simulink model "model"  (R2014a)
(part 4 of 5)

  С_10_С_85_(ПС_«Восточная»___ПС_«Солнечная»___ПС_«Зональная»___ПС_«Солнечная»)_CN_131640871_110000_CN_161501791_110000/RConn3 -- T_161501791_110000_Подстанция_«Коммунальная»/LConn3 -- bus34/LConn1
  T_223481385__Тяговая_ПС/LConn1 -- _CN_223481385_110000_CN_208172439_110000/LConn1
  T_223481385__Тяговая_ПС/LConn2 -- _CN_223481385_110000_CN_208172439_110000/LConn2
  _CN_223481385_110000_CN_208172439_110000/LConn3 -- T_223481385__Тяговая_ПС/LConn3 -- bus35/LConn1
  _CN_223481385_110000_CN_208172439_110000/RConn1 -- T_208172439_110000_Яшкино/LConn1 -- _CN_202917769_110000_CN_208172439_110000/LConn1
  _CN_223481385_110000_CN_208172439_110000/RConn2 -- T_208172439_110000_Яшкино/LConn2 -- _CN_202917769_110000_CN_208172439_110000/LConn2
  _CN_223481385_110000_CN_208172439_110000/RConn3 -- T_208172439_110000_Яшкино/LConn3 -- _CN_202917769_110000_CN_208172439_110000/LConn3 -- bus36/LConn1
  "T_237781034__ПС_110_10_кВ_\"Стрела\""/LConn1 -- _CN_237781034_110000_CN_421135596_110000/LConn1
  "T_237781034__ПС_110_10_кВ_\"Стрела\""/LConn2 -- _CN_237781034_110000_CN_421135596_110000/LConn2
  _CN_237781034_110000_CN_421135596_110000/LConn3 -- "T_237781034__ПС_110_10_кВ_\"Стрела\""/LConn3 -- bus37/LConn1
  "T_421135596_110000;35000;10000_ПС_\"Новоуральская\"_110_35_10"/LConn1 -- _CN_237781034_110000_CN_421135596_110000/RConn1
  "T_421135596_110000;35000;10000_ПС_\"Новоуральская\"_110_35_10"/LConn2 -- _CN_237781034_110000_CN_421135596_110000/RConn2
  _CN_237781034_110000_CN_421135596_110000/RConn3 -- "T_421135596_110000;35000;10000_ПС_\"Новоуральская\"_110_35_10"/LConn3 -- bus38/LConn1
  _CN_228962860_110000_CN_418072303_110000/LConn1 -- T_228962860__/LConn1 -- _CN_228962860_110000_CN_180788791_110000/LConn1
  _CN_228962860_110000_CN_418072303_110000/LConn2 -- T_228962860__/LConn2 -- _CN_228962860_110000_CN_180788791_110000/LConn2
  _CN_228962860_110000_CN_418072303_110000/LConn3 -- T_228962860__/LConn3 -- _CN_228962860_110000_CN_180788791_110000/LConn3 -- bus39/LConn1
  T_418072303__/LConn1 -- _CN_228962860_110000_CN_418072303_110000/RConn1
  T_418072303__/LConn2 -- _CN_228962860_110000_CN_418072303_110000/RConn2
  _CN_228962860_110000_CN_418072303_110000/RConn3 -- T_418072303__/LConn3 -- bus40/LConn1
  _CN_228962860_110000_CN_180788791_110000/RConn1 -- T_180788791__/LConn1 -- _CN_168239171_110000_CN_180788791_110000/LConn1
  _CN_228962860_110000_CN_180788791_110000/RConn2 -- T_180788791__/LConn2 -- _CN_168239171_110000_CN_180788791_110000/LConn2
  _CN_228962860_110000_CN_180788791_110000/RConn3 -- T_180788791__/LConn3 -- _CN_168239171_110000_CN_180788791_110000/LConn3 -- bus41/LConn1
  "T_178541618_110000;6000_ПС_№119_\"Мичуринская\""/LConn1 -- С_201___С_202_CN_178541618_110000_CN_130661477_110000/LConn1
  "T_178541618_110000;6000_ПС_№119_\"Мичуринская\""/LConn2 -- С_201___С_202_CN_178541618_110000_CN_130661477_110000/LConn2
  С_201___С_202_CN_178541618_110000_CN_130661477_110000/LConn3 -- "T_178541618_110000;6000_ПС_№119_\"Мичуринская\""/LConn3 -- bus42/LConn1
  С_201___С_202_CN_178541618_110000_CN_130661477_110000/RConn1 -- G_130661477_Красноярская_ТЭЦ_1/RConn1 -- С_1___С_204_CN_435735618_110000_CN_130661477_110000/RConn1 -- _CN_259523001_110000_CN_130661477_110000/LConn1 -- _CN_259526393_110000_CN_130661477_110000/LConn1
  С_201___С_202_CN_178541618_110000_CN_130661477_110000/RConn2 -- G_130661477_Красноярская_ТЭЦ_1/RConn2 -- С_1___С_204_CN_435735618_110000_CN_130661477_110000/RConn2 -- _CN_259523001_110000_CN_130661477_110000/LConn2 -- _CN_259526393_110000_CN_130661477_110000/LConn2
  С_201___С_202_CN_178541618_110000_CN_130661477_110000/RConn3 -- G_130661477_Красноярская_ТЭЦ_1/RConn3 -- С_1___С_204_CN_435735618_110000_CN_130661477_110000/RConn3 -- _CN_259523001_110000_CN_130661477_110000/LConn3 -- _CN_259526393_110000_CN_130661477_110000/LConn3 -- bus43/LConn1
  T_201587851__/LConn1 -- _CN_201587851_110000_CN_98731668_110000/LConn1
  T_201587851__/LConn2 -- _CN_201587851_110000_CN_98731668_110000/LConn2
  _CN_201587851_110000_CN_98731668_110000/LConn3 -- T_201587851__/LConn3 -- bus44/LConn1
  T_98731668_220000_Подстанция_«Районная»/LConn1 -- _CN_201587851_110000_CN_98731668_110000/RConn1
  T_98731668_220000_Подстанция_«Районная»/LConn2 -- _CN_201587851_110000_CN_98731668_110000/RConn2
  _CN_201587851_110000_CN_98731668_110000/RConn3 -- T_98731668_220000_Подстанция_«Районная»/LConn3 -- bus45/LConn1
  _CN_110796857_110000_CN_184811446_110000/LConn1 -- "T_110796857__ПС_500_220_110_кВ_\"Иркутская\""/RConn1 -- _CN_110796857_110000_CN_184798669_110000/LConn1 -- L_110796857/LConn1
  _CN_110796857_110000_CN_184811446_110000/LConn2 -- "T_110796857__ПС_500_220_110_кВ_\"Иркутская\""/RConn2 -- _CN_110796857_110000_CN_184798669_110000/LConn2 -- L_110796857/LConn2
  _CN_110796857_110000_CN_184811446_110000/LConn3 -- "T_110796857__ПС_500_220_110_кВ_\"Иркутская\""/RConn3 -- _CN_110796857_110000_CN_184798669_110000/LConn3 -- L_110796857/LConn3 -- bus46/LConn1
  T_184811446_110000_ПС_110_35_6_кВ_Прибрежная/LConn1 -- _CN_110796857_110000_CN_184811446_110000/RConn1
  T_184811446_110000_ПС_110_35_6_кВ_Прибрежная/LConn2 -- _CN_110796857_110000_CN_184811446_110000/RConn2
  _CN_110796857_110000_CN_184811446_110000/RConn3 -- T_184811446_110000_ПС_110_35_6_кВ_Прибрежная/LConn3 -- bus47/LConn1
  _CN_110796857_110000_CN_184798669_110000/RConn1 -- T_184798669__ПС_110_35_6_кВ_ГПП_2/LConn1 -- _CN_184798669_110000_CN_297714701_110000/LConn1
  _CN_110796857_110000_CN_184798669_110000/RConn2 -- T_184798669__ПС_110_35_6_кВ_ГПП_2/LConn2 -- _CN_184798669_110000_CN_297714701_110000/LConn2
  _CN_110796857_110000_CN_184798669_110000/RConn3 -- T_184798669__ПС_110_35_6_кВ_ГПП_2/LConn3 -- _CN_184798669_110000_CN_297714701_110000/LConn3 -- bus48/LConn1
  _CN_283922783_110000_CN_202649908_110000/LConn1 -- "T_283922783_110000;10000_ПС_№122_\"Северная\""/LConn1 -- _CN_283922783_110000_CN_95996044_110000/LConn1 -- _CN_283922783_110000_CN_225106390_110000/LConn1 -- _CN_283922783_110000_CN_95614050_110000/LConn1
  _CN_283922783_110000_CN_202649908_110000/LConn2 -- "T_283922783_110000;10000_ПС_№122_\"Северная\""/LConn2 -- _CN_283922783_110000_CN_95996044_110000/LConn2 -- _CN_283922783_110000_CN_225106390_110000/LConn2 -- _CN_283922783_110000_CN_95614050_110000/LConn2
  _CN_283922783_110000_CN_202649908_110000/LConn3 -- "T_283922783_110000;10000_ПС_№122_\"Северная\""/LConn3 -- _CN_283922783_110000_CN_95996044_110000/LConn3 -- _CN_283922783_110000_CN_225106390_110000/LConn3 -- _CN_283922783_110000_CN_95614050_110000/LConn3 -- bus49/LConn1
  _CN_283922783_110000_CN_202649908_110000/RConn1 -- "T_202649908_220000;110000;10000_ПС_\"Октябрьская\""/RConn1 -- С_17___С_18_CN_255772238_110000_CN_202649908_110000/LConn1 -- С_13___С_14_CN_267632930_110000_CN_202649908_110000/LConn1 -- L_202649908/LConn1
  _CN_283922783_110000_CN_202649908_110000/RConn2 -- "T_202649908_220000;110000;10000_ПС_\"Октябрьская\""/RConn2 -- С_17___С_18_CN_255772238_110000_CN_202649908_110000/LConn2 -- С_13___С_14_CN_267632930_110000_CN_202649908_110000/LConn2 -- L_202649908/LConn2
  _CN_283922783_110000_CN_202649908_110000/RConn3 -- "T_202649908_220000;110000;10000_ПС_\"Октябрьская\""/RConn3 -- С_17___С_18_CN_255772238_110000_CN_202649908_110000/LConn3 -- С_13___С_14_CN_267632930_110000_CN_202649908_110000/LConn3 -- L_202649908/LConn3 -- bus50/LConn1
  _CN_283922783_110000_CN_95996044_110000/RConn1 -- "T_95996044_220000;110000;10000_ПС_\"Левобережная\""/RConn1 -- _CN_95996044_110000_CN_289000622_110000/LConn1 -- _CN_95996044_110000_CN_203496562_110000/RConn1 -- L_95996044/LConn1 -- _CN_277861487_110000_CN_95996044_110000/LConn1
  _CN_283922783_110000_CN_95996044_110000/RConn2 -- "T_95996044_220000;110000;10000_ПС_\"Левобережная\""/RConn2 -- _CN_95996044_110000_CN_289000622_110000/LConn2 -- _CN_95996044_110000_CN_203496562_110000/RConn2 -- L_95996044/LConn2 -- _CN_277861487_110000_CN_95996044_110000/LConn2
  _CN_283922783_110000_CN_95996044_110000/RConn3 -- "T_95996044_220000;110000;10000_ПС_\"Левобережная\""/RConn3 -- _CN_95996044_110000_CN_289000622_110000/LConn3 -- _CN_95996044_110000_CN_203496562_110000/RConn3 -- L_95996044/LConn3 -- bus51/LConn1 -- _CN_277861487_110000_CN_95996044_110000/LConn3
  "T_225106390_110000;10000_ПС_№140_\"Аэропорт\""/LConn1 -- _CN_283922783_110000_CN_225106390_110000/RConn1
  "T_225106390_110000;10000_ПС_№140_\"Аэропорт\""/LConn2 -- _CN_283922783_110000_CN_225106390_110000/RConn2
  _CN_283922783_110000_CN_225106390_110000/RConn3 -- "T_225106390_110000;10000_ПС_№140_\"Аэропорт\""/LConn3 -- bus52/LConn1
  T_95614050_110000;10000_/LConn1 -- _CN_283922783_110000_CN_95614050_110000/RConn1
  T_95614050_110000;10000_/LConn2 -- _CN_283922783_110000_CN_95614050_110000/RConn2
  _CN_283922783_110000_CN_95614050_110000/RConn3 -- T_95614050_110000;10000_/LConn3 -- bus53/LConn1
  "T_255519517_110000;6000_ПС_\"Химволокно\""/LConn1 -- С_221___С_222_CN_435735618_110000_CN_255519517_110000/RConn1
  "T_255519517_110000;6000_ПС_\"Химволокно\""/LConn2 -- С_221___С_222_CN_435735618_110000_CN_255519517_110000/RConn2
  С_221___С_222_CN_435735618_110000_CN_255519517_110000/RConn3 -- "T_255519517_110000;6000_ПС_\"Химволокно\""/LConn3 -- bus54/LConn1
  "T_255519515_110000;6000_ПС_\"Цветные_металлы\""/LConn1 -- С_221___С_222_CN_435735618_110000_CN_255519515_110000/RConn1
  "T_255519515_110000;6000_ПС_\"Цветные_металлы\""/LConn2 -- С_221___С_222_CN_435735618_110000_CN_255519515_110000/RConn2
  С_221___С_222_CN_435735618_110000_CN_255519515_110000/RConn3 -- "T_255519515_110000;6000_ПС_\"Цветные_металлы\""/LConn3 -- bus55/LConn1
  "T_258257783_110000;10000_ПС_ГПП_1_\"КрасМаш\""/LConn1 -- С_1___С_204_CN_435735618_110000_CN_258257783_110000/RConn1
  "T_258257783_110000;10000_ПС_ГПП_1_\"КрасМаш\""/LConn2 -- С_1___С_204_CN_435735618_110000_CN_258257783_110000/RConn2
  С_1___С_204_CN_435735618_110000_CN_258257783_110000/RConn3 -- "T_258257783_110000;10000_ПС_ГПП_1_\"КрасМаш\""/LConn3 -- bus56/LConn1
  "T_328318277_110000;10000_ПС_ГПП_2_\"КрасМаш\""/LConn1 -- С_1___С_204_CN_435735618_110000_CN_328318277_110000/RConn1
  "T_328318277_110000;10000_ПС_ГПП_2_\"КрасМаш\""/LConn2 -- С_1___С_204_CN_435735618_110000_CN_328318277_110000/RConn2
  С_1___С_204_CN_435735618_110000_CN_328318277_110000/RConn3 -- "T_328318277_110000;10000_ПС_ГПП_2_\"КрасМаш\""/LConn3 -- bus57/LConn1
  T_255181608_110000_/LConn1 -- _CN_435735618_110000_CN_255181608_110000/RConn1
  T_255181608_110000_/LConn2 -- _CN_435735618_110000_CN_255181608_110000/RConn2
  _CN_435735618_110000_CN_255181608_110000/RConn3 -- T_255181608_110000_/LConn3 -- bus58/LConn1
  _CN_168239171_110000_CN_180788791_110000/RConn1 -- T_168239171_220000_Подстанция_«Ужур»/RConn1 -- L_168239171/LConn1
  _CN_168239171_110000_CN_180788791_110000/RConn2 -- T_168239171_220000_Подстанция_«Ужур»/RConn2 -- L_168239171/LConn2
  _CN_168239171_110000_CN_180788791_110000/RConn3 -- T_168239171_220000_Подстанция_«Ужур»/RConn3 -- L_168239171/LConn3 -- bus59/LConn1
  "T_201620593_110000_Тяговая_ПС_\"Кабаклы\""/LConn1 -- _CN_107439685_110000_CN_201620593_110000/RConn1
  "T_201620593_110000_Тяговая_ПС_\"Кабаклы\""/LConn2 -- _CN_107439685_110000_CN_201620593_110000/RConn2
  _CN_107439685_110000_CN_201620593_110000/RConn3 -- "T_201620593_110000_Тяговая_ПС_\"Кабаклы\""/LConn3 -- bus60/LConn1
  T_197934973_110000_Подстанция_«Валерино»/LConn1 -- _CN_107439685_110000_CN_197934973_110000/RConn1
  T_197934973_110000_Подстанция_«Валерино»/LConn2 -- _CN_107439685_110000_CN_197934973_110000/RConn2
  _CN_107439685_110000_CN_197934973_110000/RConn3 -- T_197934973_110000_Подстанция_«Валерино»/LConn3 -- bus61/LConn1
  T_113306036__/LConn1 -- _CN_107439685_110000_CN_113306036_110000/RConn1
  T_113306036__/LConn2 -- _CN_107439685_110000_CN_113306036_110000/RConn2
  _CN_107439685_110000_CN_113306036_110000/RConn3 -- T_113306036__/LConn3 -- bus62/LConn1
  T_197933918_110000_/LConn1 -- _CN_107439685_110000_CN_197933918_110000/RConn1
  T_197933918_110000_/LConn2 -- _CN_107439685_110000_CN_197933918_110000/RConn2
  _CN_107439685_110000_CN_197933918_110000/RConn3 -- T_197933918_110000_/LConn3 -- bus63/LConn1
  T_201620594_110000_Подстанция_«Киевская»/LConn1 -- _CN_107439685_110000_CN_201620594_110000/RConn1
  T_201620594_110000_Подстанция_«Киевская»/LConn2 -- _CN_107439685_110000_CN_201620594_110000/RConn2
  _CN_107439685_110000_CN_201620594_110000/RConn3 -- T_201620594_110000_Подстанция_«Киевская»/LConn3 -- bus64/LConn1
  С_15_С_16_(ПС_«Левобережная»___ПС_«Мельниково_110»)_CN_167347786_110000_CN_150289682_110000/LConn1 -- T_167347786_110000_Подстанция_«Мельниково»/LConn1 -- С_18_(ПС_«Мельниково»___ПС_«Кожевниково»)_CN_167347786_110000_CN_169673998_110000/LConn1
  С_15_С_16_(ПС_«Левобережная»___ПС_«Мельниково_110»)_CN_167347786_110000_CN_150289682_110000/LConn2 -- T_167347786_110000_Подстанция_«Мельниково»/LConn2 -- С_18_(ПС_«Мельниково»___ПС_«Кожевниково»)_CN_167347786_110000_CN_169673998_110000/LConn2
  С_15_С_16_(ПС_«Левобережная»___ПС_«Мельниково_110»)_CN_167347786_110000_CN_150289682_110000/LConn3 -- T_167347786_110000_Подстанция_«Мельниково»/LConn3 -- С_18_(ПС_«Мельниково»___ПС_«Кожевниково»)_CN_167347786_110000_CN_169673998_110000/LConn3 -- bus65/LConn1
  С_15_С_16_(ПС_«Левобережная»___ПС_«Мельниково_110»)_CN_167347786_110000_CN_150289682_110000/RConn1 -- T_150289682_110000_Подстанция_«Левобережная»/LConn1 -- С_82_С_83_(ПС_«Зональная»___ПС_«Левобережная»)_CN_123874057_110000_CN_150289682_110000/RConn1 -- С_13_С_14_(ПС_«Левобережная»___ПС_«Кандинка_110»)_CN_150289682_110000_CN_169996149_110000/LConn1
  С_15_С_16_(ПС_«Левобережная»___ПС_«Мельниково_110»)_CN_167347786_110000_CN_150289682_110000/RConn2 -- T_150289682_110000_Подстанция_«Левобережная»/LConn2 -- С_82_С_83_(ПС_«Зональная»___ПС_«Левобережная»)_CN_123874057_110000_CN_150289682_110000/RConn2 -- С_13_С_14_(ПС_«Левобережная»___ПС_«Кандинка_110»)_CN_150289682_110000_CN_169996149_110000/LConn2
  С_15_С_16_(ПС_«Левобережная»___ПС_«Мельниково_110»)_CN_167347786_110000_CN_150289682_110000/RConn3 -- T_150289682_110000_Подстанция_«Левобережная»/LConn3 -- С_82_С_83_(ПС_«Зональная»___ПС_«Левобережная»)_CN_123874057_110000_CN_150289682_110000/RConn3 -- С_13_С_14_(ПС_«Левобережная»___ПС_«Кандинка_110»)_CN_150289682_110000_CN_169996149_110000/LConn3 -- bus66/LConn1
  С_18_(ПС_«Мельниково»___ПС_«Кожевниково»)_CN_167347786_110000_CN_169673998_110000/RConn1 -- T_169673998_110000_Подстанция_«Кожевниково»/LConn1 -- С_19_(ПС_«Кожевниково»___ПС_«Уртам»)_CN_169673998_110000_CN_165976042_110000/RConn1
  С_18_(ПС_«Мельниково»___ПС_«Кожевниково»)_CN_167347786_110000_CN_169673998_110000/RConn2 -- T_169673998_110000_Подстанция_«Кожевниково»/LConn2 -- С_19_(ПС_«Кожевниково»___ПС_«Уртам»)_CN_169673998_110000_CN_165976042_110000/RConn2
  С_18_(ПС_«Мельниково»___ПС_«Кожевниково»)_CN_167347786_110000_CN_169673998_110000/RConn3 -- T_169673998_110000_Подстанция_«Кожевниково»/LConn3 -- С_19_(ПС_«Кожевниково»___ПС_«Уртам»)_CN_169673998_110000_CN_165976042_110000/RConn3 -- bus67/LConn1
  С_55_(ПС_«Сайга»___ПС_«Ягодное»)_CN_220695627_110000_CN_202927834_110000/LConn1 -- T_220695627_110000_Подстанция_«Сайга»/LConn1 -- С_55_(ПС_«Сайга»___ПС_«Ягодное»)_CN_220695627_110000_CN_220695628_110000/LConn1
  С_55_(ПС_«Сайга»___ПС_«Ягодное»)_CN_220695627_110000_CN_202927834_110000/LConn2 -- T_220695627_110000_Подстанция_«Сайга»/LConn2 -- С_55_(ПС_«Сайга»___ПС_«Ягодное»)_CN_220695627_110000_CN_220695628_110000/LConn2
  С_55_(ПС_«Сайга»___ПС_«Ягодное»)_CN_220695627_110000_CN_202927834_110000/LConn3 -- T_220695627_110000_Подстанция_«Сайга»/LConn3 -- С_55_(ПС_«Сайга»___ПС_«Ягодное»)_CN_220695627_110000_CN_220695628_110000/LConn3 -- bus68/LConn1
  С_55_(ПС_«Сайга»___ПС_«Ягодное»)_CN_220695627_110000_CN_202927834_110000/RConn1 -- T_202927834_110000_Подстанция_«Белый_Яр»/LConn1 -- С_58_С_59_(ПС_«Белый_Яр»___ПС_«Клюквинка»)_CN_202927834_110000_CN_374528071_110000/LConn1 -- С_57_(ПС_«Белый_Яр»___ПС_«Колпашево»)_CN_170936087_110000_CN_202927834_110000/LConn1
  С_55_(ПС_«Сайга»___ПС_«Ягодное»)_CN_220695627_110000_CN_202927834_110000/RConn2 -- T_202927834_110000_Подстанция_«Белый_Яр»/LConn2 -- С_58_С_59_(ПС_«Белый_Яр»___ПС_«Клюквинка»)_CN_202927834_110000_CN_374528071_110000/LConn2 -- С_57_(ПС_«Белый_Яр»___ПС_«Колпашево»)_CN_170936087_110000_CN_202927834_110000/LConn2
  С_55_(ПС_«Сайга»___ПС_«Ягодное»)_CN_220695627_110000_CN_202927834_110000/RConn3 -- T_202927834_110000_Подстанция_«Белый_Яр»/LConn3 -- С_58_С_59_(ПС_«Белый_Яр»___ПС_«Клюквинка»)_CN_202927834_110000_CN_374528071_110000/LConn3 -- bus69/LConn1 -- С_57_(ПС_«Белый_Яр»___ПС_«Колпашево»)_CN_170936087_110000_CN_202927834_110000/LConn3
  T_220695628_110000_Подстанция_«Ягодное»/LConn1 -- С_55_(ПС_«Сайга»___ПС_«Ягодное»)_CN_220695627_110000_CN_220695628_110000/RConn1
  T_220695628_110000_Подстанция_«Ягодное»/LConn2 -- С_55_(ПС_«Сайга»___ПС_«Ягодное»)_CN_220695627_110000_CN_220695628_110000/RConn2
  С_55_(ПС_«Сайга»___ПС_«Ягодное»)_CN_220695627_110000_CN_220695628_110000/RConn3 -- T_220695628_110000_Подстанция_«Ягодное»/LConn3 -- bus70/LConn1
  _CN_277861487_110000_CN_225106385_110000/LConn1 -- "T_277861487_110000;10000_ПС_№126_\"Радиотехническая\""/LConn1 -- _CN_277861487_110000_CN_277861486_110000/LConn1 -- _CN_277861487_110000_CN_95996044_110000/RConn1
  _CN_277861487_110000_CN_225106385_110000/LConn2 -- "T_277861487_110000;10000_ПС_№126_\"Радиотехническая\""/LConn2 -- _CN_277861487_110000_CN_277861486_110000/LConn2 -- _CN_277861487_110000_CN_95996044_110000/RConn2
  _CN_277861487_110000_CN_225106385_110000/LConn3 -- "T_277861487_110000;10000_ПС_№126_\"Радиотехническая\""/LConn3 -- _CN_277861487_110000_CN_277861486_110000/LConn3 -- _CN_277861487_110000_CN_95996044_110000/RConn3 -- bus71/LConn1
  "T_225106385_110000;35000;10000_ПС_№121_\"Мясокомбинат\""/LConn1 -- _CN_277861487_110000_CN_225106385_110000/RConn1
  "T_225106385_110000;35000;10000_ПС_№121_\"Мясокомбинат\""/LConn2 -- _CN_277861487_110000_CN_225106385_110000/RConn2
  _CN_277861487_110000_CN_225106385_110000/RConn3 -- "T_225106385_110000;35000;10000_ПС_№121_\"Мясокомбинат\""/LConn3 -- bus72/LConn1
  "T_277861486_110000;10000_ПС_№183_\"Ботаническая\""/LConn1 -- _CN_277861487_110000_CN_277861486_110000/RConn1
  "T_277861486_110000;10000_ПС_№183_\"Ботаническая\""/LConn2 -- _CN_277861487_110000_CN_277861486_110000/RConn2
  _CN_277861487_110000_CN_277861486_110000/RConn3 -- "T_277861486_110000;10000_ПС_№183_\"Ботаническая\""/LConn3 -- bus73/LConn1
  С_17___С_18_CN_255772238_110000_CN_259338276_110000/LConn1 -- T_255772238_110000_ПС_БНС_ТЭЦ_2/LConn1 -- С_17___С_18_CN_255772238_110000_CN_202168526_110000/LConn1 -- С_17___С_18_CN_255772238_110000_CN_202649908_110000/RConn1 -- С_17___С_18_CN_255772238_110000_CN_434906029_110000/LConn1 -- С_17___С_18_CN_255772238_110000_CN_258448640_110000/LConn1
  С_17___С_18_CN_255772238_110000_CN_259338276_110000/LConn2 -- T_255772238_110000_ПС_БНС_ТЭЦ_2/LConn2 -- С_17___С_18_CN_255772238_110000_CN_202168526_110000/LConn2 -- С_17___С_18_CN_255772238_110000_CN_202649908_110000/RConn2 -- С_17___С_18_CN_255772238_110000_CN_434906029_110000/LConn2 -- С_17___С_18_CN_255772238_110000_CN_258448640_110000/LConn2
  С_17___С_18_CN_255772238_110000_CN_259338276_110000/LConn3 -- T_255772238_110000_ПС_БНС_ТЭЦ_2/LConn3 -- С_17___С_18_CN_255772238_110000_CN_202168526_110000/LConn3 -- С_17___С_18_CN_255772238_110000_CN_202649908_110000/RConn3 -- С_17___С_18_CN_255772238_110000_CN_434906029_110000/LConn3 -- С_17___С_18_CN_255772238_110000_CN_258448640_110000/LConn3 -- bus74/LConn1
  "T_259338276_110000;6000_ПС_\"Железнодорожная\""/LConn1 -- С_17___С_18_CN_255772238_110000_CN_259338276_110000/RConn1
  "T_259338276_110000;6000_ПС_\"Железнодорожная\""/LConn2 -- С_17___С_18_CN_255772238_110000_CN_259338276_110000/RConn2
  С_17___С_18_CN_255772238_110000_CN_259338276_110000/RConn3 -- "T_259338276_110000;6000_ПС_\"Железнодорожная\""/LConn3 -- bus75/LConn1
  "T_202168526_110000;10000_ПС_№2_\"Советская\""/LConn1 -- С_17___С_18_CN_255772238_110000_CN_202168526_110000/RConn1
  "T_202168526_110000;10000_ПС_№2_\"Советская\""/LConn2 -- С_17___С_18_CN_255772238_110000_CN_202168526_110000/RConn2
  С_17___С_18_CN_255772238_110000_CN_202168526_110000/RConn3 -- "T_202168526_110000;10000_ПС_№2_\"Советская\""/LConn3 -- bus76/LConn1
  "T_434906029_110000_ПС_\"Комбайновый_завод\""/LConn1 -- С_17___С_18_CN_255772238_110000_CN_434906029_110000/RConn1
  "T_434906029_110000_ПС_\"Комбайновый_завод\""/LConn2 -- С_17___С_18_CN_255772238_110000_CN_434906029_110000/RConn2
  С_17___С_18_CN_255772238_110000_CN_434906029_110000/RConn3 -- "T_434906029_110000_ПС_\"Комбайновый_завод\""/LConn3 -- bus77/LConn1
  "T_258448640_110000;6000_ПС_№4_\"Городская\""/LConn1 -- С_17___С_18_CN_255772238_110000_CN_258448640_110000/RConn1
  "T_258448640_110000;6000_ПС_№4_\"Городская\""/LConn2 -- С_17___С_18_CN_255772238_110000_CN_258448640_110000/RConn2
  С_17___С_18_CN_255772238_110000_CN_258448640_110000/RConn3 -- "T_258448640_110000;6000_ПС_№4_\"Городская\""/LConn3 -- bus78/LConn1
  _CN_202917769_110000_CN_170223875_110000/LConn1 -- T_202917769_110000_Подстанция_«Сураново»/LConn1 -- _CN_202917769_110000_CN_162639659_110000/LConn1 -- _CN_202917769_110000_CN_123874057_110000/RConn1 -- _CN_202917769_110000_CN_208172439_110000/RConn1
  _CN_202917769_110000_CN_170223875_110000/LConn2 -- T_202917769_110000_Подстанция_«Сураново»/LConn2 -- _CN_202917769_110000_CN_162639659_110000/LConn2 -- _CN_202917769_110000_CN_123874057_110000/RConn2 -- _CN_202917769_110000_CN_208172439_110000/RConn2
  _CN_202917769_110000_CN_170223875_110000/LConn3 -- T_202917769_110000_Подстанция_«Сураново»/LConn3 -- _CN_202917769_110000_CN_162639659_110000/LConn3 -- _CN_202917769_110000_CN_123874057_110000/RConn3 -- _CN_202917769_110000_CN_208172439_110000/RConn3 -- bus79/LConn1
  T_170223875_110000_Подстанция_«Межениновка»/LConn1 -- _CN_202917769_110000_CN_170223875_110000/RConn1
  T_170223875_110000_Подстанция_«Межениновка»/LConn2 -- _CN_202917769_110000_CN_170223875_110000/RConn2
  _CN_202917769_110000_CN_170223875_110000/RConn3 -- T_170223875_110000_Подстанция_«Межениновка»/LConn3 -- bus80/LConn1
  T_162639659_110000_Подстанция_«71_км»/LConn1 -- _CN_202917769_110000_CN_162639659_110000/RConn1
  T_162639659_110000_Подстанция_«71_км»/LConn2 -- _CN_202917769_110000_CN_162639659_110000/RConn2
  _CN_202917769_110000_CN_162639659_110000/RConn3 -- T_162639659_110000_Подстанция_«71_км»/LConn3 -- bus81/LConn1
  _CN_208031316_110000_CN_221735143_110000/LConn1 -- T_208031316__/LConn1 -- _CN_208031316_110000_CN_210955238_110000/LConn1
  _CN_208031316_110000_CN_221735143_110000/LConn2 -- T_208031316__/LConn2 -- _CN_208031316_110000_CN_210955238_110000/LConn2
  _CN_208031316_110000_CN_221735143_110000/LConn3 -- T_208031316__/LConn3 -- _CN_208031316_110000_CN_210955238_110000/LConn3 -- bus82/LConn1
  T_221735143__/LConn1 -- _CN_208031316_110000_CN_221735143_110000/RConn1
  T_221735143__/LConn2 -- _CN_208031316_110000_CN_221735143_110000/RConn2
  _CN_208031316_110000_CN_221735143_110000/RConn3 -- T_221735143__/LConn3 -- bus83/LConn1
  _CN_208031316_110000_CN_210955238_110000/RConn1 -- T_210955238__/LConn1 -- _CN_126390946_110000_CN_210955238_110000/LConn1
  _CN_208031316_110000_CN_210955238_110000/RConn2 -- T_210955238__/LConn2 -- _CN_126390946_110000_CN_210955238_110000/LConn2
  _CN_208031316_110000_CN_210955238_110000/RConn3 -- T_210955238__/LConn3 -- _CN_126390946_110000_CN_210955238_110000/LConn3 -- bus84/LConn1
  _CN_259523001_110000_CN_130661477_110000/RConn1 -- "T_259523001_110000;6000_ПС_№25_\"РТИ\""/LConn1 -- _CN_259523001_110000_CN_255181607_110000/LConn1 -- _CN_259523001_110000_CN_106887628_110000/LConn1 -- _CN_259523001_110000_CN_254770727_110000/LConn1
  _CN_259523001_110000_CN_130661477_110000/RConn2 -- "T_259523001_110000;6000_ПС_№25_\"РТИ\""/LConn2 -- _CN_259523001_110000_CN_255181607_110000/LConn2 -- _CN_259523001_110000_CN_106887628_110000/LConn2 -- _CN_259523001_110000_CN_254770727_110000/LConn2
  _CN_259523001_110000_CN_130661477_110000/RConn3 -- "T_259523001_110000;6000_ПС_№25_\"РТИ\""/LConn3 -- _CN_259523001_110000_CN_255181607_110000/LConn3 -- _CN_259523001_110000_CN_106887628_110000/LConn3 -- _CN_259523001_110000_CN_254770727_110000/LConn3 -- bus85/LConn1
  T_255181607_110000_/LConn1 -- _CN_259523001_110000_CN_255181607_110000/RConn1
  T_255181607_110000_/LConn2 -- _CN_259523001_110000_CN_255181607_110000/RConn2
  _CN_259523001_110000_CN_255181607_110000/RConn3 -- T_255181607_110000_/LConn3 -- bus86/LConn1
  _CN_259523001_110000_CN_106887628_110000/RConn1 -- G_106887628_Красноярская_ТЭЦ_2/RConn1 -- С_13___С_14_CN_267632930_110000_CN_106887628_110000/LConn1
  _CN_259523001_110000_CN_106887628_110000/RConn2 -- G_106887628_Красноярская_ТЭЦ_2/RConn2 -- С_13___С_14_CN_267632930_110000_CN_106887628_110000/LConn2
  _CN_259523001_110000_CN_106887628_110000/RConn3 -- G_106887628_Красноярская_ТЭЦ_2/RConn3 -- С_13___С_14_CN_267632930_110000_CN_106887628_110000/LConn3 -- bus87/LConn1
  "T_254770727_110000;6000_ПС_№8_\"Цемзавод\""/LConn1 -- _CN_259523001_110000_CN_254770727_110000/RConn1
  "T_254770727_110000;6000_ПС_№8_\"Цемзавод\""/LConn2 -- _CN_259523001_110000_CN_254770727_110000/RConn2
  _CN_259523001_110000_CN_254770727_110000/RConn3 -- "T_254770727_110000;6000_ПС_№8_\"Цемзавод\""/LConn3 -- bus88/LConn1
  "T_259526393_110000_ПС_№24_\"ЦБК\""/LConn1 -- _CN_259526393_110000_CN_130661477_110000/RConn1
  "T_259526393_110000_ПС_№24_\"ЦБК\""/LConn2 -- _CN_259526393_110000_CN_130661477_110000/RConn2
  _CN_259526393_110000_CN_130661477_110000/RConn3 -- "T_259526393_110000_ПС_№24_\"ЦБК\""/LConn3 -- bus89/LConn1
  T_272521315__/LConn1 -- _CN_272521315_110000_CN_267191160_110000/LConn1
  T_272521315__/LConn2 -- _CN_272521315_110000_CN_267191160_110000/LConn2
  _CN_272521315_110000_CN_267191160_110000/LConn3 -- T_272521315__/LConn3 -- bus90/LConn1
  _CN_272521315_110000_CN_267191160_110000/RConn1 -- T_267191160_220000;110000;10000_/RConn1 -- L_267191160/LConn1
  _CN_272521315_110000_CN_267191160_110000/RConn2 -- T_267191160_220000;110000;10000_/RConn2 -- L_267191160/LConn2
  _CN_272521315_110000_CN_267191160_110000/RConn3 -- T_267191160_220000;110000;10000_/RConn3 -- L_267191160/LConn3 -- bus91/LConn1
  T_170766446__/LConn1 -- _CN_170766446_110000_CN_170766539_110000/LConn1
  T_170766446__/LConn2 -- _CN_170766446_110000_CN_170766539_110000/LConn2
  _CN_170766446_110000_CN_170766539_110000/LConn3 -- T_170766446__/LConn3 -- bus92/LConn1
  T_170766539__/LConn1 -- _CN_170766446_110000_CN_170766539_110000/RConn1
  T_170766539__/LConn2 -- _CN_170766446_110000_CN_170766539_110000/RConn2
  _CN_170766446_110000_CN_170766539_110000/RConn3 -- T_170766539__/LConn3 -- bus93/LConn1
  T_141629072__/LConn1 -- _CN_141629044_110000_CN_141629072_110000/RConn1
  T_141629072__/LConn2 -- _CN_141629044_110000_CN_141629072_110000/RConn2
  _CN_141629044_110000_CN_141629072_110000/RConn3 -- T_141629072__/LConn3 -- bus94/LConn1
  T_256577270__/LConn1 -- _CN_141629044_110000_CN_256577270_110000/RConn1
  T_256577270__/LConn2 -- _CN_141629044_110000_CN_256577270_110000/RConn2
  _CN_141629044_110000_CN_256577270_110000/RConn3 -- T_256577270__/LConn3 -- bus95/LConn1
  T_227657047__/LConn1 -- _CN_141629044_110000_CN_227657047_110000/RConn1
  T_227657047__/LConn2 -- _CN_141629044_110000_CN_227657047_110000/RConn2
  _CN_141629044_110000_CN_227657047_110000/RConn3 -- T_227657047__/LConn3 -- bus96/LConn1
  С_75_С_76_(ПС_«Малиновка»___ПС_«Турунтаево»)_CN_97113720_110000_CN_181309204_110000/LConn1 -- T_97113720_110000_Подстанция_«Малиновка»/LConn1 -- С_7Б_(ПС_«Бройлерная»___ПС_«Малиновка»)_CN_97113720_110000_CN_125746756_110000/LConn1 -- С_7М_(ПС_«Малиновка»___ПС_«Итатка»);?_(ПС_«Малиновка»___ПС_«Асино_220»)_CN_97113720_110000_CN_97113734_110000/LConn1
  С_75_С_76_(ПС_«Малиновка»___ПС_«Турунтаево»)_CN_97113720_110000_CN_181309204_110000/LConn2 -- T_97113720_110000_Подстанция_«Малиновка»/LConn2 -- С_7Б_(ПС_«Бройлерная»___ПС_«Малиновка»)_CN_97113720_110000_CN_125746756_110000/LConn2 -- С_7М_(ПС_«Малиновка»___ПС_«Итатка»);?_(ПС_«Малиновка»___ПС_«Асино_220»)_CN_97113720_110000_CN_97113734_110000/LConn2
  С_75_С_76_(ПС_«Малиновка»___ПС_«Турунтаево»)_CN_97113720_110000_CN_181309204_110000/LConn3 -- T_97113720_110000_Подстанция_«Малиновка»/LConn3 -- С_7Б_(ПС_«Бройлерная»___ПС_«Малиновка»)_CN_97113720_110000_CN_125746756_110000/LConn3 -- С_7М_(ПС_«Малиновка»___ПС_«Итатка»);?_(ПС_«Малиновка»___ПС_«Асино_220»)_CN_97113720_110000_CN_97113734_110000/LConn3 -- bus97/LConn1
  T_181309204_110000_Подстанция_«Турунтаево»/LConn1 -- С_75_С_76_(ПС_«Малиновка»___ПС_«Турунтаево»)_CN_97113720_110000_CN_181309204_110000/RConn1
  T_181309204_110000_Подстанция_«Турунтаево»/LConn2 -- С_75_С_76_(ПС_«Малиновка»___ПС_«Турунтаево»)_CN_97113720_110000_CN_181309204_110000/RConn2
  С_75_С_76_(ПС_«Малиновка»___ПС_«Турунтаево»)_CN_97113720_110000_CN_181309204_110000/RConn3 -- T_181309204_110000_Подстанция_«Турунтаево»/LConn3 -- bus98/LConn1
  С_7Б_(ПС_«Бройлерная»___ПС_«Малиновка»)_CN_97113720_110000_CN_125746756_110000/RConn1 -- T_125746756_110000_Подстанция_«Бройлерная»/LConn1 -- C_107_С_108_(ПС_«Восточная»___ПС_«Бройлерная»)_CN_77195444_110000_CN_125746756_110000/RConn1
  С_7Б_(ПС_«Бройлерная»___ПС_«Малиновка»)_CN_97113720_110000_CN_125746756_110000/RConn2 -- T_125746756_110000_Подстанция_«Бройлерная»/LConn2 -- C_107_С_108_(ПС_«Восточная»___ПС_«Бройлерная»)_CN_77195444_110000_CN_125746756_110000/RConn2
  С_7Б_(ПС_«Бройлерная»___ПС_«Малиновка»)_CN_97113720_110000_CN_125746756_110000/RConn3 -- T_125746756_110000_Подстанция_«Бройлерная»/LConn3 -- C_107_С_108_(ПС_«Восточная»___ПС_«Бройлерная»)_CN_77195444_110000_CN_125746756_110000/RConn3 -- bus99/LConn1
  С_7М_(ПС_«Малиновка»___ПС_«Итатка»);?_(ПС_«Малиновка»___ПС_«Асино_220»)_CN_97113720_110000_CN_97113734_110000/RConn1 -- T_97113734_110000_Подстанция_«Итатка»/LConn1 -- С_7а_(ПС_«Итатка»___ПС_«Асино_110»)_CN_97113734_110000_CN_169734094_110000/LConn1
  С_7М_(ПС_«Малиновка»___ПС_«Итатка»);?_(ПС_«Малиновка»___ПС_«Асино_220»)_CN_97113720_110000_CN_97113734_110000/RConn2 -- T_97113734_110000_Подстанция_«Итатка»/LConn2 -- С_7а_(ПС_«Итатка»___ПС_«Асино_110»)_CN_97113734_110000_CN_169734094_110000/LConn2
  С_7М_(ПС_«Малиновка»___ПС_«Итатка»);?_(ПС_«Малиновка»___ПС_«Асино_220»)_CN_97113720_110000_CN_97113734_110000/RConn3 -- T_97113734_110000_Подстанция_«Итатка»/LConn3 -- С_7а_(ПС_«Итатка»___ПС_«Асино_110»)_CN_97113734_110000_CN_169734094_110000/LConn3 -- bus100/LConn1
  С_102_(С_101?)_(ПС_«Парабель»___ПС_«Парабель_КС»)_CN_167241850_110000_CN_171057519_110000/LConn1 -- T_167241850_220000_Подстанция_«Парабель»/RConn1 -- С_103_С_104_(ПС_«Парабель»___ПС_«Лугинецкая»)_CN_167241850_110000_CN_197782305_110000/LConn1 -- L_167241850/LConn1
  С_102_(С_101?)_(ПС_«Парабель»___ПС_«Парабель_КС»)_CN_167241850_110000_CN_171057519_110000/LConn2 -- T_167241850_220000_Подстанция_«Парабель»/RConn2 -- С_103_С_104_(ПС_«Парабель»___ПС_«Лугинецкая»)_CN_167241850_110000_CN_197782305_110000/LConn2 -- L_167241850/LConn2
  С_102_(С_101?)_(ПС_«Парабель»___ПС_«Парабель_КС»)_CN_167241850_110000_CN_171057519_110000/LConn3 -- T_167241850_220000_Подстанция_«Парабель»/RConn3 -- С_103_С_104_(ПС_«Парабель»___ПС_«Лугинецкая»)_CN_167241850_110000_CN_197782305_110000/LConn3 -- L_167241850/LConn3 -- bus101/LConn1
  T_171057519_110000_Подстанция_«Парабель_КС»/LConn1 -- С_102_(С_101?)_(ПС_«Парабель»___ПС_«Парабель_КС»)_CN_167241850_110000_CN_171057519_110000/RConn1
  T_171057519_110000_Подстанция_«Парабель_КС»/LConn2 -- С_102_(С_101?)_(ПС_«Парабель»___ПС_«Парабель_КС»)_CN_167241850_110000_CN_171057519_110000/RConn2
  С_102_(С_101?)_(ПС_«Парабель»___ПС_«Парабель_КС»)_CN_167241850_110000_CN_171057519_110000/RConn3 -- T_171057519_110000_Подстанция_«Парабель_КС»/LConn3 -- bus102/LConn1
  С_103_С_104_(ПС_«Парабель»___ПС_«Лугинецкая»)_CN_167241850_110000_CN_197782305_110000/RConn1 -- T_197782305_110000_Подстанция_«Лугинецкая»/LConn1 -- С_109_(С_110?)_(ПС_«Лугинецкая»___ПС_«Игольская»)_CN_197782305_110000_CN_195060971_110000/LConn1 -- С_105_106_(ПС_«Лугинецкая»___ПС_«Калиновая»)_CN_194903352_110000_CN_197782305_110000/LConn1
  С_103_С_104_(ПС_«Парабель»___ПС_«Лугинецкая»)_CN_167241850_110000_CN_197782305_110000/RConn2 -- T_197782305_110000_Подстанция_«Лугинецкая»/LConn2 -- С_109_(С_110?)_(ПС_«Лугинецкая»___ПС_«Игольская»)_CN_197782305_110000_CN_195060971_110000/LConn2 -- С_105_106_(ПС_«Лугинецкая»___ПС_«Калиновая»)_CN_194903352_110000_CN_197782305_110000/LConn2
  С_103_С_104_(ПС_«Парабель»___ПС_«Лугинецкая»)_CN_167241850_110000_CN_197782305_110000/RConn3 -- T_197782305_110000_Подстанция_«Лугинецкая»/LConn3 -- С_109_(С_110?)_(ПС_«Лугинецкая»___ПС_«Игольская»)_CN_197782305_110000_CN_195060971_110000/LConn3 -- bus103/LConn1 -- С_105_106_(ПС_«Лугинецкая»___ПС_«Калиновая»)_CN_194903352_110000_CN_197782305_110000/LConn3
  С_7а_(ПС_«Итатка»___ПС_«Асино_110»)_CN_97113734_110000_CN_169734094_110000/RConn1 -- T_169734094_110000_Подстанция_«Асино_110»/LConn1 -- С_61_С_62_(ПС_«Асино_110»___ПС_«Зырянка»)_CN_169734094_110000_CN_245392698_110000/LConn1 -- С_61_С_62_(ПС_«Асино_110»___ПС_«Зырянка»)_CN_169734094_110000_CN_243298567_110000/LConn1
  С_7а_(ПС_«Итатка»___ПС_«Асино_110»)_CN_97113734_110000_CN_169734094_110000/RConn2 -- T_169734094_110000_Подстанция_«Асино_110»/LConn2 -- С_61_С_62_(ПС_«Асино_110»___ПС_«Зырянка»)_CN_169734094_110000_CN_245392698_110000/LConn2 -- С_61_С_62_(ПС_«Асино_110»___ПС_«Зырянка»)_CN_169734094_110000_CN_243298567_110000/LConn2
  С_7а_(ПС_«Итатка»___ПС_«Асино_110»)_CN_97113734_110000_CN_169734094_110000/RConn3 -- T_169734094_110000_Подстанция_«Асино_110»/LConn3 -- С_61_С_62_(ПС_«Асино_110»___ПС_«Зырянка»)_CN_169734094_110000_CN_245392698_110000/LConn3 -- С_61_С_62_(ПС_«Асино_110»___ПС_«Зырянка»)_CN_169734094_110000_CN_243298567_110000/LConn3 -- bus104/LConn1
  T_145227914__Подстанция_«Учительская»/LConn1 -- _CN_145227914_110000_CN_51844718_110000/LConn1
  T_145227914__Подстанция_«Учительская»/LConn2 -- _CN_145227914_110000_CN_51844718_110000/LConn2
  _CN_145227914_110000_CN_51844718_110000/LConn3 -- T_145227914__Подстанция_«Учительская»/LConn3 -- bus105/LConn1
  G_51844718_ТЭЦ_№4/RConn1 -- _CN_145227914_110000_CN_51844718_110000/RConn1
  G_51844718_ТЭЦ_№4/RConn2 -- _CN_145227914_110000_CN_51844718_110000/RConn2
  _CN_145227914_110000_CN_51844718_110000/RConn3 -- G_51844718_ТЭЦ_№4/RConn3 -- bus106/LConn1
  С_40_(ПС_«Чажемто»___ПС_«Колпашево»)_CN_170936087_110000_CN_169356997_110000/LConn1 -- T_170936087_110000_Подстанция_«Колпашево»/LConn1 -- С_57_(ПС_«Белый_Яр»___ПС_«Колпашево»)_CN_170936087_110000_CN_202927834_110000/RConn1
  С_40_(ПС_«Чажемто»___ПС_«Колпашево»)_CN_170936087_110000_CN_169356997_110000/LConn2 -- T_170936087_110000_Подстанция_«Колпашево»/LConn2 -- С_57_(ПС_«Белый_Яр»___ПС_«Колпашево»)_CN_170936087_110000_CN_202927834_110000/RConn2
  С_40_(ПС_«Чажемто»___ПС_«Колпашево»)_CN_170936087_110000_CN_169356997_110000/LConn3 -- T_170936087_110000_Подстанция_«Колпашево»/LConn3 -- С_57_(ПС_«Белый_Яр»___ПС_«Колпашево»)_CN_170936087_110000_CN_202927834_110000/RConn3 -- bus107/LConn1
  С_40_(ПС_«Чажемто»___ПС_«Колпашево»)_CN_170936087_110000_CN_169356997_110000/RConn1 -- T_169356997_220000_Подстанция_«Чажемто_220»/RConn1 -- С_111_(С_112?)_(ПС_«Чажемто_220»___ПС_«Первомайская»_консерв)_CN_169356997_110000_CN_316964474_110000/LConn1 -- С_28_С_38_(ПС_«Чажемто»___ПС_«Коломинские_Гривы»)_CN_169356997_110000_CN_191567780_110000/LConn1 -- С_29_С_39_(ПС_«Чажемто_220»___ПС_«Чажемто_110»)_CN_169356997_110000_CN_169700760_110000/LConn1 -- L_169356997/LConn1
  С_40_(ПС_«Чажемто»___ПС_«Колпашево»)_CN_170936087_110000_CN_169356997_110000/RConn2 -- T_169356997_220000_Подстанция_«Чажемто_220»/RConn2 -- С_111_(С_112?)_(ПС_«Чажемто_220»___ПС_«Первомайская»_консерв)_CN_169356997_110000_CN_316964474_110000/LConn2 -- С_28_С_38_(ПС_«Чажемто»___ПС_«Коломинские_Гривы»)_CN_169356997_110000_CN_191567780_110000/LConn2 -- С_29_С_39_(ПС_«Чажемто_220»___ПС_«Чажемто_110»)_CN_169356997_110000_CN_169700760_110000/LConn2 -- L_169356997/LConn2
  С_40_(ПС_«Чажемто»___ПС_«Колпашево»)_CN_170936087_110000_CN_169356997_110000/RConn3 -- T_169356997_220000_Подстанция_«Чажемто_220»/RConn3 -- С_111_(С_112?)_(ПС_«Чажемто_220»___ПС_«Первомайская»_консерв)_CN_169356997_110000_CN_316964474_110000/LConn3 -- С_28_С_38_(ПС_«Чажемто»___ПС_«Коломинские_Гривы»)_CN_169356997_110000_CN_191567780_110000/LConn3 -- С_29_С_39_(ПС_«Чажемто_220»___ПС_«Чажемто_110»)_CN_169356997_110000_CN_169700760_110000/LConn3 -- L_169356997/LConn3 -- bus108/LConn1
  "T_289000622_110000;10000_ПC_№16_\"Пролетарская\""/LConn1 -- _CN_95996044_110000_CN_289000622_110000/RConn1
  "T_289000622_110000;10000_ПC_№16_\"Пролетарская\""/LConn2 -- _CN_95996044_110000_CN_289000622_110000/RConn2
  _CN_95996044_110000_CN_289000622_110000/RConn3 -- "T_289000622_110000;10000_ПC_№16_\"Пролетарская\""/LConn3 -- bus109/LConn1
  T_173502610_110000_Подстанция_«Усть_Бакчар»/LConn1 -- С_46_С_47_(ПС_«Высокий_Яр»___ПС_«Усть_Бакчар»___ПС_«Подгорное»___ПС_«Усть_Бакчар»)_CN_173502610_110000_CN_170480403_110000/LConn1
  T_173502610_110000_Подстанция_«Усть_Бакчар»/LConn2 -- С_46_С_47_(ПС_«Высокий_Яр»___ПС_«Усть_Бакчар»___ПС_«Подгорное»___ПС_«Усть_Бакчар»)_CN_173502610_110000_CN_170480403_110000/LConn2
  С_46_С_47_(ПС_«Высокий_Яр»___ПС_«Усть_Бакчар»___ПС_«Подгорное»___ПС_«Усть_Бакчар»)_CN_173502610_110000_CN_170480403_110000/LConn3 -- T_173502610_110000_Подстанция_«Усть_Бакчар»/LConn3 -- bus110/LConn1
  T_170480403_110000_Подстанция_«Высокий_Яр»/LConn1 -- С_46_С_47_(ПС_«Высокий_Яр»___ПС_«Усть_Бакчар»___ПС_«Подгорное»___ПС_«Усть_Бакчар»)_CN_173502610_110000_CN_170480403_110000/RConn1
  T_170480403_110000_Подстанция_«Высокий_Яр»/LConn2 -- С_46_С_47_(ПС_«Высокий_Яр»___ПС_«Усть_Бакчар»___ПС_«Подгорное»___ПС_«Усть_Бакчар»)_CN_173502610_110000_CN_170480403_110000/RConn2
  С_46_С_47_(ПС_«Высокий_Яр»___ПС_«Усть_Бакчар»___ПС_«Подгорное»___ПС_«Усть_Бакчар»)_CN_173502610_110000_CN_170480403_110000/RConn3 -- T_170480403_110000_Подстанция_«Высокий_Яр»/LConn3 -- bus111/LConn1
  С_25_С_26_(ПС_«Кривошеино»___ПС_«Молчаново»___ПС_«Молчаново»___ПС_«Коломинские_Гривы»)_CN_169815706_110000_CN_191567780_110000/LConn1 -- T_169815706_110000_Подстанция_«Молчаново»/LConn1 -- С_25_С_26_(ПС_«Кривошеино»___ПС_«Молчаново»___ПС_«Молчаново»___ПС_«Коломинские_Гривы»)_CN_169815706_110000_CN_189871845_110000/LConn1 -- С_25_С_26_(ПС_«Кривошеино»___ПС_«Молчаново»___ПС_«Молчаново»___ПС_«Коломинские_Гривы»)_CN_169815706_110000_CN_190434443_110000/RConn1 -- С_25_С_26_(ПС_«Кривошеино»___ПС_«Молчаново»___ПС_«Молчаново»___ПС_«Коломинские_Гривы»)_CN_169815706_110000_CN_172669169_110000/LConn1 -- С_25_С_26_(ПС_«Кривошеино»___ПС_«Молчаново»___ПС_«Молчаново»___ПС_«Коломинские_Гривы»)_CN_169815706_110000_CN_172669881_110000/LConn1
  С_25_С_26_(ПС_«Кривошеино»___ПС_«Молчаново»___ПС_«Молчаново»___ПС_«Коломинские_Гривы»)_CN_169815706_110000_CN_191567780_110000/LConn2 -- T_169815706_110000_Подстанция_«Молчаново»/LConn2 -- С_25_С_26_(ПС_«Кривошеино»___ПС_«Молчаново»___ПС_«Молчаново»___ПС_«Коломинские_Гривы»)_CN_169815706_110000_CN_189871845_110000/LConn2 -- С_25_С_26_(ПС_«Кривошеино»___ПС_«Молчаново»___ПС_«Молчаново»___ПС_«Коломинские_Гривы»)_CN_169815706_110000_CN_190434443_110000/RConn2 -- С_25_С_26_(ПС_«Кривошеино»___ПС_«Молчаново»___ПС_«Молчаново»___ПС_«Коломинские_Гривы»)_CN_169815706_110000_CN_172669169_110000/LConn2 -- С_25_С_26_(ПС_«Кривошеино»___ПС_«Молчаново»___ПС_«Молчаново»___ПС_«Коломинские_Гривы»)_CN_169815706_110000_CN_172669881_110000/LConn2
  С_25_С_26_(ПС_«Кривошеино»___ПС_«Молчаново»___ПС_«Молчаново»___ПС_«Коломинские_Гривы»)_CN_169815706_110000_CN_191567780_110000/LConn3 -- T_169815706_110000_Подстанция_«Молчаново»/LConn3 -- С_25_С_26_(ПС_«Кривошеино»___ПС_«Молчаново»___ПС_«Молчаново»___ПС_«Коломинские_Гривы»)_CN_169815706_110000_CN_189871845_110000/LConn3 -- С_25_С_26_(ПС_«Кривошеино»___ПС_«Молчаново»___ПС_«Молчаново»___ПС_«Коломинские_Гривы»)_CN_169815706_110000_CN_190434443_110000/RConn3 -- С_25_С_26_(ПС_«Кривошеино»___ПС_«Молчаново»___ПС_«Молчаново»___ПС_«Коломинские_Гривы»)_CN_169815706_110000_CN_172669169_110000/LConn3 -- С_25_С_26_(ПС_«Кривошеино»___ПС_«Молчаново»___ПС_«Молчаново»___ПС_«Коломинские_Гривы»)_CN_169815706_110000_CN_172669881_110000/LConn3 -- bus112/LConn1
  С_25_С_26_(ПС_«Кривошеино»___ПС_«Молчаново»___ПС_«Молчаново»___ПС_«Коломинские_Гривы»)_CN_169815706_110000_CN_191567780_110000/RConn1 -- T_191567780_110000_Подстанция_«Коломинские_Гривы»/LConn1 -- С_28_С_38_(ПС_«Чажемто»___ПС_«Коломинские_Гривы»)_CN_169356997_110000_CN_191567780_110000/RConn1
  С_25_С_26_(ПС_«Кривошеино»___ПС_«Молчаново»___ПС_«Молчаново»___ПС_«Коломинские_Гривы»)_CN_169815706_110000_CN_191567780_110000/RConn2 -- T_191567780_110000_Подстанция_«Коломинские_Гривы»/LConn2 -- С_28_С_38_(ПС_«Чажемто»___ПС_«Коломинские_Гривы»)_CN_169356997_110000_CN_191567780_110000/RConn2
  С_25_С_26_(ПС_«Кривошеино»___ПС_«Молчаново»___ПС_«Молчаново»___ПС_«Коломинские_Гривы»)_CN_169815706_110000_CN_191567780_110000/RConn3 -- T_191567780_110000_Подстанция_«Коломинские_Гривы»/LConn3 -- С_28_С_38_(ПС_«Чажемто»___ПС_«Коломинские_Гривы»)_CN_169356997_110000_CN_191567780_110000/RConn3 -- bus113/LConn1
  С_25_С_26_(ПС_«Кривошеино»___ПС_«Молчаново»___ПС_«Молчаново»___ПС_«Коломинские_Гривы»)_CN_169815706_110000_CN_189871845_110000/RConn1 -- T_189871845_220000_Подстанция_«Володино_220»/RConn1 -- С_22_С_32_(ПС_«Мельниково_220»___ПС_«Володино_220»)_CN_189871845_110000_CN_169671124_110000/LConn1 -- L_189871845/LConn1
  С_25_С_26_(ПС_«Кривошеино»___ПС_«Молчаново»___ПС_«Молчаново»___ПС_«Коломинские_Гривы»)_CN_169815706_110000_CN_189871845_110000/RConn2 -- T_189871845_220000_Подстанция_«Володино_220»/RConn2 -- С_22_С_32_(ПС_«Мельниково_220»___ПС_«Володино_220»)_CN_189871845_110000_CN_169671124_110000/LConn2 -- L_189871845/LConn2
  С_25_С_26_(ПС_«Кривошеино»___ПС_«Молчаново»___ПС_«Молчаново»___ПС_«Коломинские_Гривы»)_CN_169815706_110000_CN_189871845_110000/RConn3 -- T_189871845_220000_Подстанция_«Володино_220»/RConn3 -- С_22_С_32_(ПС_«Мельниково_220»___ПС_«Володино_220»)_CN_189871845_110000_CN_169671124_110000/LConn3 -- L_189871845/LConn3 -- bus114/LConn1
  T_172669169_110000_Подстанция_«Молчановская_НПС»/LConn1 -- С_25_С_26_(ПС_«Кривошеино»___ПС_«Молчаново»___ПС_«Молчаново»___ПС_«Коломинские_Гривы»)_CN_169815706_110000_CN_172669169_110000/RConn1
  T_172669169_110000_Подстанция_«Молчановская_НПС»/LConn2 -- С_25_С_26_(ПС_«Кривошеино»___ПС_«Молчаново»___ПС_«Молчаново»___ПС_«Коломинские_Гривы»)_CN_169815706_110000_CN_172669169_110000/RConn2
  С_25_С_26_(ПС_«Кривошеино»___ПС_«Молчаново»___ПС_«Молчаново»___ПС_«Коломинские_Гривы»)_CN_169815706_110000_CN_172669169_110000/RConn3 -- T_172669169_110000_Подстанция_«Молчановская_НПС»/LConn3 -- bus115/LConn1
  T_172669881_110000_Подстанция_«Тунгусово»/LConn1 -- С_25_С_26_(ПС_«Кривошеино»___ПС_«Молчаново»___ПС_«Молчаново»___ПС_«Коломинские_Гривы»)_CN_169815706_110000_CN_172669881_110000/RConn1
  T_172669881_110000_Подстанция_«Тунгусово»/LConn2 -- С_25_С_26_(ПС_«Кривошеино»___ПС_«Молчаново»___ПС_«Молчаново»___ПС_«Коломинские_Гривы»)_CN_169815706_110000_CN_172669881_110000/RConn2
  С_25_С_26_(ПС_«Кривошеино»___ПС_«Молчаново»___ПС_«Молчаново»___ПС_«Коломинские_Гривы»)_CN_169815706_110000_CN_172669881_110000/RConn3 -- T_172669881_110000_Подстанция_«Тунгусово»/LConn3 -- bus116/LConn1
  T_198009967__/LConn1 -- _CN_198009967_110000_CN_198008863_110000/LConn1
  T_198009967__/LConn2 -- _CN_198009967_110000_CN_198008863_110000/LConn2
  _CN_198009967_110000_CN_198008863_110000/LConn3 -- T_198009967__/LConn3 -- bus117/LConn1
  T_198008863__/LConn1 -- _CN_198009967_110000_CN_198008863_110000/RConn1
  T_198008863__/LConn2 -- _CN_198009967_110000_CN_198008863_110000/RConn2
  _CN_198009967_110000_CN_198008863_110000/RConn3 -- T_198008863__/LConn3 -- bus118/LConn1
  "T_126390946__ПС_\"Сыропятское\""/LConn1 -- _CN_126390946_110000_CN_210955238_110000/RConn1
  "T_126390946__ПС_\"Сыропятское\""/LConn2 -- _CN_126390946_110000_CN_210955238_110000/RConn2
  _CN_126390946_110000_CN_210955238_110000/RConn3 -- "T_126390946__ПС_\"Сыропятское\""/LConn3 -- bus119/LConn1
  "T_230915624__Тяговая_подстанция_\"Чугунаш\""/LConn1 -- "ВЛ_110_Чугунаш___ПС_\"Кондомская\"_CN_230915624_110000_CN_225625506_110000"/LConn1
  "T_230915624__Тяговая_подстанция_\"Чугунаш\""/LConn2 -- "ВЛ_110_Чугунаш___ПС_\"Кондомская\"_CN_230915624_110000_CN_225625506_110000"/LConn2
  "ВЛ_110_Чугунаш___ПС_\"Кондомская\"_CN_230915624_110000_CN_225625506_110000"/LConn3 -- "T_230915624__Тяговая_подстанция_\"Чугунаш\""/LConn3 -- bus120/LConn1
  "T_225625506_110000;35000;6000_ПС_110_35_6_кВ_\"Кондомская\""/LConn1 -- "ВЛ_110_Чугунаш___ПС_\"Кондомская\"_CN_230915624_110000_CN_225625506_110000"/RConn1
  "T_225625506_110000;35000;6000_ПС_110_35_6_кВ_\"Кондомская\""/LConn2 -- "ВЛ_110_Чугунаш___ПС_\"Кондомская\"_CN_230915624_110000_CN_225625506_110000"/RConn2
  "ВЛ_110_Чугунаш___ПС_\"Кондомская\"_CN_230915624_110000_CN_225625506_110000"/RConn3 -- "T_225625506_110000;35000;6000_ПС_110_35_6_кВ_\"Кондомская\""/LConn3 -- bus121/LConn1
  _CN_312889001_110000_CN_60047767_110000/LConn1 -- T_312889001_110000;6000_ПС_БНС_ТЭЦ_3/LConn1 -- С_246_CN_312889001_110000_CN_313033143_110000/LConn1 -- С_246_CN_312889001_110000_CN_60450100_110000/LConn1
  _CN_312889001_110000_CN_60047767_110000/LConn2 -- T_312889001_110000;6000_ПС_БНС_ТЭЦ_3/LConn2 -- С_246_CN_312889001_110000_CN_313033143_110000/LConn2 -- С_246_CN_312889001_110000_CN_60450100_110000/LConn2
  _CN_312889001_110000_CN_60047767_110000/LConn3 -- T_312889001_110000;6000_ПС_БНС_ТЭЦ_3/LConn3 -- С_246_CN_312889001_110000_CN_313033143_110000/LConn3 -- С_246_CN_312889001_110000_CN_60450100_110000/LConn3 -- bus122/LConn1
  _CN_312889001_110000_CN_60047767_110000/RConn1 -- G_60047767_Красноярская_ТЭЦ_3/RConn1 -- С_243___С_244_CN_60450100_110000_CN_60047767_110000/LConn1 -- _CN_48050742_220000_CN_60047767_110000/LConn1 -- _CN_305389785_220000_CN_60047767_110000/LConn1
  _CN_312889001_110000_CN_60047767_110000/RConn2 -- G_60047767_Красноярская_ТЭЦ_3/RConn2 -- С_243___С_244_CN_60450100_110000_CN_60047767_110000/LConn2 -- _CN_48050742_220000_CN_60047767_110000/LConn2 -- _CN_305389785_220000_CN_60047767_110000/LConn2
  _CN_312889001_110000_CN_60047767_110000/RConn3 -- G_60047767_Красноярская_ТЭЦ_3/RConn3 -- С_243___С_244_CN_60450100_110000_CN_60047767_110000/LConn3 -- _CN_48050742_220000_CN_60047767_110000/LConn3 -- _CN_305389785_220000_CN_60047767_110000/LConn3 -- bus123/LConn1
  "T_313033143_110000;10000_ПС_№147_\"Речпорт\""/LConn1 -- С_246_CN_312889001_110000_CN_313033143_110000/RConn1
  "T_313033143_110000;10000_ПС_№147_\"Речпорт\""/LConn2 -- С_246_CN_312889001_110000_CN_313033143_110000/RConn2
  С_246_CN_312889001_110000_CN_313033143_110000/RConn3 -- "T_313033143_110000;10000_ПС_№147_\"Речпорт\""/LConn3 -- bus124/LConn1
  С_246_CN_312889001_110000_CN_60450100_110000/RConn1 -- "T_60450100_220000;110000_ПС_\"КИСК\""/LConn1 -- _CN_60450100_110000_CN_295819200_110000/LConn1 -- С_243___С_244_CN_60450100_110000_CN_60047767_110000/RConn1
  С_246_CN_312889001_110000_CN_60450100_110000/RConn2 -- "T_60450100_220000;110000_ПС_\"КИСК\""/LConn2 -- _CN_60450100_110000_CN_295819200_110000/LConn2 -- С_243___С_244_CN_60450100_110000_CN_60047767_110000/RConn2
  С_246_CN_312889001_110000_CN_60450100_110000/RConn3 -- "T_60450100_220000;110000_ПС_\"КИСК\""/LConn3 -- _CN_60450100_110000_CN_295819200_110000/LConn3 -- С_243___С_244_CN_60450100_110000_CN_60047767_110000/RConn3 -- bus125/LConn1
  "T_285451553_110000;10000_ПС_№134_\"Солонцы\""/LConn1 -- _CN_203496562_110000_CN_285451553_110000/RConn1
  "T_285451553_110000;10000_ПС_№134_\"Солонцы\""/LConn2 -- _CN_203496562_110000_CN_285451553_110000/RConn2
  _CN_203496562_110000_CN_285451553_110000/RConn3 -- "T_285451553_110000;10000_ПС_№134_\"Солонцы\""/LConn3 -- bus126/LConn1
  "T_202168530_110000;10000_ПС_\"Слобода_весны\""/LConn1 -- _CN_203496562_110000_CN_202168530_110000/RConn1
  "T_202168530_110000;10000_ПС_\"Слобода_весны\""/LConn2 -- _CN_203496562_110000_CN_202168530_110000/RConn2
  _CN_203496562_110000_CN_202168530_110000/RConn3 -- "T_202168530_110000;10000_ПС_\"Слобода_весны\""/LConn3 -- bus127/LConn1
  "T_202168527_110000;10000_ПС_№71_\"Весна\""/LConn1 -- С_213_CN_203496562_110000_CN_202168527_110000/RConn1
  "T_202168527_110000;10000_ПС_№71_\"Весна\""/LConn2 -- С_213_CN_203496562_110000_CN_202168527_110000/RConn2
  С_213_CN_203496562_110000_CN_202168527_110000/RConn3 -- "T_202168527_110000;10000_ПС_№71_\"Весна\""/LConn3 -- bus128/LConn1
  Т_1_Т_4_(ПС_«Восточная»___СХК___ПС_«Восточная»___ПС_«Пиковая»)_CN_77195444_110000_CN_162583841_110000/RConn1 -- T_162583841_220000_Подстанция_«ГПП_220»/RConn1 -- L_162583841/LConn1
  Т_1_Т_4_(ПС_«Восточная»___СХК___ПС_«Восточная»___ПС_«Пиковая»)_CN_77195444_110000_CN_162583841_110000/RConn2 -- T_162583841_220000_Подстанция_«ГПП_220»/RConn2 -- L_162583841/LConn2
  Т_1_Т_4_(ПС_«Восточная»___СХК___ПС_«Восточная»___ПС_«Пиковая»)_CN_77195444_110000_CN_162583841_110000/RConn3 -- T_162583841_220000_Подстанция_«ГПП_220»/RConn3 -- L_162583841/LConn3 -- bus129/LConn1
  T_162577702__ПС_СХК/LConn1 -- Т_1_Т_4_(ПС_«Восточная»___СХК___ПС_«Восточная»___ПС_«Пиковая»)_CN_77195444_110000_CN_162577702_110000/RConn1
  T_162577702__ПС_СХК/LConn2 -- Т_1_Т_4_(ПС_«Восточная»___СХК___ПС_«Восточная»___ПС_«Пиковая»)_CN_77195444_110000_CN_162577702_110000/RConn2
  Т_1_Т_4_(ПС_«Восточная»___СХК___ПС_«Восточная»___ПС_«Пиковая»)_CN_77195444_110000_CN_162577702_110000/RConn3 -- T_162577702__ПС_СХК/LConn3 -- bus130/LConn1
  T_149712234_110000_Подстанция_«Пиковая»/LConn1 -- Т_1_Т_4_(ПС_«Восточная»___СХК___ПС_«Восточная»___ПС_«Пиковая»)_CN_77195444_110000_CN_149712234_110000/RConn1
  T_149712234_110000_Подстанция_«Пиковая»/LConn2 -- Т_1_Т_4_(ПС_«Восточная»___СХК___ПС_«Восточная»___ПС_«Пиковая»)_CN_77195444_110000_CN_149712234_110000/RConn2
  Т_1_Т_4_(ПС_«Восточная»___СХК___ПС_«Восточная»___ПС_«Пиковая»)_CN_77195444_110000_CN_149712234_110000/RConn3 -- T_149712234_110000_Подстанция_«Пиковая»/LConn3 -- bus131/LConn1
  "С_1__С_2_(ГРЭС_2___ПС_\"Восточная\")_CN_77195444_110000_CN_124009952_110000"/RConn1 -- G_124009952_ГРЭС_2/RConn1 -- "С_3_С_4_(ПС_\"Зональная\"___ГРЭС_2)_CN_123874057_110000_CN_124009952_110000"/RConn1
  "С_1__С_2_(ГРЭС_2___ПС_\"Восточная\")_CN_77195444_110000_CN_124009952_110000"/RConn2 -- G_124009952_ГРЭС_2/RConn2 -- "С_3_С_4_(ПС_\"Зональная\"___ГРЭС_2)_CN_123874057_110000_CN_124009952_110000"/RConn2
  "С_1__С_2_(ГРЭС_2___ПС_\"Восточная\")_CN_77195444_110000_CN_124009952_110000"/RConn3 -- G_124009952_ГРЭС_2/RConn3 -- "С_3_С_4_(ПС_\"Зональная\"___ГРЭС_2)_CN_123874057_110000_CN_124009952_110000"/RConn3 -- bus132/LConn1
  _CN_105831607_110000_CN_107196366_110000/LConn1 -- T_105831607__Камала_1/RConn1 -- L_105831607/LConn1
  _CN_105831607_110000_CN_107196366_110000/LConn2 -- T_105831607__Камала_1/RConn2 -- L_105831607/LConn2
  _CN_105831607_110000_CN_107196366_110000/LConn3 -- T_105831607__Камала_1/RConn3 -- L_105831607/LConn3 -- bus133/LConn1
  "T_107196366__ГПП_1_\"Первая_Городская\""/LConn1 -- _CN_105831607_110000_CN_107196366_110000/RConn1
  "T_107196366__ГПП_1_\"Первая_Городская\""/LConn2 -- _CN_105831607_110000_CN_107196366_110000/RConn2
  _CN_105831607_110000_CN_107196366_110000/RConn3 -- "T_107196366__ГПП_1_\"Первая_Городская\""/LConn3 -- bus134/LConn1
  T_274464446__/LConn1 -- _CN_274464446_110000_CN_289973452_110000/LConn1
  T_274464446__/LConn2 -- _CN_274464446_110000_CN_289973452_110000/LConn2
  _CN_274464446_110000_CN_289973452_110000/LConn3 -- T_274464446__/LConn3 -- bus135/LConn1
  T_289973452__/LConn1 -- _CN_274464446_110000_CN_289973452_110000/RConn1
  T_289973452__/LConn2 -- _CN_274464446_110000_CN_289973452_110000/RConn2
  _CN_274464446_110000_CN_289973452_110000/RConn3 -- T_289973452__/LConn3 -- bus136/LConn1
  T_190450368_110000_Подстанция_«Григорьевская»/LConn1 -- _CN_190450368_110000_CN_89555905_110000/LConn1
  T_190450368_110000_Подстанция_«Григорьевская»/LConn2 -- _CN_190450368_110000_CN_89555905_110000/LConn2
  _CN_190450368_110000_CN_89555905_110000/LConn3 -- T_190450368_110000_Подстанция_«Григорьевская»/LConn3 -- bus137/LConn1
  T_89555905_110000_Подстанция_«Стрежевская»/LConn1 -- _CN_190450368_110000_CN_89555905_110000/RConn1
  T_89555905_110000_Подстанция_«Стрежевская»/LConn2 -- _CN_190450368_110000_CN_89555905_110000/RConn2
  _CN_190450368_110000_CN_89555905_110000/RConn3 -- T_89555905_110000_Подстанция_«Стрежевская»/LConn3 -- bus138/LConn1
  T_316964474__/LConn1 -- С_111_(С_112?)_(ПС_«Чажемто_220»___ПС_«Первомайская»_консерв)_CN_169356997_110000_CN_316964474_110000/RConn1
  T_316964474__/LConn2 -- С_111_(С_112?)_(ПС_«Чажемто_220»___ПС_«Первомайская»_консерв)_CN_169356997_110000_CN_316964474_110000/RConn2
  С_111_(С_112?)_(ПС_«Чажемто_220»___ПС_«Первомайская»_консерв)_CN_169356997_110000_CN_316964474_110000/RConn3 -- T_316964474__/LConn3 -- bus139/LConn1
  T_169700760_110000_Подстанция_«Чажемто_110»/LConn1 -- С_29_С_39_(ПС_«Чажемто_220»___ПС_«Чажемто_110»)_CN_169356997_110000_CN_169700760_110000/RConn1
  T_169700760_110000_Подстанция_«Чажемто_110»/LConn2 -- С_29_С_39_(ПС_«Чажемто_220»___ПС_«Чажемто_110»)_CN_169356997_110000_CN_169700760_110000/RConn2
  С_29_С_39_(ПС_«Чажемто_220»___ПС_«Чажемто_110»)_CN_169356997_110000_CN_169700760_110000/RConn3 -- T_169700760_110000_Подстанция_«Чажемто_110»/LConn3 -- bus140/LConn1
  T_134436050_110000_Подстанция_«Малореченская»/LConn1 -- С_95М_С_96М_(ПС_«Александровская»___ПС_«Малореченская»)_CN_134436050_110000_CN_130469640_110000/LConn1
  T_134436050_110000_Подстанция_«Малореченская»/LConn2 -- С_95М_С_96М_(ПС_«Александровская»___ПС_«Малореченская»)_CN_134436050_110000_CN_130469640_110000/LConn2
  С_95М_С_96М_(ПС_«Александровская»___ПС_«Малореченская»)_CN_134436050_110000_CN_130469640_110000/LConn3 -- T_134436050_110000_Подстанция_«Малореченская»/LConn3 -- bus141/LConn1
  T_130469640_110000_ПС_«Александровская»_110_10/LConn1 -- С_95М_С_96М_(ПС_«Александровская»___ПС_«Малореченская»)_CN_134436050_110000_CN_130469640_110000/RConn1
  T_130469640_110000_ПС_«Александровская»_110_10/LConn2 -- С_95М_С_96М_(ПС_«Александровская»___ПС_«Малореченская»)_CN_134436050_110000_CN_130469640_110000/RConn2
  С_95М_С_96М_(ПС_«Александровская»___ПС_«Малореченская»)_CN_134436050_110000_CN_130469640_110000/RConn3 -- T_130469640_110000_ПС_«Александровская»_110_10/LConn3 -- bus142/LConn1
  С_61_С_62_(ПС_«Асино_110»___ПС_«Зырянка»)_CN_169734094_110000_CN_245392698_110000/RConn1 -- T_245392698_110000_Подстанция_«Чердаты»/LConn1 -- С_63_С_64_(ПС_«Чердаты»___ПС_«Тегульдет»)_CN_219125213_110000_CN_245392698_110000/LConn1
  С_61_С_62_(ПС_«Асино_110»___ПС_«Зырянка»)_CN_169734094_110000_CN_245392698_110000/RConn2 -- T_245392698_110000_Подстанция_«Чердаты»/LConn2 -- С_63_С_64_(ПС_«Чердаты»___ПС_«Тегульдет»)_CN_219125213_110000_CN_245392698_110000/LConn2
  С_61_С_62_(ПС_«Асино_110»___ПС_«Зырянка»)_CN_169734094_110000_CN_245392698_110000/RConn3 -- T_245392698_110000_Подстанция_«Чердаты»/LConn3 -- С_63_С_64_(ПС_«Чердаты»___ПС_«Тегульдет»)_CN_219125213_110000_CN_245392698_110000/LConn3 -- bus143/LConn1
  T_243298567_110000_Подстанция_«Зырянка»/LConn1 -- С_61_С_62_(ПС_«Асино_110»___ПС_«Зырянка»)_CN_169734094_110000_CN_243298567_110000/RConn1
  T_243298567_110000_Подстанция_«Зырянка»/LConn2 -- С_61_С_62_(ПС_«Асино_110»___ПС_«Зырянка»)_CN_169734094_110000_CN_243298567_110000/RConn2
  С_61_С_62_(ПС_«Асино_110»___ПС_«Зырянка»)_CN_169734094_110000_CN_243298567_110000/RConn3 -- T_243298567_110000_Подстанция_«Зырянка»/LConn3 -- bus144/LConn1
  АС_70_(ПС_«Веселовская»___ПС_«Зубковская»)_CN_100146904_110000_CN_201600388_110000/LConn1 -- T_100146904_110000_Подстанция_«Зубковская»/LConn1 -- АС_70_(ПС_«Веселовская»___ПС_«Зубковская»)_CN_100146904_110000_CN_100118265_110000/LConn1 -- АС_70_(ПС_«Веселовская»___ПС_«Зубковская»)_CN_100146904_110000_CN_201600393_110000/LConn1
  АС_70_(ПС_«Веселовская»___ПС_«Зубковская»)_CN_100146904_110000_CN_201600388_110000/LConn2 -- T_100146904_110000_Подстанция_«Зубковская»/LConn2 -- АС_70_(ПС_«Веселовская»___ПС_«Зубковская»)_CN_100146904_110000_CN_100118265_110000/LConn2 -- АС_70_(ПС_«Веселовская»___ПС_«Зубковская»)_CN_100146904_110000_CN_201600393_110000/LConn2
  АС_70_(ПС_«Веселовская»___ПС_«Зубковская»)_CN_100146904_110000_CN_201600388_110000/LConn3 -- T_100146904_110000_Подстанция_«Зубковская»/LConn3 -- АС_70_(ПС_«Веселовская»___ПС_«Зубковская»)_CN_100146904_110000_CN_100118265_110000/LConn3 -- АС_70_(ПС_«Веселовская»___ПС_«Зубковская»)_CN_100146904_110000_CN_201600393_110000/LConn3 -- bus145/LConn1
  T_201600388_110000_Подстанция_«Веселовская»/LConn1 -- АС_70_(ПС_«Веселовская»___ПС_«Зубковская»)_CN_100146904_110000_CN_201600388_110000/RConn1
  T_201600388_110000_Подстанция_«Веселовская»/LConn2 -- АС_70_(ПС_«Веселовская»___ПС_«Зубковская»)_CN_100146904_110000_CN_201600388_110000/RConn2
  АС_70_(ПС_«Веселовская»___ПС_«Зубковская»)_CN_100146904_110000_CN_201600388_110000/RConn3 -- T_201600388_110000_Подстанция_«Веселовская»/LConn3 -- bus146/LConn1
  T_100118265_110000_Подстанция_«Нива»/LConn1 -- АС_70_(ПС_«Веселовская»___ПС_«Зубковская»)_CN_100146904_110000_CN_100118265_110000/RConn1
  T_100118265_110000_Подстанция_«Нива»/LConn2 -- АС_70_(ПС_«Веселовская»___ПС_«Зубковская»)_CN_100146904_110000_CN_100118265_110000/RConn2
  АС_70_(ПС_«Веселовская»___ПС_«Зубковская»)_CN_100146904_110000_CN_100118265_110000/RConn3 -- T_100118265_110000_Подстанция_«Нива»/LConn3 -- bus147/LConn1
  АС_70_(ПС_«Веселовская»___ПС_«Зубковская»)_CN_100146904_110000_CN_201600393_110000/RConn1 -- T_201600393_110000_Подстанция_«Лянино»/LConn1 -- ПС_«Лянино»___ПС_«Верх_Угрюм»_CN_201600393_110000_CN_201600394_110000/LConn1
  АС_70_(ПС_«Веселовская»___ПС_«Зубковская»)_CN_100146904_110000_CN_201600393_110000/RConn2 -- T_201600393_110000_Подстанция_«Лянино»/LConn2 -- ПС_«Лянино»___ПС_«Верх_Угрюм»_CN_201600393_110000_CN_201600394_110000/LConn2
  АС_70_(ПС_«Веселовская»___ПС_«Зубковская»)_CN_100146904_110000_CN_201600393_110000/RConn3 -- T_201600393_110000_Подстанция_«Лянино»/LConn3 -- ПС_«Лянино»___ПС_«Верх_Угрюм»_CN_201600393_110000_CN_201600394_110000/LConn3 -- bus148/LConn1
  T_374528071__/LConn1 -- С_58_С_59_(ПС_«Белый_Яр»___ПС_«Клюквинка»)_CN_202927834_110000_CN_374528071_110000/RConn1
  T_374528071__/LConn2 -- С_58_С_59_(ПС_«Белый_Яр»___ПС_«Клюквинка»)_CN_202927834_110000_CN_374528071_110000/RConn2
  С_58_С_59_(ПС_«Белый_Яр»___ПС_«Клюквинка»)_CN_202927834_110000_CN_374528071_110000/RConn3 -- T_374528071__/LConn3 -- bus149/LConn1
  С_22_С_32_(ПС_«Мельниково_220»___ПС_«Володино_220»)_CN_189871845_110000_CN_169671124_110000/RConn1 -- T_169671124_220000_Подстанция_«Мельниково_220»/RConn1 -- L_169671124/LConn1
  С_22_С_32_(ПС_«Мельниково_220»___ПС_«Володино_220»)_CN_189871845_110000_CN_169671124_110000/RConn2 -- T_169671124_220000_Подстанция_«Мельниково_220»/RConn2 -- L_169671124/LConn2
  С_22_С_32_(ПС_«Мельниково_220»___ПС_«Володино_220»)_CN_189871845_110000_CN_169671124_110000/RConn3 -- T_169671124_220000_Подстанция_«Мельниково_220»/RConn3 -- L_169671124/LConn3 -- bus150/LConn1
  _CN_131753195_110000_CN_176748969_110000/LConn1 -- T_131753195_500000;220000;fixme_Подстанция_«Абаканская»/RConn4 -- _CN_131753195_110000_CN_223867037_110000/LConn1 -- L_131753195/LConn1
  _CN_131753195_110000_CN_176748969_110000/LConn2 -- T_131753195_500000;220000;fixme_Подстанция_«Абаканская»/RConn5 -- _CN_131753195_110000_CN_223867037_110000/LConn2 -- L_131753195/LConn2
  _CN_131753195_110000_CN_176748969_110000/LConn3 -- T_131753195_500000;220000;fixme_Подстанция_«Абаканская»/RConn6 -- _CN_131753195_110000_CN_223867037_110000/LConn3 -- L_131753195/LConn3 -- bus151/LConn1
  T_176748969__/LConn1 -- _CN_131753195_110000_CN_176748969_110000/RConn1
  T_176748969__/LConn2 -- _CN_131753195_110000_CN_176748969_110000/RConn2
  _CN_131753195_110000_CN_176748969_110000/RConn3 -- T_176748969__/LConn3 -- bus152/LConn1
  T_223867037__/LConn1 -- _CN_131753195_110000_CN_223867037_110000/RConn1
  T_223867037__/LConn2 -- _CN_131753195_110000_CN_223867037_110000/RConn2
  _CN_131753195_110000_CN_223867037_110000/RConn3 -- T_223867037__/LConn3 -- bus153/LConn1
  T_191079379_110000_Подстанция_110_35_10_кВ_«ОЭЗ»/LConn1 -- "?_(ПС_«Зональная»___ПС_«ОЭЗ»)_CN_191079379_110000_CN_123874057_110000"/RConn1
  T_191079379_110000_Подстанция_110_35_10_кВ_«ОЭЗ»/LConn2 -- "?_(ПС_«Зональная»___ПС_«ОЭЗ»)_CN_191079379_110000_CN_123874057_110000"/RConn2
  "?_(ПС_«Зональная»___ПС_«ОЭЗ»)_CN_191079379_110000_CN_123874057_110000"/RConn3 -- T_191079379_110000_Подстанция_110_35_10_кВ_«ОЭЗ»/LConn3 -- bus154/LConn1
  T_192046328__/LConn1 -- _CN_192046328_110000_CN_76228618_110000/LConn1
  T_192046328__/LConn2 -- _CN_192046328_110000_CN_76228618_110000/LConn2
  _CN_192046328_110000_CN_76228618_110000/LConn3 -- T_192046328__/LConn3 -- bus155/LConn1
  _CN_192046328_110000_CN_76228618_110000/RConn1 -- G_76228618_ТЭЦ_3/RConn1 -- Т_210_(ПС_«Томская»___ТЭЦ_3)_CN_166018985_220000_CN_76228618_110000/LConn1 -- Т_211_Т_212_(ТЭЦ_3___ПС_«ГПП_220»)_CN_162583841_220000_CN_76228618_110000/LConn1
  _CN_192046328_110000_CN_76228618_110000/RConn2 -- G_76228618_ТЭЦ_3/RConn2 -- Т_210_(ПС_«Томская»___ТЭЦ_3)_CN_166018985_220000_CN_76228618_110000/LConn2 -- Т_211_Т_212_(ТЭЦ_3___ПС_«ГПП_220»)_CN_162583841_220000_CN_76228618_110000/LConn2
  _CN_192046328_110000_CN_76228618_110000/RConn3 -- G_76228618_ТЭЦ_3/RConn3 -- Т_210_(ПС_«Томская»___ТЭЦ_3)_CN_166018985_220000_CN_76228618_110000/LConn3 -- bus156/LConn1 -- Т_211_Т_212_(ТЭЦ_3___ПС_«ГПП_220»)_CN_162583841_220000_CN_76228618_110000/LConn3
  T_169996149_110000_Подстанция_«Кандинка_110»/LConn1 -- С_13_С_14_(ПС_«Левобережная»___ПС_«Кандинка_110»)_CN_150289682_110000_CN_169996149_110000/RConn1
  T_169996149_110000_Подстанция_«Кандинка_110»/LConn2 -- С_13_С_14_(ПС_«Левобережная»___ПС_«Кандинка_110»)_CN_150289682_110000_CN_169996149_110000/RConn2
  С_13_С_14_(ПС_«Левобережная»___ПС_«Кандинка_110»)_CN_150289682_110000_CN_169996149_110000/RConn3 -- T_169996149_110000_Подстанция_«Кандинка_110»/LConn3 -- bus157/LConn1
  С_13___С_14_CN_267632930_110000_CN_106887628_110000/RConn1 -- "T_267632930_110000_ПС_№7_\"Медпрепараты\""/LConn1 -- С_13___С_14_CN_267632930_110000_CN_275667154_110000/LConn1 -- С_13___С_14_CN_267632930_110000_CN_279030763_110000/LConn1 -- С_13___С_14_CN_267632930_110000_CN_202649908_110000/RConn1
  С_13___С_14_CN_267632930_110000_CN_106887628_110000/RConn2 -- "T_267632930_110000_ПС_№7_\"Медпрепараты\""/LConn2 -- С_13___С_14_CN_267632930_110000_CN_275667154_110000/LConn2 -- С_13___С_14_CN_267632930_110000_CN_279030763_110000/LConn2 -- С_13___С_14_CN_267632930_110000_CN_202649908_110000/RConn2
  С_13___С_14_CN_267632930_110000_CN_106887628_110000/RConn3 -- "T_267632930_110000_ПС_№7_\"Медпрепараты\""/LConn3 -- С_13___С_14_CN_267632930_110000_CN_275667154_110000/LConn3 -- С_13___С_14_CN_267632930_110000_CN_279030763_110000/LConn3 -- С_13___С_14_CN_267632930_110000_CN_202649908_110000/RConn3 -- bus158/LConn1
  "T_275667154_110000;35000;6000_ПС_№92_\"Юго_Западная\""/LConn1 -- С_13___С_14_CN_267632930_110000_CN_275667154_110000/RConn1
  "T_275667154_110000;35000;6000_ПС_№92_\"Юго_Западная\""/LConn2 -- С_13___С_14_CN_267632930_110000_CN_275667154_110000/RConn2
  С_13___С_14_CN_267632930_110000_CN_275667154_110000/RConn3 -- "T_275667154_110000;35000;6000_ПС_№92_\"Юго_Западная\""/LConn3 -- bus159/LConn1
  "T_279030763_110000;6000_ПС_№65_\"Бобровый_лог\""/LConn1 -- С_13___С_14_CN_267632930_110000_CN_279030763_110000/RConn1
  "T_279030763_110000;6000_ПС_№65_\"Бобровый_лог\""/LConn2 -- С_13___С_14_CN_267632930_110000_CN_279030763_110000/RConn2
  С_13___С_14_CN_267632930_110000_CN_279030763_110000/RConn3 -- "T_279030763_110000;6000_ПС_№65_\"Бобровый_лог\""/LConn3 -- bus160/LConn1
  T_130482986_110000_Подстанция_«Раздольное»/LConn1 -- С_93_(С_94?)_(ПС_«Чапаевка»___ПС_«Раздольное»)_CN_130482986_110000_CN_191588676_110000/RConn1
  T_130482986_110000_Подстанция_«Раздольное»/LConn2 -- С_93_(С_94?)_(ПС_«Чапаевка»___ПС_«Раздольное»)_CN_130482986_110000_CN_191588676_110000/RConn2
  С_93_(С_94?)_(ПС_«Чапаевка»___ПС_«Раздольное»)_CN_130482986_110000_CN_191588676_110000/RConn3 -- T_130482986_110000_Подстанция_«Раздольное»/LConn3 -- bus161/LConn1
  T_219125213_110000_Подстанция_«Тегульдет»/LConn1 -- С_63_С_64_(ПС_«Чердаты»___ПС_«Тегульдет»)_CN_219125213_110000_CN_245392698_110000/RConn1
  T_219125213_110000_Подстанция_«Тегульдет»/LConn2 -- С_63_С_64_(ПС_«Чердаты»___ПС_«Тегульдет»)_CN_219125213_110000_CN_245392698_110000/RConn2
  С_63_С_64_(ПС_«Чердаты»___ПС_«Тегульдет»)_CN_219125213_110000_CN_245392698_110000/RConn3 -- T_219125213_110000_Подстанция_«Тегульдет»/LConn3 -- bus162/LConn1
  "T_295819200_110000;10000_ПС_№49_\"Юбилейная\""/LConn1 -- _CN_60450100_110000_CN_295819200_110000/RConn1
  "T_295819200_110000;10000_ПС_№49_\"Юбилейная\""/LConn2 -- _CN_60450100_110000_CN_295819200_110000/RConn2
  _CN_60450100_110000_CN_295819200_110000/RConn3 -- "T_295819200_110000;10000_ПС_№49_\"Юбилейная\""/LConn3 -- bus163/LConn1
  T_194903352_110000_Подстанция_«Калиновая»/LConn1 -- С_105_106_(ПС_«Лугинецкая»___ПС_«Калиновая»)_CN_194903352_110000_CN_197782305_110000/RConn1
  T_194903352_110000_Подстанция_«Калиновая»/LConn2 -- С_105_106_(ПС_«Лугинецкая»___ПС_«Калиновая»)_CN_194903352_110000_CN_197782305_110000/RConn2
  С_105_106_(ПС_«Лугинецкая»___ПС_«Калиновая»)_CN_194903352_110000_CN_197782305_110000/RConn3 -- T_194903352_110000_Подстанция_«Калиновая»/LConn3 -- bus164/LConn1
  С_109_(С_110?)_(ПС_«Лугинецкая»___ПС_«Игольская»)_CN_197782305_110000_CN_195060971_110000/RConn1 -- T_195060971_110000_Подстанция_«Игольская»/LConn1 -- С_140_С_141_(ПС_«Двуреченская»___ПС_«Игольская»)_CN_194874204_110000_CN_195060971_110000/LConn1
  С_109_(С_110?)_(ПС_«Лугинецкая»___ПС_«Игольская»)_CN_197782305_110000_CN_195060971_110000/RConn2 -- T_195060971_110000_Подстанция_«Игольская»/LConn2 -- С_140_С_141_(ПС_«Двуреченская»___ПС_«Игольская»)_CN_194874204_110000_CN_195060971_110000/LConn2
  С_109_(С_110?)_(ПС_«Лугинецкая»___ПС_«Игольская»)_CN_197782305_110000_CN_195060971_110000/RConn3 -- T_195060971_110000_Подстанция_«Игольская»/LConn3 -- С_140_С_141_(ПС_«Двуреченская»___ПС_«Игольская»)_CN_194874204_110000_CN_195060971_110000/LConn3 -- bus165/LConn1
  T_332123970__/LConn1 -- _CN_332123970_110000_CN_332122569_110000/LConn1
  T_332123970__/LConn2 -- _CN_332123970_110000_CN_332122569_110000/LConn2
  _CN_332123970_110000_CN_332122569_110000/LConn3 -- T_332123970__/LConn3 -- bus166/LConn1
  T_332122569__/LConn1 -- _CN_332123970_110000_CN_332122569_110000/RConn1
  T_332122569__/LConn2 -- _CN_332123970_110000_CN_332122569_110000/RConn2
  _CN_332123970_110000_CN_332122569_110000/RConn3 -- T_332122569__/LConn3 -- bus167/LConn1
  T_194874204_110000_Подстанция_«Крапивинская»/LConn1 -- С_140_С_141_(ПС_«Двуреченская»___ПС_«Игольская»)_CN_194874204_110000_CN_195060971_110000/RConn1
  T_194874204_110000_Подстанция_«Крапивинская»/LConn2 -- С_140_С_141_(ПС_«Двуреченская»___ПС_«Игольская»)_CN_194874204_110000_CN_195060971_110000/RConn2
  С_140_С_141_(ПС_«Двуреченская»___ПС_«Игольская»)_CN_194874204_110000_CN_195060971_110000/RConn3 -- T_194874204_110000_Подстанция_«Крапивинская»/LConn3 -- bus168/LConn1
  T_100718452__Ефремовская/LConn1 -- _CN_100718452_110000_CN_94337786_110000/LConn1
  T_100718452__Ефремовская/LConn2 -- _CN_100718452_110000_CN_94337786_110000/LConn2
  _CN_100718452_110000_CN_94337786_110000/LConn3 -- T_100718452__Ефремовская/LConn3 -- bus169/LConn1
  T_94337786__Оловозаводская/LConn1 -- _CN_100718452_110000_CN_94337786_110000/RConn1
  T_94337786__Оловозаводская/LConn2 -- _CN_100718452_110000_CN_94337786_110000/RConn2
  _CN_100718452_110000_CN_94337786_110000/RConn3 -- T_94337786__Оловозаводская/LConn3 -- bus170/LConn1
  T_201600394_110000_Подстанция_«Верх_Угрюм»/LConn1 -- ПС_«Лянино»___ПС_«Верх_Угрюм»_CN_201600393_110000_CN_201600394_110000/RConn1
  T_201600394_110000_Подстанция_«Верх_Угрюм»/LConn2 -- ПС_«Лянино»___ПС_«Верх_Угрюм»_CN_201600393_110000_CN_201600394_110000/RConn2
  ПС_«Лянино»___ПС_«Верх_Угрюм»_CN_201600393_110000_CN_201600394_110000/RConn3 -- T_201600394_110000_Подстанция_«Верх_Угрюм»/LConn3 -- bus171/LConn1
  _CN_203056539_110000_CN_298817867_110000/LConn1 -- T_203056539__Тяговая_ПС_Суховская/LConn1 -- _CN_203056539_110000_CN_297714701_110000/LConn1
  _CN_203056539_110000_CN_298817867_110000/LConn2 -- T_203056539__Тяговая_ПС_Суховская/LConn2 -- _CN_203056539_110000_CN_297714701_110000/LConn2
  _CN_203056539_110000_CN_298817867_110000/LConn3 -- T_203056539__Тяговая_ПС_Суховская/LConn3 -- _CN_203056539_110000_CN_297714701_110000/LConn3 -- bus172/LConn1
  T_298817867__/LConn1 -- _CN_203056539_110000_CN_298817867_110000/RConn1
  T_298817867__/LConn2 -- _CN_203056539_110000_CN_298817867_110000/RConn2
  _CN_203056539_110000_CN_298817867_110000/RConn3 -- T_298817867__/LConn3 -- bus173/LConn1
  _CN_203056539_110000_CN_297714701_110000/RConn1 -- G_297714701_/RConn1 -- _CN_184798669_110000_CN_297714701_110000/RConn1
  _CN_203056539_110000_CN_297714701_110000/RConn2 -- G_297714701_/RConn2 -- _CN_184798669_110000_CN_297714701_110000/RConn2
  _CN_203056539_110000_CN_297714701_110000/RConn3 -- G_297714701_/RConn3 -- _CN_184798669_110000_CN_297714701_110000/RConn3 -- bus174/LConn1
  T_367574444__/LConn1 -- _CN_367574444_110000_CN_283373486_110000/LConn1
  T_367574444__/LConn2 -- _CN_367574444_110000_CN_283373486_110000/LConn2
  _CN_367574444_110000_CN_283373486_110000/LConn3 -- T_367574444__/LConn3 -- bus175/LConn1
  T_283373486__/LConn1 -- _CN_367574444_110000_CN_283373486_110000/RConn1
  T_283373486__/LConn2 -- _CN_367574444_110000_CN_283373486_110000/RConn2
  _CN_367574444_110000_CN_283373486_110000/RConn3 -- T_283373486__/LConn3 -- bus176/LConn1
  Д_12_CN_59261969_220000_CN_110542603_220000/LConn1 -- "T_59261969_220000;110000;10000_ПС_\"Дивногорск\""/LConn1 -- Д_18_CN_59261969_220000_CN_198719682_220000/LConn1
  Д_12_CN_59261969_220000_CN_110542603_220000/LConn2 -- "T_59261969_220000;110000;10000_ПС_\"Дивногорск\""/LConn2 -- Д_18_CN_59261969_220000_CN_198719682_220000/LConn2
  Д_12_CN_59261969_220000_CN_110542603_220000/LConn3 -- "T_59261969_220000;110000;10000_ПС_\"Дивногорск\""/LConn3 -- Д_18_CN_59261969_220000_CN_198719682_220000/LConn3 -- bus177/LConn1
  Д_12_CN_59261969_220000_CN_110542603_220000/RConn1 -- "T_110542603_220000_ПС_№152_\"Новокрасноярская\""/LConn1 -- _CN_305389785_220000_CN_110542603_220000/LConn1 -- _CN_60040448_220000_CN_110542603_220000/LConn1
  Д_12_CN_59261969_220000_CN_110542603_220000/RConn2 -- "T_110542603_220000_ПС_№152_\"Новокрасноярская\""/LConn2 -- _CN_305389785_220000_CN_110542603_220000/LConn2 -- _CN_60040448_220000_CN_110542603_220000/LConn2
  Д_12_CN_59261969_220000_CN_110542603_220000/RConn3 -- "T_110542603_220000_ПС_№152_\"Новокрасноярская\""/LConn3 -- _CN_305389785_220000_CN_110542603_220000/LConn3 -- _CN_60040448_220000_CN_110542603_220000/LConn3 -- bus178/LConn1
  "T_198719682_220000;110000;10000;6000_ПС_\"Правобережная\""/LConn1 -- Д_18_CN_59261969_220000_CN_198719682_220000/RConn1
  "T_198719682_220000;110000;10000;6000_ПС_\"Правобережная\""/LConn2 -- Д_18_CN_59261969_220000_CN_198719682_220000/RConn2
  Д_18_CN_59261969_220000_CN_198719682_220000/RConn3 -- "T_198719682_220000;110000;10000;6000_ПС_\"Правобережная\""/LConn3 -- bus179/LConn1
  T_116607512__/LConn1 -- _CN_116607512_220000_CN_113555542_220000/LConn1
  T_116607512__/LConn2 -- _CN_116607512_220000_CN_113555542_220000/LConn2
  _CN_116607512_220000_CN_113555542_220000/LConn3 -- T_116607512__/LConn3 -- bus180/LConn1
  _CN_116607512_220000_CN_113555542_220000/RConn1 -- G_113555542_ТЭЦ_7/RConn1 -- _CN_110601357_220000_CN_113555542_220000/LConn1
  _CN_116607512_220000_CN_113555542_220000/RConn2 -- G_113555542_ТЭЦ_7/RConn2 -- _CN_110601357_220000_CN_113555542_220000/LConn2
  _CN_116607512_220000_CN_113555542_220000/RConn3 -- G_113555542_ТЭЦ_7/RConn3 -- _CN_110601357_220000_CN_113555542_220000/LConn3 -- bus181/LConn1
  _CN_51129883_220000_CN_51809085_220000/LConn1 -- T_51129883__Восточная/LConn1 -- _CN_51129883_220000_CN_51857448_110000/RConn1
  _CN_51129883_220000_CN_51809085_220000/LConn2 -- T_51129883__Восточная/LConn2 -- _CN_51129883_220000_CN_51857448_110000/RConn2
  _CN_51129883_220000_CN_51809085_220000/LConn3 -- T_51129883__Восточная/LConn3 -- _CN_51129883_220000_CN_51857448_110000/RConn3 -- bus182/LConn1
  G_51809085_Новосибирская_ГЭС/RConn1 -- _CN_51129883_220000_CN_51809085_220000/RConn1
  G_51809085_Новосибирская_ГЭС/RConn2 -- _CN_51129883_220000_CN_51809085_220000/RConn2
  _CN_51129883_220000_CN_51809085_220000/RConn3 -- G_51809085_Новосибирская_ГЭС/RConn3 -- bus183/LConn1
  T_394149419_220000_Подстанция_«Орловка»/LConn1 -- Отпайка_на_ПС_«Орловка»_от_ТВ_221_ТВ_231_CN_394149419_220000_CN_166018985_220000/LConn1
  T_394149419_220000_Подстанция_«Орловка»/LConn2 -- Отпайка_на_ПС_«Орловка»_от_ТВ_221_ТВ_231_CN_394149419_220000_CN_166018985_220000/LConn2
  Отпайка_на_ПС_«Орловка»_от_ТВ_221_ТВ_231_CN_394149419_220000_CN_166018985_220000/LConn3 -- T_394149419_220000_Подстанция_«Орловка»/LConn3 -- bus184/LConn1
  Отпайка_на_ПС_«Орловка»_от_ТВ_221_ТВ_231_CN_394149419_220000_CN_166018985_220000/RConn1 -- T_166018985_500000_Подстанция_«Томская»/LConn1 -- Т_203_Т_204_(ПС_«Томская»___ПС_«Восточная»)_CN_77195444_220000_CN_166018985_220000/LConn1 -- Т_213_(ПС_«Томская»___ПС_«ГПП_220»)_CN_162583841_220000_CN_166018985_220000/LConn1 -- Т_210_(ПС_«Томская»___ТЭЦ_3)_CN_166018985_220000_CN_76228618_110000/RConn1
  Отпайка_на_ПС_«Орловка»_от_ТВ_221_ТВ_231_CN_394149419_220000_CN_166018985_220000/RConn2 -- T_166018985_500000_Подстанция_«Томская»/LConn2 -- Т_203_Т_204_(ПС_«Томская»___ПС_«Восточная»)_CN_77195444_220000_CN_166018985_220000/LConn2 -- Т_213_(ПС_«Томская»___ПС_«ГПП_220»)_CN_162583841_220000_CN_166018985_220000/LConn2 -- Т_210_(ПС_«Томская»___ТЭЦ_3)_CN_166018985_220000_CN_76228618_110000/RConn2
  Отпайка_на_ПС_«Орловка»_от_ТВ_221_ТВ_231_CN_394149419_220000_CN_166018985_220000/RConn3 -- T_166018985_500000_Подстанция_«Томская»/LConn3 -- Т_203_Т_204_(ПС_«Томская»___ПС_«Восточная»)_CN_77195444_220000_CN_166018985_220000/LConn3 -- Т_213_(ПС_«Томская»___ПС_«ГПП_220»)_CN_162583841_220000_CN_166018985_220000/LConn3 -- Т_210_(ПС_«Томская»___ТЭЦ_3)_CN_166018985_220000_CN_76228618_110000/RConn3 -- bus185/LConn1
  _CN_48050741_220000_CN_48050742_220000/LConn1 -- "T_48050741_500000;220000;35000;10000_ПС_\"Красноярская\""/RConn1 -- L_48050741/LConn1
  _CN_48050741_220000_CN_48050742_220000/LConn2 -- "T_48050741_500000;220000;35000;10000_ПС_\"Красноярская\""/RConn2 -- L_48050741/LConn2
  _CN_48050741_220000_CN_48050742_220000/LConn3 -- "T_48050741_500000;220000;35000;10000_ПС_\"Красноярская\""/RConn3 -- L_48050741/LConn3 -- bus186/LConn1
  _CN_48050741_220000_CN_48050742_220000/RConn1 -- T_48050742_220000_ПС_ЦРП_220_кВ/LConn1 -- _CN_48050742_220000_CN_60047767_110000/RConn1 -- Д_5_CN_48050742_220000_CN_95996044_220000/LConn1 -- _CN_48050742_220000_CN_305389785_220000/LConn1 -- _CN_48050742_220000_CN_60040415_220000/LConn1 -- _CN_48050742_220000_CN_220574879_220000/LConn1 -- _CN_48050742_220000_CN_60040500_220000/LConn1
  _CN_48050741_220000_CN_48050742_220000/RConn2 -- T_48050742_220000_ПС_ЦРП_220_кВ/LConn2 -- _CN_48050742_220000_CN_60047767_110000/RConn2 -- Д_5_CN_48050742_220000_CN_95996044_220000/LConn2 -- _CN_48050742_220000_CN_305389785_220000/LConn2 -- _CN_48050742_220000_CN_60040415_220000/LConn2 -- _CN_48050742_220000_CN_220574879_220000/LConn2 -- _CN_48050742_220000_CN_60040500_220000/LConn2
  _CN_48050741_220000_CN_48050742_220000/RConn3 -- T_48050742_220000_ПС_ЦРП_220_кВ/LConn3 -- _CN_48050742_220000_CN_60047767_110000/RConn3 -- bus187/LConn1 -- Д_5_CN_48050742_220000_CN_95996044_220000/LConn3 -- _CN_48050742_220000_CN_305389785_220000/LConn3 -- _CN_48050742_220000_CN_60040415_220000/LConn3 -- _CN_48050742_220000_CN_220574879_220000/LConn3 -- _CN_48050742_220000_CN_60040500_220000/LConn3
  _CN_48050742_220000_CN_220574879_220000/RConn1 -- T_220574879_220000_ОРУ___ГПП_3/LConn1 -- _CN_60040328_220000_CN_220574879_220000/LConn1 -- _CN_220574879_220000_CN_60040606_220000/LConn1
  _CN_48050742_220000_CN_220574879_220000/RConn2 -- T_220574879_220000_ОРУ___ГПП_3/LConn2 -- _CN_60040328_220000_CN_220574879_220000/LConn2 -- _CN_220574879_220000_CN_60040606_220000/LConn2
  _CN_48050742_220000_CN_220574879_220000/RConn3 -- T_220574879_220000_ОРУ___ГПП_3/LConn3 -- _CN_60040328_220000_CN_220574879_220000/LConn3 -- _CN_220574879_220000_CN_60040606_220000/LConn3 -- bus188/LConn1
  _CN_48050742_220000_CN_60040500_220000/RConn1 -- T_60040500_220000_ОРУ___ГПП_5/LConn1 -- _CN_60040500_220000_CN_60040659_220000/LConn1
  _CN_48050742_220000_CN_60040500_220000/RConn2 -- T_60040500_220000_ОРУ___ГПП_5/LConn2 -- _CN_60040500_220000_CN_60040659_220000/LConn2
  _CN_48050742_220000_CN_60040500_220000/RConn3 -- T_60040500_220000_ОРУ___ГПП_5/LConn3 -- _CN_60040500_220000_CN_60040659_220000/LConn3 -- bus189/LConn1
  _CN_48050742_220000_CN_60040415_220000/RConn1 -- T_60040415_220000_ОРУ___ГПП_1/LConn1 -- _CN_60040415_220000_CN_60040606_220000/LConn1
  _CN_48050742_220000_CN_60040415_220000/RConn2 -- T_60040415_220000_ОРУ___ГПП_1/LConn2 -- _CN_60040415_220000_CN_60040606_220000/LConn2
  _CN_48050742_220000_CN_60040415_220000/RConn3 -- T_60040415_220000_ОРУ___ГПП_1/LConn3 -- _CN_60040415_220000_CN_60040606_220000/LConn3 -- bus190/LConn1
  Д_5_CN_48050742_220000_CN_95996044_220000/RConn1 -- "T_95996044_220000;110000;10000_ПС_\"Левобережная\""/LConn1 -- _CN_95996044_220000_CN_202649908_220000/LConn1
  Д_5_CN_48050742_220000_CN_95996044_220000/RConn2 -- "T_95996044_220000;110000;10000_ПС_\"Левобережная\""/LConn2 -- _CN_95996044_220000_CN_202649908_220000/LConn2
  Д_5_CN_48050742_220000_CN_95996044_220000/RConn3 -- "T_95996044_220000;110000;10000_ПС_\"Левобережная\""/LConn3 -- _CN_95996044_220000_CN_202649908_220000/LConn3 -- bus191/LConn1
  _CN_48050742_220000_CN_305389785_220000/RConn1 -- "T_305389785_500000;220000_ПС_\"Енисей\""/RConn1 -- _CN_305389785_220000_CN_110542603_220000/RConn1 -- L_305389785/LConn1 -- _CN_305389785_220000_CN_60047767_110000/RConn1
  _CN_48050742_220000_CN_305389785_220000/RConn2 -- "T_305389785_500000;220000_ПС_\"Енисей\""/RConn2 -- _CN_305389785_220000_CN_110542603_220000/RConn2 -- L_305389785/LConn2 -- _CN_305389785_220000_CN_60047767_110000/RConn2
  _CN_48050742_220000_CN_305389785_220000/RConn3 -- "T_305389785_500000;220000_ПС_\"Енисей\""/RConn3 -- _CN_305389785_220000_CN_110542603_220000/RConn3 -- L_305389785/LConn3 -- bus192/LConn1 -- _CN_305389785_220000_CN_60047767_110000/RConn3
  "T_105828925_220000;110000;10000_ПС_\"Узловая\""/LConn1 -- Д_19___Д_20_CN_105828925_220000_CN_435735615_220000/LConn1
  "T_105828925_220000;110000;10000_ПС_\"Узловая\""/LConn2 -- Д_19___Д_20_CN_105828925_220000_CN_435735615_220000/LConn2
  Д_19___Д_20_CN_105828925_220000_CN_435735615_220000/LConn3 -- "T_105828925_220000;110000;10000_ПС_\"Узловая\""/LConn3 -- bus193/LConn1
  T_435735615_220000_ОРУ_220_кВ/LConn1 -- Д_19___Д_20_CN_105828925_220000_CN_435735615_220000/RConn1
  T_435735615_220000_ОРУ_220_кВ/LConn2 -- Д_19___Д_20_CN_105828925_220000_CN_435735615_220000/RConn2
  Д_19___Д_20_CN_105828925_220000_CN_435735615_220000/RConn3 -- T_435735615_220000_ОРУ_220_кВ/LConn3 -- bus194/LConn1
  _CN_168239171_220000_CN_221635306_220000/LConn1 -- T_168239171_220000_Подстанция_«Ужур»/LConn1 -- _CN_168239171_220000_CN_228972838_220000/LConn1
  _CN_168239171_220000_CN_221635306_220000/LConn2 -- T_168239171_220000_Подстанция_«Ужур»/LConn2 -- _CN_168239171_220000_CN_228972838_220000/LConn2
  _CN_168239171_220000_CN_221635306_220000/LConn3 -- T_168239171_220000_Подстанция_«Ужур»/LConn3 -- _CN_168239171_220000_CN_228972838_220000/LConn3 -- bus195/LConn1
  T_221635306__Подстанция_«Сорская»/LConn1 -- _CN_168239171_220000_CN_221635306_220000/RConn1
  T_221635306__Подстанция_«Сорская»/LConn2 -- _CN_168239171_220000_CN_221635306_220000/RConn2
  _CN_168239171_220000_CN_221635306_220000/RConn3 -- T_221635306__Подстанция_«Сорская»/LConn3 -- bus196/LConn1
  _CN_168239171_220000_CN_228972838_220000/RConn1 -- T_228972838__/LConn1 -- _CN_228972838_220000_CN_228960140_220000/LConn1
  _CN_168239171_220000_CN_228972838_220000/RConn2 -- T_228972838__/LConn2 -- _CN_228972838_220000_CN_228960140_220000/LConn2
  _CN_168239171_220000_CN_228972838_220000/RConn3 -- T_228972838__/LConn3 -- _CN_228972838_220000_CN_228960140_220000/LConn3 -- bus197/LConn1
  _CN_141629044_220000_CN_110601357_220000/LConn1 -- T_141629044_500000;220000;110000;10000_Тулун/RConn1 -- _CN_141629044_220000_CN_113629981_220000/LConn1
  _CN_141629044_220000_CN_110601357_220000/LConn2 -- T_141629044_500000;220000;110000;10000_Тулун/RConn2 -- _CN_141629044_220000_CN_113629981_220000/LConn2
  _CN_141629044_220000_CN_110601357_220000/LConn3 -- T_141629044_500000;220000;110000;10000_Тулун/RConn3 -- _CN_141629044_220000_CN_113629981_220000/LConn3 -- bus198/LConn1
  _CN_141629044_220000_CN_110601357_220000/RConn1 -- T_110601357_500000;220000_/RConn1 -- _CN_110601357_220000_CN_113629981_220000/LConn1 -- _CN_110601357_220000_CN_116489400_220000/LConn1 -- _CN_110601357_220000_CN_113555542_220000/RConn1 -- L_110601357/LConn1
  _CN_141629044_220000_CN_110601357_220000/RConn2 -- T_110601357_500000;220000_/RConn2 -- _CN_110601357_220000_CN_113629981_220000/LConn2 -- _CN_110601357_220000_CN_116489400_220000/LConn2 -- _CN_110601357_220000_CN_113555542_220000/RConn2 -- L_110601357/LConn2
  _CN_141629044_220000_CN_110601357_220000/RConn3 -- T_110601357_500000;220000_/RConn3 -- _CN_110601357_220000_CN_113629981_220000/LConn3 -- _CN_110601357_220000_CN_116489400_220000/LConn3 -- _CN_110601357_220000_CN_113555542_220000/RConn3 -- L_110601357/LConn3 -- bus199/LConn1
  _CN_141629044_220000_CN_113629981_220000/RConn1 -- T_113629981_220000;110000;35000;fixme_/LConn1 -- _CN_110601357_220000_CN_113629981_220000/RConn1
  _CN_141629044_220000_CN_113629981_220000/RConn2 -- T_113629981_220000;110000;35000;fixme_/LConn2 -- _CN_110601357_220000_CN_113629981_220000/RConn2
  _CN_141629044_220000_CN_113629981_220000/RConn3 -- T_113629981_220000;110000;35000;fixme_/LConn3 -- _CN_110601357_220000_CN_113629981_220000/RConn3 -- bus200/LConn1
  ЧП_223___ЧП_233_(ПС_«Чажемто»___ПС_«Парабель»)_CN_167241850_220000_CN_169356997_220000/LConn1 -- T_167241850_220000_Подстанция_«Парабель»/LConn1 -- ПВ_224___ПВ_234_(ПС_«Парабель»___ПС_«Вертикос»)_CN_167241850_220000_CN_228023756_220000/LConn1
  ЧП_223___ЧП_233_(ПС_«Чажемто»___ПС_«Парабель»)_CN_167241850_220000_CN_169356997_220000/LConn2 -- T_167241850_220000_Подстанция_«Парабель»/LConn2 -- ПВ_224___ПВ_234_(ПС_«Парабель»___ПС_«Вертикос»)_CN_167241850_220000_CN_228023756_220000/LConn2
  ЧП_223___ЧП_233_(ПС_«Чажемто»___ПС_«Парабель»)_CN_167241850_220000_CN_169356997_220000/LConn3 -- T_167241850_220000_Подстанция_«Парабель»/LConn3 -- ПВ_224___ПВ_234_(ПС_«Парабель»___ПС_«Вертикос»)_CN_167241850_220000_CN_228023756_220000/LConn3 -- bus201/LConn1
  ЧП_223___ЧП_233_(ПС_«Чажемто»___ПС_«Парабель»)_CN_167241850_220000_CN_169356997_220000/RConn1 -- T_169356997_220000_Подстанция_«Чажемто_220»/LConn1 -- ВЧ_222___ВЧ_232_(ПС_«Володино»___ПС_«Чажемто»)_CN_169356997_220000_CN_189871845_220000/LConn1
  ЧП_223___ЧП_233_(ПС_«Чажемто»___ПС_«Парабель»)_CN_167241850_220000_CN_169356997_220000/RConn2 -- T_169356997_220000_Подстанция_«Чажемто_220»/LConn2 -- ВЧ_222___ВЧ_232_(ПС_«Володино»___ПС_«Чажемто»)_CN_169356997_220000_CN_189871845_220000/LConn2
  ЧП_223___ЧП_233_(ПС_«Чажемто»___ПС_«Парабель»)_CN_167241850_220000_CN_169356997_220000/RConn3 -- T_169356997_220000_Подстанция_«Чажемто_220»/LConn3 -- ВЧ_222___ВЧ_232_(ПС_«Володино»___ПС_«Чажемто»)_CN_169356997_220000_CN_189871845_220000/LConn3 -- bus202/LConn1
  T_228023756_220000_Подстанция_«Вертикос»/LConn1 -- ПВ_224___ПВ_234_(ПС_«Парабель»___ПС_«Вертикос»)_CN_167241850_220000_CN_228023756_220000/RConn1
  T_228023756_220000_Подстанция_«Вертикос»/LConn2 -- ПВ_224___ПВ_234_(ПС_«Парабель»___ПС_«Вертикос»)_CN_167241850_220000_CN_228023756_220000/RConn2
  ПВ_224___ПВ_234_(ПС_«Парабель»___ПС_«Вертикос»)_CN_167241850_220000_CN_228023756_220000/RConn3 -- T_228023756_220000_Подстанция_«Вертикос»/LConn3 -- bus203/LConn1
  T_245816959__/LConn1 -- _CN_245816959_220000_CN_82361665_220000/LConn1
  T_245816959__/LConn2 -- _CN_245816959_220000_CN_82361665_220000/LConn2
  _CN_245816959_220000_CN_82361665_220000/LConn3 -- T_245816959__/LConn3 -- bus204/LConn1
  _CN_245816959_220000_CN_82361665_220000/RConn1 -- T_82361665_500000_Означенное/RConn1 -- L_82361665/LConn1
  _CN_245816959_220000_CN_82361665_220000/RConn2 -- T_82361665_500000_Означенное/RConn2 -- L_82361665/LConn2
  _CN_245816959_220000_CN_82361665_220000/RConn3 -- T_82361665_500000_Означенное/RConn3 -- L_82361665/LConn3 -- bus205/LConn1
  T_60040328_220000_ОРУ___ГПП_4/LConn1 -- _CN_60040328_220000_CN_220574879_220000/RConn1
  T_60040328_220000_ОРУ___ГПП_4/LConn2 -- _CN_60040328_220000_CN_220574879_220000/RConn2
  _CN_60040328_220000_CN_220574879_220000/RConn3 -- T_60040328_220000_ОРУ___ГПП_4/LConn3 -- bus206/LConn1
  "T_202649908_220000;110000;10000_ПС_\"Октябрьская\""/LConn1 -- _CN_95996044_220000_CN_202649908_220000/RConn1
  "T_202649908_220000;110000;10000_ПС_\"Октябрьская\""/LConn2 -- _CN_95996044_220000_CN_202649908_220000/RConn2
  _CN_95996044_220000_CN_202649908_220000/RConn3 -- "T_202649908_220000;110000;10000_ПС_\"Октябрьская\""/LConn3 -- bus207/LConn1
  T_116489400__/LConn1 -- _CN_110601357_220000_CN_116489400_220000/RConn1
  T_116489400__/LConn2 -- _CN_110601357_220000_CN_116489400_220000/RConn2
  _CN_110601357_220000_CN_116489400_220000/RConn3 -- T_116489400__/LConn3 -- bus208/LConn1
  _CN_220574879_220000_CN_60040606_220000/RConn1 -- T_60040606_220000_ОРУ___ГПП_2/LConn1 -- _CN_60040415_220000_CN_60040606_220000/RConn1
  _CN_220574879_220000_CN_60040606_220000/RConn2 -- T_60040606_220000_ОРУ___ГПП_2/LConn2 -- _CN_60040415_220000_CN_60040606_220000/RConn2
  _CN_220574879_220000_CN_60040606_220000/RConn3 -- T_60040606_220000_ОРУ___ГПП_2/LConn3 -- _CN_60040415_220000_CN_60040606_220000/RConn3 -- bus209/LConn1
  АТ_216_Т_208_(ПС_«Новоанжерская»___ПС_«Восточная»___ПС_«Зональная»___ПС_«Восточная»)_CN_77195444_220000_CN_123874057_220000/LConn1 -- T_77195444_220000_Подстанция_«Восточная»/LConn1 -- Т_203_Т_204_(ПС_«Томская»___ПС_«Восточная»)_CN_77195444_220000_CN_341189940_220000/LConn1 -- Т_203_Т_204_(ПС_«Томская»___ПС_«Восточная»)_CN_77195444_220000_CN_166018985_220000/RConn1 -- Т_201_Т_202_(ПС_«Восточная»___ТЭЦ_СХК___ПС_«Восточная»___ЭС_2_СХК)_CN_77195444_220000_CN_166616387_220000/LConn1
  АТ_216_Т_208_(ПС_«Новоанжерская»___ПС_«Восточная»___ПС_«Зональная»___ПС_«Восточная»)_CN_77195444_220000_CN_123874057_220000/LConn2 -- T_77195444_220000_Подстанция_«Восточная»/LConn2 -- Т_203_Т_204_(ПС_«Томская»___ПС_«Восточная»)_CN_77195444_220000_CN_341189940_220000/LConn2 -- Т_203_Т_204_(ПС_«Томская»___ПС_«Восточная»)_CN_77195444_220000_CN_166018985_220000/RConn2 -- Т_201_Т_202_(ПС_«Восточная»___ТЭЦ_СХК___ПС_«Восточная»___ЭС_2_СХК)_CN_77195444_220000_CN_166616387_220000/LConn2
  АТ_216_Т_208_(ПС_«Новоанжерская»___ПС_«Восточная»___ПС_«Зональная»___ПС_«Восточная»)_CN_77195444_220000_CN_123874057_220000/LConn3 -- T_77195444_220000_Подстанция_«Восточная»/LConn3 -- Т_203_Т_204_(ПС_«Томская»___ПС_«Восточная»)_CN_77195444_220000_CN_341189940_220000/LConn3 -- Т_203_Т_204_(ПС_«Томская»___ПС_«Восточная»)_CN_77195444_220000_CN_166018985_220000/RConn3 -- Т_201_Т_202_(ПС_«Восточная»___ТЭЦ_СХК___ПС_«Восточная»___ЭС_2_СХК)_CN_77195444_220000_CN_166616387_220000/LConn3 -- bus210/LConn1
  T_123874057_220000_Подстанция_«Зональная»/LConn1 -- АТ_216_Т_208_(ПС_«Новоанжерская»___ПС_«Восточная»___ПС_«Зональная»___ПС_«Восточная»)_CN_77195444_220000_CN_123874057_220000/RConn1
  T_123874057_220000_Подстанция_«Зональная»/LConn2 -- АТ_216_Т_208_(ПС_«Новоанжерская»___ПС_«Восточная»___ПС_«Зональная»___ПС_«Восточная»)_CN_77195444_220000_CN_123874057_220000/RConn2
  АТ_216_Т_208_(ПС_«Новоанжерская»___ПС_«Восточная»___ПС_«Зональная»___ПС_«Восточная»)_CN_77195444_220000_CN_123874057_220000/RConn3 -- T_123874057_220000_Подстанция_«Зональная»/LConn3 -- bus211/LConn1
  T_341189940__/LConn1 -- Т_203_Т_204_(ПС_«Томская»___ПС_«Восточная»)_CN_77195444_220000_CN_341189940_220000/RConn1
  T_341189940__/LConn2 -- Т_203_Т_204_(ПС_«Томская»___ПС_«Восточная»)_CN_77195444_220000_CN_341189940_220000/RConn2
  Т_203_Т_204_(ПС_«Томская»___ПС_«Восточная»)_CN_77195444_220000_CN_341189940_220000/RConn3 -- T_341189940__/LConn3 -- bus212/LConn1
  T_166616387__ЭС_2_СХК/LConn1 -- Т_201_Т_202_(ПС_«Восточная»___ТЭЦ_СХК___ПС_«Восточная»___ЭС_2_СХК)_CN_77195444_220000_CN_166616387_220000/RConn1
  T_166616387__ЭС_2_СХК/LConn2 -- Т_201_Т_202_(ПС_«Восточная»___ТЭЦ_СХК___ПС_«Восточная»___ЭС_2_СХК)_CN_77195444_220000_CN_166616387_220000/RConn2
  Т_201_Т_202_(ПС_«Восточная»___ТЭЦ_СХК___ПС_«Восточная»___ЭС_2_СХК)_CN_77195444_220000_CN_166616387_220000/RConn3 -- T_166616387__ЭС_2_СХК/LConn3 -- bus213/LConn1
  ВЧ_222___ВЧ_232_(ПС_«Володино»___ПС_«Чажемто»)_CN_169356997_220000_CN_189871845_220000/RConn1 -- T_189871845_220000_Подстанция_«Володино_220»/LConn1 -- Т_219___Т_220_(ПС_«Володино_220»___ПС_«Мельниково_220»)_CN_189871845_220000_CN_169671124_220000/LConn1
  ВЧ_222___ВЧ_232_(ПС_«Володино»___ПС_«Чажемто»)_CN_169356997_220000_CN_189871845_220000/RConn2 -- T_189871845_220000_Подстанция_«Володино_220»/LConn2 -- Т_219___Т_220_(ПС_«Володино_220»___ПС_«Мельниково_220»)_CN_189871845_220000_CN_169671124_220000/LConn2
  ВЧ_222___ВЧ_232_(ПС_«Володино»___ПС_«Чажемто»)_CN_169356997_220000_CN_189871845_220000/RConn3 -- T_189871845_220000_Подстанция_«Володино_220»/LConn3 -- Т_219___Т_220_(ПС_«Володино_220»___ПС_«Мельниково_220»)_CN_189871845_220000_CN_169671124_220000/LConn3 -- bus214/LConn1
  T_169671124_220000_Подстанция_«Мельниково_220»/LConn1 -- Т_219___Т_220_(ПС_«Володино_220»___ПС_«Мельниково_220»)_CN_189871845_220000_CN_169671124_220000/RConn1
  T_169671124_220000_Подстанция_«Мельниково_220»/LConn2 -- Т_219___Т_220_(ПС_«Володино_220»___ПС_«Мельниково_220»)_CN_189871845_220000_CN_169671124_220000/RConn2
  Т_219___Т_220_(ПС_«Володино_220»___ПС_«Мельниково_220»)_CN_189871845_220000_CN_169671124_220000/RConn3 -- T_169671124_220000_Подстанция_«Мельниково_220»/LConn3 -- bus215/LConn1
  T_131753194_220000;110000;10000_Абакан_Районная/LConn1 -- _CN_131753194_220000_CN_131753195_220000/LConn1
  T_131753194_220000;110000;10000_Абакан_Районная/LConn2 -- _CN_131753194_220000_CN_131753195_220000/LConn2
  _CN_131753194_220000_CN_131753195_220000/LConn3 -- T_131753194_220000;110000;10000_Абакан_Районная/LConn3 -- bus216/LConn1
  _CN_131753194_220000_CN_131753195_220000/RConn1 -- T_131753195_500000;220000;fixme_Подстанция_«Абаканская»/RConn1 -- _CN_131753195_220000_CN_115163974_220000/LConn1
  _CN_131753194_220000_CN_131753195_220000/RConn2 -- T_131753195_500000;220000;fixme_Подстанция_«Абаканская»/RConn2 -- _CN_131753195_220000_CN_115163974_220000/LConn2
  _CN_131753194_220000_CN_131753195_220000/RConn3 -- T_131753195_500000;220000;fixme_Подстанция_«Абаканская»/RConn3 -- _CN_131753195_220000_CN_115163974_220000/LConn3 -- bus217/LConn1
  T_115163974_220000_Подстанция_«Минусинск_Опорная»/LConn1 -- _CN_131753195_220000_CN_115163974_220000/RConn1
  T_115163974_220000_Подстанция_«Минусинск_Опорная»/LConn2 -- _CN_131753195_220000_CN_115163974_220000/RConn2
  _CN_131753195_220000_CN_115163974_220000/RConn3 -- T_115163974_220000_Подстанция_«Минусинск_Опорная»/LConn3 -- bus218/LConn1
  _CN_60040448_220000_CN_110542603_220000/RConn1 -- "T_60040448_220000_РПС_\"КРАМЗ\""/LConn1 -- _CN_60040448_220000_CN_308372785_220000/LConn1 -- _CN_60040448_220000_CN_308372786_220000/LConn1 -- _CN_60040448_220000_CN_60040627_220000/LConn1
  _CN_60040448_220000_CN_110542603_220000/RConn2 -- "T_60040448_220000_РПС_\"КРАМЗ\""/LConn2 -- _CN_60040448_220000_CN_308372785_220000/LConn2 -- _CN_60040448_220000_CN_308372786_220000/LConn2 -- _CN_60040448_220000_CN_60040627_220000/LConn2
  _CN_60040448_220000_CN_110542603_220000/RConn3 -- "T_60040448_220000_РПС_\"КРАМЗ\""/LConn3 -- _CN_60040448_220000_CN_308372785_220000/LConn3 -- _CN_60040448_220000_CN_308372786_220000/LConn3 -- _CN_60040448_220000_CN_60040627_220000/LConn3 -- bus219/LConn1
  T_308372785_220000_/LConn1 -- _CN_60040448_220000_CN_308372785_220000/RConn1
  T_308372785_220000_/LConn2 -- _CN_60040448_220000_CN_308372785_220000/RConn2
  _CN_60040448_220000_CN_308372785_220000/RConn3 -- T_308372785_220000_/LConn3 -- bus220/LConn1
  T_308372786_220000_/LConn1 -- _CN_60040448_220000_CN_308372786_220000/RConn1
  T_308372786_220000_/LConn2 -- _CN_60040448_220000_CN_308372786_220000/RConn2
  _CN_60040448_220000_CN_308372786_220000/RConn3 -- T_308372786_220000_/LConn3 -- bus221/LConn1
  T_60040627_220000_/LConn1 -- _CN_60040448_220000_CN_60040627_220000/RConn1
  T_60040627_220000_/LConn2 -- _CN_60040448_220000_CN_60040627_220000/RConn2
  _CN_60040448_220000_CN_60040627_220000/RConn3 -- T_60040627_220000_/LConn3 -- bus222/LConn1
  "T_81603854__ПС_220_кВ_\"Урожай\""/LConn1 -- _CN_81603854_220000_CN_88364440_220000/LConn1
  "T_81603854__ПС_220_кВ_\"Урожай\""/LConn2 -- _CN_81603854_220000_CN_88364440_220000/LConn2
  _CN_81603854_220000_CN_88364440_220000/LConn3 -- "T_81603854__ПС_220_кВ_\"Урожай\""/LConn3 -- bus223/LConn1
  T_88364440_220000_Подстанция_«Карасук_3_(тяговая)»/LConn1 -- _CN_81603854_220000_CN_88364440_220000/RConn1
  T_88364440_220000_Подстанция_«Карасук_3_(тяговая)»/LConn2 -- _CN_81603854_220000_CN_88364440_220000/RConn2
  _CN_81603854_220000_CN_88364440_220000/RConn3 -- T_88364440_220000_Подстанция_«Карасук_3_(тяговая)»/LConn3 -- bus224/LConn1
  _CN_240874260_220000_CN_267191160_220000/LConn1 -- T_240874260__/LConn1 -- _CN_240874260_220000_CN_290406343_220000/LConn1 -- _CN_240874260_220000_CN_271058766_220000/LConn1
  _CN_240874260_220000_CN_267191160_220000/LConn2 -- T_240874260__/LConn2 -- _CN_240874260_220000_CN_290406343_220000/LConn2 -- _CN_240874260_220000_CN_271058766_220000/LConn2
  _CN_240874260_220000_CN_267191160_220000/LConn3 -- T_240874260__/LConn3 -- _CN_240874260_220000_CN_290406343_220000/LConn3 -- _CN_240874260_220000_CN_271058766_220000/LConn3 -- bus225/LConn1
  T_267191160_220000;110000;10000_/LConn1 -- _CN_240874260_220000_CN_267191160_220000/RConn1
  T_267191160_220000;110000;10000_/LConn2 -- _CN_240874260_220000_CN_267191160_220000/RConn2
  _CN_240874260_220000_CN_267191160_220000/RConn3 -- T_267191160_220000;110000;10000_/LConn3 -- bus226/LConn1
  T_290406343__/LConn1 -- _CN_240874260_220000_CN_290406343_220000/RConn1
  T_290406343__/LConn2 -- _CN_240874260_220000_CN_290406343_220000/RConn2
  _CN_240874260_220000_CN_290406343_220000/RConn3 -- T_290406343__/LConn3 -- bus227/LConn1
  T_271058766__/LConn1 -- _CN_240874260_220000_CN_271058766_220000/RConn1
  T_271058766__/LConn2 -- _CN_240874260_220000_CN_271058766_220000/RConn2
  _CN_240874260_220000_CN_271058766_220000/RConn3 -- T_271058766__/LConn3 -- bus228/LConn1
  Т_213_(ПС_«Томская»___ПС_«ГПП_220»)_CN_162583841_220000_CN_166018985_220000/RConn1 -- T_162583841_220000_Подстанция_«ГПП_220»/LConn1 -- Т_211_Т_212_(ТЭЦ_3___ПС_«ГПП_220»)_CN_162583841_220000_CN_76228618_110000/RConn1 -- Т_214_(ЭС_2_СХК___ПС_«ГПП_220»)_CN_162583841_220000_CN_166616386_220000/LConn1
  Т_213_(ПС_«Томская»___ПС_«ГПП_220»)_CN_162583841_220000_CN_166018985_220000/RConn2 -- T_162583841_220000_Подстанция_«ГПП_220»/LConn2 -- Т_211_Т_212_(ТЭЦ_3___ПС_«ГПП_220»)_CN_162583841_220000_CN_76228618_110000/RConn2 -- Т_214_(ЭС_2_СХК___ПС_«ГПП_220»)_CN_162583841_220000_CN_166616386_220000/LConn2
  Т_213_(ПС_«Томская»___ПС_«ГПП_220»)_CN_162583841_220000_CN_166018985_220000/RConn3 -- T_162583841_220000_Подстанция_«ГПП_220»/LConn3 -- Т_211_Т_212_(ТЭЦ_3___ПС_«ГПП_220»)_CN_162583841_220000_CN_76228618_110000/RConn3 -- bus229/LConn1 -- Т_214_(ЭС_2_СХК___ПС_«ГПП_220»)_CN_162583841_220000_CN_166616386_220000/LConn3
  T_166616386__ЭС_2_СХК/LConn1 -- Т_214_(ЭС_2_СХК___ПС_«ГПП_220»)_CN_162583841_220000_CN_166616386_220000/RConn1
  T_166616386__ЭС_2_СХК/LConn2 -- Т_214_(ЭС_2_СХК___ПС_«ГПП_220»)_CN_162583841_220000_CN_166616386_220000/RConn2
  Т_214_(ЭС_2_СХК___ПС_«ГПП_220»)_CN_162583841_220000_CN_166616386_220000/RConn3 -- T_166616386__ЭС_2_СХК/LConn3 -- bus230/LConn1
  T_228960140__/LConn1 -- _CN_228972838_220000_CN_228960140_220000/RConn1
  T_228960140__/LConn2 -- _CN_228972838_220000_CN_228960140_220000/RConn2
  _CN_228972838_220000_CN_228960140_220000/RConn3 -- T_228960140__/LConn3 -- bus231/LConn1
  T_60040659_220000_ОРУ___ГПП_6/LConn1 -- _CN_60040500_220000_CN_60040659_220000/RConn1
  T_60040659_220000_ОРУ___ГПП_6/LConn2 -- _CN_60040500_220000_CN_60040659_220000/RConn2
  _CN_60040500_220000_CN_60040659_220000/RConn3 -- T_60040659_220000_ОРУ___ГПП_6/LConn3 -- bus232/LConn1
  T_191588676_220000_Подстанция_«Чапаевка»/LConn1 -- _CN_191588676_220000_CN_130503101_220000/LConn1
  T_191588676_220000_Подстанция_«Чапаевка»/LConn2 -- _CN_191588676_220000_CN_130503101_220000/LConn2
  _CN_191588676_220000_CN_130503101_220000/LConn3 -- T_191588676_220000_Подстанция_«Чапаевка»/LConn3 -- bus233/LConn1
  _CN_191588676_220000_CN_130503101_220000/RConn1 -- T_130503101_220000_Подстанция_«Советско_Соснинская»/LConn1 -- _CN_130503101_220000_CN_68522408_220000/LConn1
  _CN_191588676_220000_CN_130503101_220000/RConn2 -- T_130503101_220000_Подстанция_«Советско_Соснинская»/LConn2 -- _CN_130503101_220000_CN_68522408_220000/LConn2
  _CN_191588676_220000_CN_130503101_220000/RConn3 -- T_130503101_220000_Подстанция_«Советско_Соснинская»/LConn3 -- _CN_130503101_220000_CN_68522408_220000/LConn3 -- bus234/LConn1
  G_68522408_Нижневартовская_ГРЭС/RConn1 -- _CN_130503101_220000_CN_68522408_220000/RConn1
  G_68522408_Нижневартовская_ГРЭС/RConn2 -- _CN_130503101_220000_CN_68522408_220000/RConn2
  _CN_130503101_220000_CN_68522408_220000/RConn3 -- G_68522408_Нижневартовская_ГРЭС/RConn3 -- bus235/LConn1
  ВЛ_?_(ПС_«Означенное»___ПС_«Алюминиевая»)_CN_223947264_500000_CN_82361665_500000/LConn1 -- T_223947264_500000_Подстанция_«Алюминиевая»/LConn1 -- ВЛ_?_(ПС_«Абаканская»___ПС_«Алюминиевая»)_CN_223947264_500000_CN_131753195_500000/LConn1
  ВЛ_?_(ПС_«Означенное»___ПС_«Алюминиевая»)_CN_223947264_500000_CN_82361665_500000/LConn2 -- T_223947264_500000_Подстанция_«Алюминиевая»/LConn2 -- ВЛ_?_(ПС_«Абаканская»___ПС_«Алюминиевая»)_CN_223947264_500000_CN_131753195_500000/LConn2
  ВЛ_?_(ПС_«Означенное»___ПС_«Алюминиевая»)_CN_223947264_500000_CN_82361665_500000/LConn3 -- T_223947264_500000_Подстанция_«Алюминиевая»/LConn3 -- ВЛ_?_(ПС_«Абаканская»___ПС_«Алюминиевая»)_CN_223947264_500000_CN_131753195_500000/LConn3 -- bus236/LConn1
  ВЛ_?_(ПС_«Означенное»___ПС_«Алюминиевая»)_CN_223947264_500000_CN_82361665_500000/RConn1 -- T_82361665_500000_Означенное/LConn1 -- ВЛ_543_(или_ВЛ_544)_(Саяно_Шушенская_ГЭС___ПС_«Означенное»)_CN_227781922_500000_CN_82361665_500000/LConn1
  ВЛ_?_(ПС_«Означенное»___ПС_«Алюминиевая»)_CN_223947264_500000_CN_82361665_500000/RConn2 -- T_82361665_500000_Означенное/LConn2 -- ВЛ_543_(или_ВЛ_544)_(Саяно_Шушенская_ГЭС___ПС_«Означенное»)_CN_227781922_500000_CN_82361665_500000/LConn2
  ВЛ_?_(ПС_«Означенное»___ПС_«Алюминиевая»)_CN_223947264_500000_CN_82361665_500000/RConn3 -- T_82361665_500000_Означенное/LConn3 -- ВЛ_543_(или_ВЛ_544)_(Саяно_Шушенская_ГЭС___ПС_«Означенное»)_CN_227781922_500000_CN_82361665_500000/LConn3 -- bus237/LConn1
  T_131753195_500000;220000;fixme_Подстанция_«Абаканская»/LConn1 -- ВЛ_?_(ПС_«Абаканская»___ПС_«Алюминиевая»)_CN_223947264_500000_CN_131753195_500000/RConn1
  T_131753195_500000;220000;fixme_Подстанция_«Абаканская»/LConn2 -- ВЛ_?_(ПС_«Абаканская»___ПС_«Алюминиевая»)_CN_223947264_500000_CN_131753195_500000/RConn2
  ВЛ_?_(ПС_«Абаканская»___ПС_«Алюминиевая»)_CN_223947264_500000_CN_131753195_500000/RConn3 -- T_131753195_500000;220000;fixme_Подстанция_«Абаканская»/LConn3 -- bus238/LConn1
  T_227781890_500000_КРУЭ_500_кВ/LConn1 -- _CN_227781890_500000_CN_227781922_500000/LConn1
  T_227781890_500000_КРУЭ_500_кВ/LConn2 -- _CN_227781890_500000_CN_227781922_500000/LConn2
  _CN_227781890_500000_CN_227781922_500000/LConn3 -- T_227781890_500000_КРУЭ_500_кВ/LConn3 -- bus239/LConn1
  _CN_227781890_500000_CN_227781922_500000/RConn1 -- T_227781922_500000_ОРУ_500_кВ/LConn1 -- ВЛ_541_(Саяно_Шушенская_ГЭС___ПС_«Новокузнецкая»)_CN_227781922_500000_CN_157280374_500000/LConn1 -- ВЛ_543_(или_ВЛ_544)_(Саяно_Шушенская_ГЭС___ПС_«Означенное»)_CN_227781922_500000_CN_82361665_500000/RConn1
  _CN_227781890_500000_CN_227781922_500000/RConn2 -- T_227781922_500000_ОРУ_500_кВ/LConn2 -- ВЛ_541_(Саяно_Шушенская_ГЭС___ПС_«Новокузнецкая»)_CN_227781922_500000_CN_157280374_500000/LConn2 -- ВЛ_543_(или_ВЛ_544)_(Саяно_Шушенская_ГЭС___ПС_«Означенное»)_CN_227781922_500000_CN_82361665_500000/RConn2
  _CN_227781890_500000_CN_227781922_500000/RConn3 -- T_227781922_500000_ОРУ_500_кВ/LConn3 -- ВЛ_541_(Саяно_Шушенская_ГЭС___ПС_«Новокузнецкая»)_CN_227781922_500000_CN_157280374_500000/LConn3 -- ВЛ_543_(или_ВЛ_544)_(Саяно_Шушенская_ГЭС___ПС_«Означенное»)_CN_227781922_500000_CN_82361665_500000/RConn3 -- bus240/LConn1
  _CN_110601357_500000_CN_225711294_500000/LConn1 -- T_110601357_500000;220000_/LConn1 -- _CN_110601357_500000_CN_113557354_500000/LConn1 -- _CN_110601357_500000_CN_141629044_500000/LConn1
  _CN_110601357_500000_CN_225711294_500000/LConn2 -- T_110601357_500000;220000_/LConn2 -- _CN_110601357_500000_CN_113557354_500000/LConn2 -- _CN_110601357_500000_CN_141629044_500000/LConn2
  _CN_110601357_500000_CN_225711294_500000/LConn3 -- T_110601357_500000;220000_/LConn3 -- _CN_110601357_500000_CN_113557354_500000/LConn3 -- bus241/LConn1 -- _CN_110601357_500000_CN_141629044_500000/LConn3
  _CN_110601357_500000_CN_225711294_500000/RConn1 -- T_225711294_500000;220000_Братский_переключательный_пункт/LConn1 -- _CN_131767848_500000_CN_225711294_500000/LConn1 -- _CN_225711294_500000_CN_141629044_500000/LConn1
  _CN_110601357_500000_CN_225711294_500000/RConn2 -- T_225711294_500000;220000_Братский_переключательный_пункт/LConn2 -- _CN_131767848_500000_CN_225711294_500000/LConn2 -- _CN_225711294_500000_CN_141629044_500000/LConn2
  _CN_110601357_500000_CN_225711294_500000/RConn3 -- T_225711294_500000;220000_Братский_переключательный_пункт/LConn3 -- _CN_131767848_500000_CN_225711294_500000/LConn3 -- _CN_225711294_500000_CN_141629044_500000/LConn3 -- bus242/LConn1
  _CN_110601357_500000_CN_141629044_500000/RConn1 -- T_141629044_500000;220000;110000;10000_Тулун/LConn1 -- _CN_110796857_500000_CN_141629044_500000/LConn1 -- _CN_225711294_500000_CN_141629044_500000/RConn1 -- _CN_228246728_500000_CN_141629044_500000/LConn1
  _CN_110601357_500000_CN_141629044_500000/RConn2 -- T_141629044_500000;220000;110000;10000_Тулун/LConn2 -- _CN_110796857_500000_CN_141629044_500000/LConn2 -- _CN_225711294_500000_CN_141629044_500000/RConn2 -- _CN_228246728_500000_CN_141629044_500000/LConn2
  _CN_110601357_500000_CN_141629044_500000/RConn3 -- T_141629044_500000;220000;110000;10000_Тулун/LConn3 -- _CN_110796857_500000_CN_141629044_500000/LConn3 -- _CN_225711294_500000_CN_141629044_500000/RConn3 -- _CN_228246728_500000_CN_141629044_500000/LConn3 -- bus243/LConn1
  G_113557354_Братская_ГЭС/RConn1 -- _CN_110601357_500000_CN_113557354_500000/RConn1
  G_113557354_Братская_ГЭС/RConn2 -- _CN_110601357_500000_CN_113557354_500000/RConn2
  _CN_110601357_500000_CN_113557354_500000/RConn3 -- G_113557354_Братская_ГЭС/RConn3 -- bus244/LConn1
  ВЛ_541_(Саяно_Шушенская_ГЭС___ПС_«Новокузнецкая»)_CN_227781922_500000_CN_157280374_500000/RConn1 -- T_157280374_500000_ПС_Новокузнецкая_500_кВ/LConn1 -- ВЛ_540_(ПС_«Барнаульская»___ПС_«Новокузнецкая»)_CN_100584147_500000_CN_157280374_500000/LConn1
  ВЛ_541_(Саяно_Шушенская_ГЭС___ПС_«Новокузнецкая»)_CN_227781922_500000_CN_157280374_500000/RConn2 -- T_157280374_500000_ПС_Новокузнецкая_500_кВ/LConn2 -- ВЛ_540_(ПС_«Барнаульская»___ПС_«Новокузнецкая»)_CN_100584147_500000_CN_157280374_500000/LConn2
  ВЛ_541_(Саяно_Шушенская_ГЭС___ПС_«Новокузнецкая»)_CN_227781922_500000_CN_157280374_500000/RConn3 -- T_157280374_500000_ПС_Новокузнецкая_500_кВ/LConn3 -- ВЛ_540_(ПС_«Барнаульская»___ПС_«Новокузнецкая»)_CN_100584147_500000_CN_157280374_500000/LConn3 -- bus245/LConn1
  _CN_131767848_500000_CN_105831607_500000/LConn1 -- T_131767848_500000;110000;35000_Тайшет/LConn1 -- _CN_131767848_500000_CN_225711294_500000/RConn1
  _CN_131767848_500000_CN_105831607_500000/LConn2 -- T_131767848_500000;110000;35000_Тайшет/LConn2 -- _CN_131767848_500000_CN_225711294_500000/RConn2
  _CN_131767848_500000_CN_105831607_500000/LConn3 -- T_131767848_500000;110000;35000_Тайшет/LConn3 -- _CN_131767848_500000_CN_225711294_500000/RConn3 -- bus246/LConn1
  _CN_131767848_500000_CN_105831607_500000/RConn1 -- T_105831607__Камала_1/LConn1 -- _CN_48050741_500000_CN_105831607_500000/LConn1
  _CN_131767848_500000_CN_105831607_500000/RConn2 -- T_105831607__Камала_1/LConn2 -- _CN_48050741_500000_CN_105831607_500000/LConn2
  _CN_131767848_500000_CN_105831607_500000/RConn3 -- T_105831607__Камала_1/LConn3 -- _CN_48050741_500000_CN_105831607_500000/LConn3 -- bus247/LConn1
  T_97377449_500000_Подстанция_«Барабинская»/LConn1 -- ВЛ_534_(ПС_«Барабинская»___ПС_«Таврическая»)_CN_97377449_500000_CN_107673466_500000/LConn1
  T_97377449_500000_Подстанция_«Барабинская»/LConn2 -- ВЛ_534_(ПС_«Барабинская»___ПС_«Таврическая»)_CN_97377449_500000_CN_107673466_500000/LConn2
  ВЛ_534_(ПС_«Барабинская»___ПС_«Таврическая»)_CN_97377449_500000_CN_107673466_500000/LConn3 -- T_97377449_500000_Подстанция_«Барабинская»/LConn3 -- bus248/LConn1
  ВЛ_534_(ПС_«Барабинская»___ПС_«Таврическая»)_CN_97377449_500000_CN_107673466_500000/RConn1 -- T_107673466_500000;220000_Подстанция_«Таврическая»/LConn1 -- ВЛ_555_(ПС_«Иртышская»___ПС_«Таврическая»)_CN_122224559_500000_CN_107673466_500000/LConn1
  ВЛ_534_(ПС_«Барабинская»___ПС_«Таврическая»)_CN_97377449_500000_CN_107673466_500000/RConn2 -- T_107673466_500000;220000_Подстанция_«Таврическая»/LConn2 -- ВЛ_555_(ПС_«Иртышская»___ПС_«Таврическая»)_CN_122224559_500000_CN_107673466_500000/LConn2
  ВЛ_534_(ПС_«Барабинская»___ПС_«Таврическая»)_CN_97377449_500000_CN_107673466_500000/RConn3 -- T_107673466_500000;220000_Подстанция_«Таврическая»/LConn3 -- ВЛ_555_(ПС_«Иртышская»___ПС_«Таврическая»)_CN_122224559_500000_CN_107673466_500000/LConn3 -- bus249/LConn1
  T_100584107_500000_Подстанция_«Алтай»/LConn1 -- ВЛ_595_(или_596)_(ПС_«Алтай»___ПС_«Барнаульская»)_CN_100584107_500000_CN_100584147_500000/LConn1
  T_100584107_500000_Подстанция_«Алтай»/LConn2 -- ВЛ_595_(или_596)_(ПС_«Алтай»___ПС_«Барнаульская»)_CN_100584107_500000_CN_100584147_500000/LConn2
  ВЛ_595_(или_596)_(ПС_«Алтай»___ПС_«Барнаульская»)_CN_100584107_500000_CN_100584147_500000/LConn3 -- T_100584107_500000_Подстанция_«Алтай»/LConn3 -- bus250/LConn1
  ВЛ_595_(или_596)_(ПС_«Алтай»___ПС_«Барнаульская»)_CN_100584107_500000_CN_100584147_500000/RConn1 -- T_100584147_500000_Подстанция_«Барнаульская»/LConn1 -- ВЛ_540_(ПС_«Барнаульская»___ПС_«Новокузнецкая»)_CN_100584147_500000_CN_157280374_500000/RConn1
  ВЛ_595_(или_596)_(ПС_«Алтай»___ПС_«Барнаульская»)_CN_100584107_500000_CN_100584147_500000/RConn2 -- T_100584147_500000_Подстанция_«Барнаульская»/LConn2 -- ВЛ_540_(ПС_«Барнаульская»___ПС_«Новокузнецкая»)_CN_100584147_500000_CN_157280374_500000/RConn2
  ВЛ_595_(или_596)_(ПС_«Алтай»___ПС_«Барнаульская»)_CN_100584107_500000_CN_100584147_500000/RConn3 -- T_100584147_500000_Подстанция_«Барнаульская»/LConn3 -- ВЛ_540_(ПС_«Барнаульская»___ПС_«Новокузнецкая»)_CN_100584147_500000_CN_157280374_500000/RConn3 -- bus251/LConn1
  "T_122224559_500000;220000;110000_ПС_500_кВ_\"Иртышская\""/LConn1 -- ВЛ_555_(ПС_«Иртышская»___ПС_«Таврическая»)_CN_122224559_500000_CN_107673466_500000/RConn1
  "T_122224559_500000;220000;110000_ПС_500_кВ_\"Иртышская\""/LConn2 -- ВЛ_555_(ПС_«Иртышская»___ПС_«Таврическая»)_CN_122224559_500000_CN_107673466_500000/RConn2
  ВЛ_555_(ПС_«Иртышская»___ПС_«Таврическая»)_CN_122224559_500000_CN_107673466_500000/RConn3 -- "T_122224559_500000;220000;110000_ПС_500_кВ_\"Иртышская\""/LConn3 -- bus252/LConn1
  _CN_48050741_500000_CN_105831607_500000/RConn1 -- "T_48050741_500000;220000;35000;10000_ПС_\"Красноярская\""/LConn1 -- _CN_48050741_500000_CN_305389785_500000/LConn1
  _CN_48050741_500000_CN_105831607_500000/RConn2 -- "T_48050741_500000;220000;35000;10000_ПС_\"Красноярская\""/LConn2 -- _CN_48050741_500000_CN_305389785_500000/LConn2
  _CN_48050741_500000_CN_105831607_500000/RConn3 -- "T_48050741_500000;220000;35000;10000_ПС_\"Красноярская\""/LConn3 -- _CN_48050741_500000_CN_305389785_500000/LConn3 -- bus253/LConn1
  "T_305389785_500000;220000_ПС_\"Енисей\""/LConn1 -- _CN_48050741_500000_CN_305389785_500000/RConn1
  "T_305389785_500000;220000_ПС_\"Енисей\""/LConn2 -- _CN_48050741_500000_CN_305389785_500000/RConn2
  _CN_48050741_500000_CN_305389785_500000/RConn3 -- "T_305389785_500000;220000_ПС_\"Енисей\""/LConn3 -- bus254/LConn1
  _CN_110796857_500000_CN_141629044_500000/RConn1 -- "T_110796857__ПС_500_220_110_кВ_\"Иркутская\""/LConn1 -- _CN_110796857_500000_CN_228246728_500000/LConn1
  _CN_110796857_500000_CN_141629044_500000/RConn2 -- "T_110796857__ПС_500_220_110_кВ_\"Иркутская\""/LConn2 -- _CN_110796857_500000_CN_228246728_500000/LConn2
  _CN_110796857_500000_CN_141629044_500000/RConn3 -- "T_110796857__ПС_500_220_110_кВ_\"Иркутская\""/LConn3 -- _CN_110796857_500000_CN_228246728_500000/LConn3 -- bus255/LConn1
  _CN_110796857_500000_CN_228246728_500000/RConn1 -- T_228246728_500000;220000_/LConn1 -- _CN_228246728_500000_CN_41746137_500000/LConn1 -- _CN_228246728_500000_CN_141629044_500000/RConn1
  _CN_110796857_500000_CN_228246728_500000/RConn2 -- T_228246728_500000;220000_/LConn2 -- _CN_228246728_500000_CN_41746137_500000/LConn2 -- _CN_228246728_500000_CN_141629044_500000/RConn2
  _CN_110796857_500000_CN_228246728_500000/RConn3 -- T_228246728_500000;220000_/LConn3 -- _CN_228246728_500000_CN_41746137_500000/LConn3 -- bus256/LConn1 -- _CN_228246728_500000_CN_141629044_500000/RConn3
  G_41746137_Гусиноозёрская_ГРЭС/RConn1 -- _CN_228246728_500000_CN_41746137_500000/RConn1
  G_41746137_Гусиноозёрская_ГРЭС/RConn2 -- _CN_228246728_500000_CN_41746137_500000/RConn2
  _CN_228246728_500000_CN_41746137_500000/RConn3 -- G_41746137_Гусиноозёрская_ГРЭС/RConn3 -- bus257/LConn1
  "T_339272953_110000_ПС_\"Маркелово\""/RConn1 -- L_339272953/LConn1
  "T_339272953_110000_ПС_\"Маркелово\""/RConn2 -- L_339272953/LConn2
  L_339272953/LConn3 -- "T_339272953_110000_ПС_\"Маркелово\""/RConn3 -- bus258/LConn1
  T_173504267_110000_Подстанция_«Плотниково»/RConn1 -- L_173504267/LConn1
  T_173504267_110000_Подстанция_«Плотниково»/RConn2 -- L_173504267/LConn2
  L_173504267/LConn3 -- T_173504267_110000_Подстанция_«Плотниково»/RConn3 -- bus259/LConn1
  T_162573317_110000_Подстанция_«ГПП_14»/RConn1 -- L_162573317/LConn1
  T_162573317_110000_Подстанция_«ГПП_14»/RConn2 -- L_162573317/LConn2
  L_162573317/LConn3 -- T_162573317_110000_Подстанция_«ГПП_14»/RConn3 -- bus260/LConn1
  "T_197928455_110000_Тяговая_ПС_\"Тебисская\""/RConn1 -- L_197928455/LConn1
  "T_197928455_110000_Тяговая_ПС_\"Тебисская\""/RConn2 -- L_197928455/LConn2
  L_197928455/LConn3 -- "T_197928455_110000_Тяговая_ПС_\"Тебисская\""/RConn3 -- bus261/LConn1
  T_167875378__/RConn1 -- L_167875378/LConn1
  T_167875378__/RConn2 -- L_167875378/LConn2
  L_167875378/LConn3 -- T_167875378__/RConn3 -- bus262/LConn1
  T_107439685_110000_Подстанция_«Чаны»/RConn1 -- L_107439685/LConn1
  T_107439685_110000_Подстанция_«Чаны»/RConn2 -- L_107439685/LConn2
  L_107439685/LConn3 -- T_107439685_110000_Подстанция_«Чаны»/RConn3 -- bus263/LConn1
  T_172599304_110000_Подстанция_«Кривошеино»/RConn1 -- L_172599304/LConn1
  T_172599304_110000_Подстанция_«Кривошеино»/RConn2 -- L_172599304/LConn2
  L_172599304/LConn3 -- T_172599304_110000_Подстанция_«Кривошеино»/RConn3 -- bus264/LConn1
  T_190434443_110000_Подстанция_«Володино_110»/RConn1 -- L_190434443/LConn1
  T_190434443_110000_Подстанция_«Володино_110»/RConn2 -- L_190434443/LConn2
  L_190434443/LConn3 -- T_190434443_110000_Подстанция_«Володино_110»/RConn3 -- bus265/LConn1
  T_228847625_110000_Подстанция_«Ломовая»/RConn1 -- L_228847625/LConn1
  T_228847625_110000_Подстанция_«Ломовая»/RConn2 -- L_228847625/LConn2
  L_228847625/LConn3 -- T_228847625_110000_Подстанция_«Ломовая»/RConn3 -- bus266/LConn1
  "T_255013388_110000_ПС_№159_\"ХМЗ\""/RConn1 -- L_255013388/LConn1
  "T_255013388_110000_ПС_№159_\"ХМЗ\""/RConn2 -- L_255013388/LConn2
  L_255013388/LConn3 -- "T_255013388_110000_ПС_№159_\"ХМЗ\""/RConn3 -- bus267/LConn1
  T_435735618_110000_ОРУ_110_кВ/RConn1 -- L_435735618/LConn1
  T_435735618_110000_ОРУ_110_кВ/RConn2 -- L_435735618/LConn2
  L_435735618/LConn3 -- T_435735618_110000_ОРУ_110_кВ/RConn3 -- bus268/LConn1
  "T_59264203_110000;35000;10000_ПС_№103_\"Береговая\""/RConn1 -- L_59264203/LConn1
  "T_59264203_110000;35000;10000_ПС_№103_\"Береговая\""/RConn2 -- L_59264203/LConn2
  L_59264203/LConn3 -- "T_59264203_110000;35000;10000_ПС_№103_\"Береговая\""/RConn3 -- bus269/LConn1
  "T_60132693_110000;35000;6000_ПС_№101_\"Гидростроителей\""/RConn1 -- L_60132693/LConn1
  "T_60132693_110000;35000;6000_ПС_№101_\"Гидростроителей\""/RConn2 -- L_60132693/LConn2
  L_60132693/LConn3 -- "T_60132693_110000;35000;6000_ПС_№101_\"Гидростроителей\""/RConn3 -- bus270/LConn1
  T_227681298__/RConn1 -- L_227681298/LConn1
  T_227681298__/RConn2 -- L_227681298/LConn2
  L_227681298/LConn3 -- T_227681298__/RConn3 -- bus271/LConn1
  T_141629009__Нюра/RConn1 -- L_141629009/LConn1
  T_141629009__Нюра/RConn2 -- L_141629009/LConn2
  L_141629009/LConn3 -- T_141629009__Нюра/RConn3 -- bus272/LConn1
  T_256586292__/RConn1 -- L_256586292/LConn1
  T_256586292__/RConn2 -- L_256586292/LConn2
  L_256586292/LConn3 -- T_256586292__/RConn3 -- bus273/LConn1
  T_162544154_110000_Подстанция_«Октябрьская»/RConn1 -- L_162544154/LConn1
  T_162544154_110000_Подстанция_«Октябрьская»/RConn2 -- L_162544154/LConn2
  L_162544154/LConn3 -- T_162544154_110000_Подстанция_«Октябрьская»/RConn3 -- bus274/LConn1
  T_51505459__/RConn1 -- L_51505459/LConn1
  T_51505459__/RConn2 -- L_51505459/LConn2
  L_51505459/LConn3 -- T_51505459__/RConn3 -- bus275/LConn1
  "T_294641182_110000;10000_ПС_№_9_\"Центральная\""/RConn1 -- L_294641182/LConn1
  "T_294641182_110000;10000_ПС_№_9_\"Центральная\""/RConn2 -- L_294641182/LConn2
  L_294641182/LConn3 -- "T_294641182_110000;10000_ПС_№_9_\"Центральная\""/RConn3 -- bus276/LConn1
  "T_203496562_220000;210000;10000_ПС_\"Центр\""/RConn1 -- L_203496562/LConn1
  "T_203496562_220000;210000;10000_ПС_\"Центр\""/RConn2 -- L_203496562/LConn2
  L_203496562/LConn3 -- "T_203496562_220000;210000;10000_ПС_\"Центр\""/RConn3 -- bus277/LConn1
  "T_295466100_110000;10000_ПС_№5_\"Восточная\""/RConn1 -- L_295466100/LConn1
  "T_295466100_110000;10000_ПС_№5_\"Восточная\""/RConn2 -- L_295466100/LConn2
  L_295466100/LConn3 -- "T_295466100_110000;10000_ПС_№5_\"Восточная\""/RConn3 -- bus278/LConn1
  "T_123943720_110000;10000_ПС_№_33_\"Молодежная\""/RConn1 -- L_123943720/LConn1
  "T_123943720_110000;10000_ПС_№_33_\"Молодежная\""/RConn2 -- L_123943720/LConn2
  L_123943720/LConn3 -- "T_123943720_110000;10000_ПС_№_33_\"Молодежная\""/RConn3 -- bus279/LConn1
  T_167284772_110000_Подстанция_«Вороново»/RConn1 -- L_167284772/LConn1
  T_167284772_110000_Подстанция_«Вороново»/RConn2 -- L_167284772/LConn2
  L_167284772/LConn3 -- T_167284772_110000_Подстанция_«Вороново»/RConn3 -- bus280/LConn1
  T_165976042_110000_Подстанция_«Уртам»/RConn1 -- L_165976042/LConn1
  T_165976042_110000_Подстанция_«Уртам»/RConn2 -- L_165976042/LConn2
  L_165976042/LConn3 -- T_165976042_110000_Подстанция_«Уртам»/RConn3 -- bus281/LConn1
  T_131640871_110000_Подстанция_«Солнечная»/RConn1 -- L_131640871/LConn1
  T_131640871_110000_Подстанция_«Солнечная»/RConn2 -- L_131640871/LConn2
  L_131640871/LConn3 -- T_131640871_110000_Подстанция_«Солнечная»/RConn3 -- bus282/LConn1
  T_161501791_110000_Подстанция_«Коммунальная»/RConn1 -- L_161501791/LConn1
  T_161501791_110000_Подстанция_«Коммунальная»/RConn2 -- L_161501791/LConn2
  L_161501791/LConn3 -- T_161501791_110000_Подстанция_«Коммунальная»/RConn3 -- bus283/LConn1
  T_223481385__Тяговая_ПС/RConn1 -- L_223481385/LConn1
  T_223481385__Тяговая_ПС/RConn2 -- L_223481385/LConn2
  L_223481385/LConn3 -- T_223481385__Тяговая_ПС/RConn3 -- bus284/LConn1
  T_208172439_110000_Яшкино/RConn1 -- L_208172439/LConn1
  T_208172439_110000_Яшкино/RConn2 -- L_208172439/LConn2
  L_208172439/LConn3 -- T_208172439_110000_Яшкино/RConn3 -- bus285/LConn1
  "T_237781034__ПС_110_10_кВ_\"Стрела\""/RConn1 -- L_237781034/LConn1
  "T_237781034__ПС_110_10_кВ_\"Стрела\""/RConn2 -- L_237781034/LConn2
  L_237781034/LConn3 -- "T_237781034__ПС_110_10_кВ_\"Стрела\""/RConn3 -- bus286/LConn1
  "T_421135596_110000;35000;10000_ПС_\"Новоуральская\"_110_35_10"/RConn1 -- L_421135596/LConn1
  "T_421135596_110000;35000;10000_ПС_\"Новоуральская\"_110_35_10"/RConn2 -- L_421135596/LConn2
  L_421135596/LConn3 -- "T_421135596_110000;35000;10000_ПС_\"Новоуральская\"_110_35_10"/RConn3 -- bus287/LConn1
  T_228962860__/RConn1 -- L_228962860/LConn1
  T_228962860__/RConn2 -- L_228962860/LConn2
  L_228962860/LConn3 -- T_228962860__/RConn3 -- bus288/LConn1
  T_418072303__/RConn1 -- L_418072303/LConn1
  T_418072303__/RConn2 -- L_418072303/LConn2
  L_418072303/LConn3 -- T_418072303__/RConn3 -- bus289/LConn1
  T_180788791__/RConn1 -- L_180788791/LConn1
  T_180788791__/RConn2 -- L_180788791/LConn2
  L_180788791/LConn3 -- T_180788791__/RConn3 -- bus290/LConn1
  "T_178541618_110000;6000_ПС_№119_\"Мичуринская\""/RConn1 -- L_178541618/LConn1
  "T_178541618_110000;6000_ПС_№119_\"Мичуринская\""/RConn2 -- L_178541618/LConn2
  L_178541618/LConn3 -- "T_178541618_110000;6000_ПС_№119_\"Мичуринская\""/RConn3 -- bus291/LConn1
  T_201587851__/RConn1 -- L_201587851/LConn1
  T_201587851__/RConn2 -- L_201587851/LConn2
  L_201587851/LConn3 -- T_201587851__/RConn3 -- bus292/LConn1
  T_98731668_220000_Подстанция_«Районная»/RConn1 -- L_98731668/LConn1
  T_98731668_220000_Подстанция_«Районная»/RConn2 -- L_98731668/LConn2
  L_98731668/LConn3 -- T_98731668_220000_Подстанция_«Районная»/RConn3 -- bus293/LConn1
  T_184811446_110000_ПС_110_35_6_кВ_Прибрежная/RConn1 -- L_184811446/LConn1
  T_184811446_110000_ПС_110_35_6_кВ_Прибрежная/RConn2 -- L_184811446/LConn2
  L_184811446/LConn3 -- T_184811446_110000_ПС_110_35_6_кВ_Прибрежная/RConn3 -- bus294/LConn1
  T_184798669__ПС_110_35_6_кВ_ГПП_2/RConn1 -- L_184798669/LConn1
  T_184798669__ПС_110_35_6_кВ_ГПП_2/RConn2 -- L_184798669/LConn2
  L_184798669/LConn3 -- T_184798669__ПС_110_35_6_кВ_ГПП_2/RConn3 -- bus295/LConn1
  "T_283922783_110000;10000_ПС_№122_\"Северная\""/RConn1 -- L_283922783/LConn1
  "T_283922783_110000;10000_ПС_№122_\"Северная\""/RConn2 -- L_283922783/LConn2
  L_283922783/LConn3 -- "T_283922783_110000;10000_ПС_№122_\"Северная\""/RConn3 -- bus296/LConn1
  "T_225106390_110000;10000_ПС_№140_\"Аэропорт\""/RConn1 -- L_225106390/LConn1
  "T_225106390_110000;10000_ПС_№140_\"Аэропорт\""/RConn2 -- L_225106390/LConn2
  L_225106390/LConn3 -- "T_225106390_110000;10000_ПС_№140_\"Аэропорт\""/RConn3 -- bus297/LConn1
  T_95614050_110000;10000_/RConn1 -- L_95614050/LConn1
  T_95614050_110000;10000_/RConn2 -- L_95614050/LConn2
  L_95614050/LConn3 -- T_95614050_110000;10000_/RConn3 -- bus298/LConn1
  "T_255519517_110000;6000_ПС_\"Химволокно\""/RConn1 -- L_255519517/LConn1
  "T_255519517_110000;6000_ПС_\"Химволокно\""/RConn2 -- L_255519517/LConn2
  L_255519517/LConn3 -- "T_255519517_110000;6000_ПС_\"Химволокно\""/RConn3 -- bus299/LConn1
  "T_255519515_110000;6000_ПС_\"Цветные_металлы\""/RConn1 -- L_255519515/LConn1
  "T_255519515_110000;6000_ПС_\"Цветные_металлы\""/RConn2 -- L_255519515/LConn2
  L_255519515/LConn3 -- "T_255519515_110000;6000_ПС_\"Цветные_металлы\""/RConn3 -- bus300/LConn1
  "T_258257783_110000;10000_ПС_ГПП_1_\"КрасМаш\""/RConn1 -- L_258257783/LConn1
  "T_258257783_110000;10000_ПС_ГПП_1_\"КрасМаш\""/RConn2 -- L_258257783/LConn2
  L_258257783/LConn3 -- "T_258257783_110000;10000_ПС_ГПП_1_\"КрасМаш\""/RConn3 -- bus301/LConn1
  "T_328318277_110000;10000_ПС_ГПП_2_\"КрасМаш\""/RConn1 -- L_328318277/LConn1
  "T_328318277_110000;10000_ПС_ГПП_2_\"КрасМаш\""/RConn2 -- L_328318277/LConn2
  L_328318277/LConn3 -- "T_328318277_110000;10000_ПС_ГПП_2_\"КрасМаш\""/RConn3 -- bus302/LConn1
  T_255181608_110000_/RConn1 -- L_255181608/LConn1
  T_255181608_110000_/RConn2 -- L_255181608/LConn2
  L_255181608/LConn3 -- T_255181608_110000_/RConn3 -- bus303/LConn1
  "T_201620593_110000_Тяговая_ПС_\"Кабаклы\""/RConn1 -- L_201620593/LConn1
  "T_201620593_110000_Тяговая_ПС_\"Кабаклы\""/RConn2 -- L_201620593/LConn2
  L_201620593/LConn3 -- "T_201620593_110000_Тяговая_ПС_\"Кабаклы\""/RConn3 -- bus304/LConn1
  T_197934973_110000_Подстанция_«Валерино»/RConn1 -- L_197934973/LConn1
  T_197934973_110000_Подстанция_«Валерино»/RConn2 -- L_197934973/LConn2
  L_197934973/LConn3 -- T_197934973_110000_Подстанция_«Валерино»/RConn3 -- bus305/LConn1
  T_113306036__/RConn1 -- L_113306036/LConn1
  T_113306036__/RConn2 -- L_113306036/LConn2
  L_113306036/LConn3 -- T_113306036__/RConn3 -- bus306/LConn1
  T_197933918_110000_/RConn1 -- L_197933918/LConn1
  T_197933918_110000_/RConn2 -- L_197933918/LConn2
  L_197933918/LConn3 -- T_197933918_110000_/RConn3 -- bus307/LConn1
  T_201620594_110000_Подстанция_«Киевская»/RConn1 -- L_201620594/LConn1
  T_201620594_110000_Подстанция_«Киевская»/RConn2 -- L_201620594/LConn2
  L_201620594/LConn3 -- T_201620594_110000_Подстанция_«Киевская»/RConn3 -- bus308/LConn1
  T_167347786_110000_Подстанция_«Мельниково»/RConn1 -- L_167347786/LConn1
  T_167347786_110000_Подстанция_«Мельниково»/RConn2 -- L_167347786/LConn2
  L_167347786/LConn3 -- T_167347786_110000_Подстанция_«Мельниково»/RConn3 -- bus309/LConn1
  T_150289682_110000_Подстанция_«Левобережная»/RConn1 -- L_150289682/LConn1
  T_150289682_110000_Подстанция_«Левобережная»/RConn2 -- L_150289682/LConn2
  L_150289682/LConn3 -- T_150289682_110000_Подстанция_«Левобережная»/RConn3 -- bus310/LConn1
  T_169673998_110000_Подстанция_«Кожевниково»/RConn1 -- L_169673998/LConn1
  T_169673998_110000_Подстанция_«Кожевниково»/RConn2 -- L_169673998/LConn2
  L_169673998/LConn3 -- T_169673998_110000_Подстанция_«Кожевниково»/RConn3 -- bus311/LConn1
  T_220695627_110000_Подстанция_«Сайга»/RConn1 -- L_220695627/LConn1
  T_220695627_110000_Подстанция_«Сайга»/RConn2 -- L_220695627/LConn2
  L_220695627/LConn3 -- T_220695627_110000_Подстанция_«Сайга»/RConn3 -- bus312/LConn1
  T_202927834_110000_Подстанция_«Белый_Яр»/RConn1 -- L_202927834/LConn1
  T_202927834_110000_Подстанция_«Белый_Яр»/RConn2 -- L_202927834/LConn2
  L_202927834/LConn3 -- T_202927834_110000_Подстанция_«Белый_Яр»/RConn3 -- bus313/LConn1
  T_220695628_110000_Подстанция_«Ягодное»/RConn1 -- L_220695628/LConn1
  T_220695628_110000_Подстанция_«Ягодное»/RConn2 -- L_220695628/LConn2
  L_220695628/LConn3 -- T_220695628_110000_Подстанция_«Ягодное»/RConn3 -- bus314/LConn1
  "T_277861487_110000;10000_ПС_№126_\"Радиотехническая\""/RConn1 -- L_277861487/LConn1
  "T_277861487_110000;10000_ПС_№126_\"Радиотехническая\""/RConn2 -- L_277861487/LConn2
  L_277861487/LConn3 -- "T_277861487_110000;10000_ПС_№126_\"Радиотехническая\""/RConn3 -- bus315/LConn1
  "T_225106385_110000;35000;10000_ПС_№121_\"Мясокомбинат\""/RConn1 -- L_225106385/LConn1
  "T_225106385_110000;35000;10000_ПС_№121_\"Мясокомбинат\""/RConn2 -- L_225106385/LConn2
  L_225106385/LConn3 -- "T_225106385_110000;35000;10000_ПС_№121_\"Мясокомбинат\""/RConn3 -- bus316/LConn1
  "T_277861486_110000;10000_ПС_№183_\"Ботаническая\""/RConn1 -- L_277861486/LConn1
  "T_277861486_110000;10000_ПС_№183_\"Ботаническая\""/RConn2 -- L_277861486/LConn2
  L_277861486/LConn3 -- "T_277861486_110000;10000_ПС_№183_\"Ботаническая\""/RConn3 -- bus317/LConn1
  T_255772238_110000_ПС_БНС_ТЭЦ_2/RConn1 -- L_255772238/LConn1
  T_255772238_110000_ПС_БНС_ТЭЦ_2/RConn2 -- L_255772238/LConn2
  L_255772238/LConn3 -- T_255772238_110000_ПС_БНС_ТЭЦ_2/RConn3 -- bus318/LConn1
  "T_259338276_110000;6000_ПС_\"Железнодорожная\""/RConn1 -- L_259338276/LConn1
  "T_259338276_110000;6000_ПС_\"Железнодорожная\""/RConn2 -- L_259338276/LConn2
  L_259338276/LConn3 -- "T_259338276_110000;6000_ПС_\"Железнодорожная\""/RConn3 -- bus319/LConn1
  "T_202168526_110000;10000_ПС_№2_\"Советская\""/RConn1 -- L_202168526/LConn1
  "T_202168526_110000;10000_ПС_№2_\"Советская\""/RConn2 -- L_202168526/LConn2
  L_202168526/LConn3 -- "T_202168526_110000;10000_ПС_№2_\"Советская\""/RConn3 -- bus320/LConn1
  "T_434906029_110000_ПС_\"Комбайновый_завод\""/RConn1 -- L_434906029/LConn1
  "T_434906029_110000_ПС_\"Комбайновый_завод\""/RConn2 -- L_434906029/LConn2
  L_434906029/LConn3 -- "T_434906029_110000_ПС_\"Комбайновый_завод\""/RConn3 -- bus321/LConn1
  "T_258448640_110000;6000_ПС_№4_\"Городская\""/RConn1 -- L_258448640/LConn1
  "T_258448640_110000;6000_ПС_№4_\"Городская\""/RConn2 -- L_258448640/LConn2
  L_258448640/LConn3 -- "T_258448640_110000;6000_ПС_№4_\"Городская\""/RConn3 -- bus322/LConn1
  T_202917769_110000_Подстанция_«Сураново»/RConn1 -- L_202917769/LConn1
  T_202917769_110000_Подстанция_«Сураново»/RConn2 -- L_202917769/LConn2
  L_202917769/LConn3 -- T_202917769_110000_Подстанция_«Сураново»/RConn3 -- bus323/LConn1
  T_170223875_110000_Подстанция_«Межениновка»/RConn1 -- L_170223875/LConn1
  T_170223875_110000_Подстанция_«Межениновка»/RConn2 -- L_170223875/LConn2
  L_170223875/LConn3 -- T_170223875_110000_Подстанция_«Межениновка»/RConn3 -- bus324/LConn1
  T_162639659_110000_Подстанция_«71_км»/RConn1 -- L_162639659/LConn1
  T_162639659_110000_Подстанция_«71_км»/RConn2 -- L_162639659/LConn2
  L_162639659/LConn3 -- T_162639659_110000_Подстанция_«71_км»/RConn3 -- bus325/LConn1
  T_208031316__/RConn1 -- L_208031316/LConn1
  T_208031316__/RConn2 -- L_208031316/LConn2
  L_208031316/LConn3 -- T_208031316__/RConn3 -- bus326/LConn1
  T_221735143__/RConn1 -- L_221735143/LConn1
  T_221735143__/RConn2 -- L_221735143/LConn2
  L_221735143/LConn3 -- T_221735143__/RConn3 -- bus327/LConn1
  T_210955238__/RConn1 -- L_210955238/LConn1
  T_210955238__/RConn2 -- L_210955238/LConn2
  L_210955238/LConn3 -- T_210955238__/RConn3 -- bus328/LConn1
  "T_259523001_110000;6000_ПС_№25_\"РТИ\""/RConn1 -- L_259523001/LConn1
  "T_259523001_110000;6000_ПС_№25_\"РТИ\""/RConn2 -- L_259523001/LConn2
  L_259523001/LConn3 -- "T_259523001_110000;6000_ПС_№25_\"РТИ\""/RConn3 -- bus329/LConn1
  T_255181607_110000_/RConn1 -- L_255181607/LConn1
  T_255181607_110000_/RConn2 -- L_255181607/LConn2
  L_255181607/LConn3 -- T_255181607_110000_/RConn3 -- bus330/LConn1
  "T_254770727_110000;6000_ПС_№8_\"Цемзавод\""/RConn1 -- L_254770727/LConn1
  "T_254770727_110000;6000_ПС_№8_\"Цемзавод\""/RConn2 -- L_254770727/LConn2
  L_254770727/LConn3 -- "T_254770727_110000;6000_ПС_№8_\"Цемзавод\""/RConn3 -- bus331/LConn1
  "T_259526393_110000_ПС_№24_\"ЦБК\""/RConn1 -- L_259526393/LConn1
  "T_259526393_110000_ПС_№24_\"ЦБК\""/RConn2 -- L_259526393/LConn2
  L_259526393/LConn3 -- "T_259526393_110000_ПС_№24_\"ЦБК\""/RConn3 -- bus332/LConn1
  T_272521315__/RConn1 -- L_272521315/LConn1
  T_272521315__/RConn2 -- L_272521315/LConn2
  L_272521315/LConn3 -- T_272521315__/RConn3 -- bus333/LConn1
  T_170766446__/RConn1 -- L_170766446/LConn1
  T_170766446__/RConn2 -- L_170766446/LConn2
  L_170766446/LConn3 -- T_170766446__/RConn3 -- bus334/LConn1
  T_170766539__/RConn1 -- L_170766539/LConn1
  T_170766539__/RConn2 -- L_170766539/LConn2
  L_170766539/LConn3 -- T_170766539__/RConn3 -- bus335/LConn1
  T_141629072__/RConn1 -- L_141629072/LConn1
  T_141629072__/RConn2 -- L_141629072/LConn2
  L_141629072/LConn3 -- T_141629072__/RConn3 -- bus336/LConn1
  T_256577270__/RConn1 -- L_256577270/LConn1
  T_256577270__/RConn2 -- L_256577270/LConn2
  L_256577270/LConn3 -- T_256577270__/RConn3 -- bus337/LConn1
  T_227657047__/RConn1 -- L_227657047/LConn1
  T_227657047__/RConn2 -- L_227657047/LConn2
  L_227657047/LConn3 -- T_227657047__/RConn3 -- bus338/LConn1
  T_97113720_110000_Подстанция_«Малиновка»/RConn1 -- L_97113720/LConn1
  T_97113720_110000_Подстанция_«Малиновка»/RConn2 -- L_97113720/LConn2
  L_97113720/LConn3 -- T_97113720_110000_Подстанция_«Малиновка»/RConn3 -- bus339/LConn1
  T_181309204_110000_Подстанция_«Турунтаево»/RConn1 -- L_181309204/LConn1
  T_181309204_110000_Подстанция_«Турунтаево»/RConn2 -- L_181309204/LConn2
  L_181309204/LConn3 -- T_181309204_110000_Подстанция_«Турунтаево»/RConn3 -- bus340/LConn1
  T_125746756_110000_Подстанция_«Бройлерная»/RConn1 -- L_125746756/LConn1
  T_125746756_110000_Подстанция_«Бройлерная»/RConn2 -- L_125746756/LConn2
  L_125746756/LConn3 -- T_125746756_110000_Подстанция_«Бройлерная»/RConn3 -- bus341/LConn1
  T_97113734_110000_Подстанция_«Итатка»/RConn1 -- L_97113734/LConn1
  T_97113734_110000_Подстанция_«Итатка»/RConn2 -- L_97113734/LConn2
  L_97113734/LConn3 -- T_97113734_110000_Подстанция_«Итатка»/RConn3 -- bus342/LConn1
  T_171057519_110000_Подстанция_«Парабель_КС»/RConn1 -- L_171057519/LConn1
  T_171057519_110000_Подстанция_«Парабель_КС»/RConn2 -- L_171057519/LConn2
  L_171057519/LConn3 -- T_171057519_110000_Подстанция_«Парабель_КС»/RConn3 -- bus343/LConn1
  T_197782305_110000_Подстанция_«Лугинецкая»/RConn1 -- L_197782305/LConn1
  T_197782305_110000_Подстанция_«Лугинецкая»/RConn2 -- L_197782305/LConn2
  L_197782305/LConn3 -- T_197782305_110000_Подстанция_«Лугинецкая»/RConn3 -- bus344/LConn1
  T_169734094_110000_Подстанция_«Асино_110»/RConn1 -- L_169734094/LConn1
  T_169734094_110000_Подстанция_«Асино_110»/RConn2 -- L_169734094/LConn2
  L_169734094/LConn3 -- T_169734094_110000_Подстанция_«Асино_110»/RConn3 -- bus345/LConn1
  T_145227914__Подстанция_«Учительская»/RConn1 -- L_145227914/LConn1
  T_145227914__Подстанция_«Учительская»/RConn2 -- L_145227914/LConn2
  L_145227914/LConn3 -- T_145227914__Подстанция_«Учительская»/RConn3 -- bus346/LConn1
  T_170936087_110000_Подстанция_«Колпашево»/RConn1 -- L_170936087/LConn1
  T_170936087_110000_Подстанция_«Колпашево»/RConn2 -- L_170936087/LConn2
  L_170936087/LConn3 -- T_170936087_110000_Подстанция_«Колпашево»/RConn3 -- bus347/LConn1
  "T_289000622_110000;10000_ПC_№16_\"Пролетарская\""/RConn1 -- L_289000622/LConn1
  "T_289000622_110000;10000_ПC_№16_\"Пролетарская\""/RConn2 -- L_289000622/LConn2
  L_289000622/LConn3 -- "T_289000622_110000;10000_ПC_№16_\"Пролетарская\""/RConn3 -- bus348/LConn1
  T_173502610_110000_Подстанция_«Усть_Бакчар»/RConn1 -- L_173502610/LConn1
  T_173502610_110000_Подстанция_«Усть_Бакчар»/RConn2 -- L_173502610/LConn2
  L_173502610/LConn3 -- T_173502610_110000_Подстанция_«Усть_Бакчар»/RConn3 -- bus349/LConn1
  T_170480403_110000_Подстанция_«Высокий_Яр»/RConn1 -- L_170480403/LConn1
  T_170480403_110000_Подстанция_«Высокий_Яр»/RConn2 -- L_170480403/LConn2
  L_170480403/LConn3 -- T_170480403_110000_Подстанция_«Высокий_Яр»/RConn3 -- bus350/LConn1
  T_169815706_110000_Подстанция_«Молчаново»/RConn1 -- L_169815706/LConn1
  T_169815706_110000_Подстанция_«Молчаново»/RConn2 -- L_169815706/LConn2
  L_169815706/LConn3 -- T_169815706_110000_Подстанция_«Молчаново»/RConn3 -- bus351/LConn1
  T_191567780_110000_Подстанция_«Коломинские_Гривы»/RConn1 -- L_191567780/LConn1
  T_191567780_110000_Подстанция_«Коломинские_Гривы»/RConn2 -- L_191567780/LConn2
  L_191567780/LConn3 -- T_191567780_110000_Подстанция_«Коломинские_Гривы»/RConn3 -- bus352/LConn1
  T_172669169_110000_Подстанция_«Молчановская_НПС»/RConn1 -- L_172669169/LConn1
  T_172669169_110000_Подстанция_«Молчановская_НПС»/RConn2 -- L_172669169/LConn2
  L_172669169/LConn3 -- T_172669169_110000_Подстанция_«Молчановская_НПС»/RConn3 -- bus353/LConn1
  T_172669881_110000_Подстанция_«Тунгусово»/RConn1 -- L_172669881/LConn1
  T_172669881_110000_Подстанция_«Тунгусово»/RConn2 -- L_172669881/LConn2
  L_172669881/LConn3 -- T_172669881_110000_Подстанция_«Тунгусово»/RConn3 -- bus354/LConn1
  T_198009967__/RConn1 -- L_198009967/LConn1
  T_198009967__/RConn2 -- L_198009967/LConn2
  L_198009967/LConn3 -- T_198009967__/RConn3 -- bus355/LConn1
  T_198008863__/RConn1 -- L_198008863/LConn1
  T_198008863__/RConn2 -- L_198008863/LConn2
  L_198008863/LConn3 -- T_198008863__/RConn3 -- bus356/LConn1
  "T_126390946__ПС_\"Сыропятское\""/RConn1 -- L_126390946/LConn1
  "T_126390946__ПС_\"Сыропятское\""/RConn2 -- L_126390946/LConn2
  L_126390946/LConn3 -- "T_126390946__ПС_\"Сыропятское\""/RConn3 -- bus357/LConn1
  "T_230915624__Тяговая_подстанция_\"Чугунаш\""/RConn1 -- L_230915624/LConn1
  "T_230915624__Тяговая_подстанция_\"Чугунаш\""/RConn2 -- L_230915624/LConn2
  L_230915624/LConn3 -- "T_230915624__Тяговая_подстанция_\"Чугунаш\""/RConn3 -- bus358/LConn1
  "T_225625506_110000;35000;6000_ПС_110_35_6_кВ_\"Кондомская\""/RConn1 -- L_225625506/LConn1
  "T_225625506_110000;35000;6000_ПС_110_35_6_кВ_\"Кондомская\""/RConn2 -- L_225625506/LConn2
  L_225625506/LConn3 -- "T_225625506_110000;35000;6000_ПС_110_35_6_кВ_\"Кондомская\""/RConn3 -- bus359/LConn1
  T_312889001_110000;6000_ПС_БНС_ТЭЦ_3/RConn1 -- L_312889001/LConn1
  T_312889001_110000;6000_ПС_БНС_ТЭЦ_3/RConn2 -- L_312889001/LConn2
  L_312889001/LConn3 -- T_312889001_110000;6000_ПС_БНС_ТЭЦ_3/RConn3 -- bus360/LConn1
  "T_313033143_110000;10000_ПС_№147_\"Речпорт\""/RConn1 -- L_313033143/LConn1
  "T_313033143_110000;10000_ПС_№147_\"Речпорт\""/RConn2 -- L_313033143/LConn2
  L_313033143/LConn3 -- "T_313033143_110000;10000_ПС_№147_\"Речпорт\""/RConn3 -- bus361/LConn1
  "T_60450100_220000;110000_ПС_\"КИСК\""/RConn1 -- L_60450100/LConn1
  "T_60450100_220000;110000_ПС_\"КИСК\""/RConn2 -- L_60450100/LConn2
  L_60450100/LConn3 -- "T_60450100_220000;110000_ПС_\"КИСК\""/RConn3 -- bus362/LConn1
  "T_285451553_110000;10000_ПС_№134_\"Солонцы\""/RConn1 -- L_285451553/LConn1
  "T_285451553_110000;10000_ПС_№134_\"Солонцы\""/RConn2 -- L_285451553/LConn2
  L_285451553/LConn3 -- "T_285451553_110000;10000_ПС_№134_\"Солонцы\""/RConn3 -- bus363/LConn1
  "T_202168530_110000;10000_ПС_\"Слобода_весны\""/RConn1 -- L_202168530/LConn1
  "T_202168530_110000;10000_ПС_\"Слобода_весны\""/RConn2 -- L_202168530/LConn2
  L_202168530/LConn3 -- "T_202168530_110000;10000_ПС_\"Слобода_весны\""/RConn3 -- bus364/LConn1
  "T_202168527_110000;10000_ПС_№71_\"Весна\""/RConn1 -- L_202168527/LConn1
  "T_202168527_110000;10000_ПС_№71_\"Весна\""/RConn2 -- L_202168527/LConn2
  L_202168527/LConn3 -- "T_202168527_110000;10000_ПС_№71_\"Весна\""/RConn3 -- bus365/LConn1
  T_162577702__ПС_СХК/RConn1 -- L_162577702/LConn1
  T_162577702__ПС_СХК/RConn2 -- L_162577702/LConn2
  L_162577702/LConn3 -- T_162577702__ПС_СХК/RConn3 -- bus366/LConn1
  T_149712234_110000_Подстанция_«Пиковая»/RConn1 -- L_149712234/LConn1
  T_149712234_110000_Подстанция_«Пиковая»/RConn2 -- L_149712234/LConn2
  L_149712234/LConn3 -- T_149712234_110000_Подстанция_«Пиковая»/RConn3 -- bus367/LConn1
  "T_107196366__ГПП_1_\"Первая_Городская\""/RConn1 -- L_107196366/LConn1
  "T_107196366__ГПП_1_\"Первая_Городская\""/RConn2 -- L_107196366/LConn2
  L_107196366/LConn3 -- "T_107196366__ГПП_1_\"Первая_Городская\""/RConn3 -- bus368/LConn1
  T_274464446__/RConn1 -- L_274464446/LConn1
  T_274464446__/RConn2 -- L_274464446/LConn2
  L_274464446/LConn3 -- T_274464446__/RConn3 -- bus369/LConn1
  T_289973452__/RConn1 -- L_289973452/LConn1
  T_289973452__/RConn2 -- L_289973452/LConn2
  L_289973452/LConn3 -- T_289973452__/RConn3 -- bus370/LConn1
  T_190450368_110000_Подстанция_«Григорьевская»/RConn1 -- L_190450368/LConn1
  T_190450368_110000_Подстанция_«Григорьевская»/RConn2 -- L_190450368/LConn2
  L_190450368/LConn3 -- T_190450368_110000_Подстанция_«Григорьевская»/RConn3 -- bus371/LConn1
  T_89555905_110000_Подстанция_«Стрежевская»/RConn1 -- L_89555905/LConn1
  T_89555905_110000_Подстанция_«Стрежевская»/RConn2 -- L_89555905/LConn2
  L_89555905/LConn3 -- T_89555905_110000_Подстанция_«Стрежевская»/RConn3 -- bus372/LConn1
  T_316964474__/RConn1 -- L_316964474/LConn1
  T_316964474__/RConn2 -- L_316964474/LConn2
  L_316964474/LConn3 -- T_316964474__/RConn3 -- bus373/LConn1
  T_169700760_110000_Подстанция_«Чажемто_110»/RConn1 -- L_169700760/LConn1
  T_169700760_110000_Подстанция_«Чажемто_110»/RConn2 -- L_169700760/LConn2
  L_169700760/LConn3 -- T_169700760_110000_Подстанция_«Чажемто_110»/RConn3 -- bus374/LConn1
  T_134436050_110000_Подстанция_«Малореченская»/RConn1 -- L_134436050/LConn1
  T_134436050_110000_Подстанция_«Малореченская»/RConn2 -- L_134436050/LConn2
  L_134436050/LConn3 -- T_134436050_110000_Подстанция_«Малореченская»/RConn3 -- bus375/LConn1
  T_130469640_110000_ПС_«Александровская»_110_10/RConn1 -- L_130469640/LConn1
  T_130469640_110000_ПС_«Александровская»_110_10/RConn2 -- L_130469640/LConn2
  L_130469640/LConn3 -- T_130469640_110000_ПС_«Александровская»_110_10/RConn3 -- bus376/LConn1
  T_245392698_110000_Подстанция_«Чердаты»/RConn1 -- L_245392698/LConn1
  T_245392698_110000_Подстанция_«Чердаты»/RConn2 -- L_245392698/LConn2
  L_245392698/LConn3 -- T_245392698_110000_Подстанция_«Чердаты»/RConn3 -- bus377/LConn1
  T_243298567_110000_Подстанция_«Зырянка»/RConn1 -- L_243298567/LConn1
  T_243298567_110000_Подстанция_«Зырянка»/RConn2 -- L_243298567/LConn2
  L_243298567/LConn3 -- T_243298567_110000_Подстанция_«Зырянка»/RConn3 -- bus378/LConn1
  T_100146904_110000_Подстанция_«Зубковская»/RConn1 -- L_100146904/LConn1
  T_100146904_110000_Подстанция_«Зубковская»/RConn2 -- L_100146904/LConn2
  L_100146904/LConn3 -- T_100146904_110000_Подстанция_«Зубковская»/RConn3 -- bus379/LConn1
  T_201600388_110000_Подстанция_«Веселовская»/RConn1 -- L_201600388/LConn1
  T_201600388_110000_Подстанция_«Веселовская»/RConn2 -- L_201600388/LConn2
  L_201600388/LConn3 -- T_201600388_110000_Подстанция_«Веселовская»/RConn3 -- bus380/LConn1
  T_100118265_110000_Подстанция_«Нива»/RConn1 -- L_100118265/LConn1
  T_100118265_110000_Подстанция_«Нива»/RConn2 -- L_100118265/LConn2
  L_100118265/LConn3 -- T_100118265_110000_Подстанция_«Нива»/RConn3 -- bus381/LConn1
  T_201600393_110000_Подстанция_«Лянино»/RConn1 -- L_201600393/LConn1
  T_201600393_110000_Подстанция_«Лянино»/RConn2 -- L_201600393/LConn2
  L_201600393/LConn3 -- T_201600393_110000_Подстанция_«Лянино»/RConn3 -- bus382/LConn1
  T_374528071__/RConn1 -- L_374528071/LConn1
  T_374528071__/RConn2 -- L_374528071/LConn2
  L_374528071/LConn3 -- T_374528071__/RConn3 -- bus383/LConn1
  T_176748969__/RConn1 -- L_176748969/LConn1
  T_176748969__/RConn2 -- L_176748969/LConn2
  L_176748969/LConn3 -- T_176748969__/RConn3 -- bus384/LConn1
  T_223867037__/RConn1 -- L_223867037/LConn1
  T_223867037__/RConn2 -- L_223867037/LConn2
  L_223867037/LConn3 -- T_223867037__/RConn3 -- bus385/LConn1
  T_191079379_110000_Подстанция_110_35_10_кВ_«ОЭЗ»/RConn1 -- L_191079379/LConn1
  T_191079379_110000_Подстанция_110_35_10_кВ_«ОЭЗ»/RConn2 -- L_191079379/LConn2
  L_191079379/LConn3 -- T_191079379_110000_Подстанция_110_35_10_кВ_«ОЭЗ»/RConn3 -- bus386/LConn1
  T_192046328__/RConn1 -- L_192046328/LConn1
  T_192046328__/RConn2 -- L_192046328/LConn2
  L_192046328/LConn3 -- T_192046328__/RConn3 -- bus387/LConn1
  T_169996149_110000_Подстанция_«Кандинка_110»/RConn1 -- L_169996149/LConn1
  T_169996149_110000_Подстанция_«Кандинка_110»/RConn2 -- L_169996149/LConn2
  L_169996149/LConn3 -- T_169996149_110000_Подстанция_«Кандинка_110»/RConn3 -- bus388/LConn1
  "T_267632930_110000_ПС_№7_\"Медпрепараты\""/RConn1 -- L_267632930/LConn1
  "T_267632930_110000_ПС_№7_\"Медпрепараты\""/RConn2 -- L_267632930/LConn2
  L_267632930/LConn3 -- "T_267632930_110000_ПС_№7_\"Медпрепараты\""/RConn3 -- bus389/LConn1
  "T_275667154_110000;35000;6000_ПС_№92_\"Юго_Западная\""/RConn1 -- L_275667154/LConn1
  "T_275667154_110000;35000;6000_ПС_№92_\"Юго_Западная\""/RConn2 -- L_275667154/LConn2
  L_275667154/LConn3 -- "T_275667154_110000;35000;6000_ПС_№92_\"Юго_Западная\""/RConn3 -- bus390/LConn1
  "T_279030763_110000;6000_ПС_№65_\"Бобровый_лог\""/RConn1 -- L_279030763/LConn1
  "T_279030763_110000;6000_ПС_№65_\"Бобровый_лог\""/RConn2 -- L_279030763/LConn2
  L_279030763/LConn3 -- "T_279030763_110000;6000_ПС_№65_\"Бобровый_лог\""/RConn3 -- bus391/LConn1
  T_130482986_110000_Подстанция_«Раздольное»/RConn1 -- L_130482986/LConn1
  T_130482986_110000_Подстанция_«Раздольное»/RConn2 -- L_130482986/LConn2
  L_130482986/LConn3 -- T_130482986_110000_Подстанция_«Раздольное»/RConn3 -- bus392/LConn1
  T_219125213_110000_Подстанция_«Тегульдет»/RConn1 -- L_219125213/LConn1
  T_219125213_110000_Подстанция_«Тегульдет»/RConn2 -- L_219125213/LConn2
  L_219125213/LConn3 -- T_219125213_110000_Подстанция_«Тегульдет»/RConn3 -- bus393/LConn1
  "T_295819200_110000;10000_ПС_№49_\"Юбилейная\""/RConn1 -- L_295819200/LConn1
  "T_295819200_110000;10000_ПС_№49_\"Юбилейная\""/RConn2 -- L_295819200/LConn2
  L_295819200/LConn3 -- "T_295819200_110000;10000_ПС_№49_\"Юбилейная\""/RConn3 -- bus394/LConn1
  T_194903352_110000_Подстанция_«Калиновая»/RConn1 -- L_194903352/LConn1
  T_194903352_110000_Подстанция_«Калиновая»/RConn2 -- L_194903352/LConn2
  L_194903352/LConn3 -- T_194903352_110000_Подстанция_«Калиновая»/RConn3 -- bus395/LConn1
